simulink model "COMPONENT_MDL_Lag_QUAD_and_PEND_with_spin_rotors"  (R2020b)
(part 9 of 10)

Ly_pend.^2.*THE_Phi_D.*m_pend.*sin(THE_Phi_pend.*2.0).*(-1.0./2.4e+1)+(Lz_pend.^2.*THE_Phi_D.*m_pend.*sin(THE_Phi_pend.*2.0))./6.0-(Ly_pend.^2.*THE_Psi_D.*m_pend.*cos(THE_Theta).*sin(THE_Psi))./6.0-(Ly_pend.^2.*THE_Theta_pend_D.*m_pend.*cos(THE_Phi_pend).*sin(THE_Theta))./6.0-Lz_pend.^2.*THE_Theta_D.*m_pend.*cos(THE_Psi).*sin(THE_Theta).*(2.0./3.0)+(Ly_pend.^2.*THE_Phi_D.*m_pend.*cos(THE_Theta).*sin(THE_Psi).*sin(THE_Theta))./1.2e+1+(Ly_pend.^2.*THE_Psi_D.*m_pend.*cos(THE_Phi_pend).*sin(THE_Theta).*sin(THE_Phi_pend))./6.0+(Ly_pend.^2.*THE_Theta_pend_D.*m_pend.*cos(THE_Theta).*sin(THE_Psi).*sin(THE_Phi_pend))./6.0+(Ly_pend.^2.*THE_Phi_D.*m_pend.*cos(THE_Psi_pend).*sin(THE_Psi_pend).*sin(THE_Theta_pend))./1.2e+1-(Lz_pend.^2.*THE_Phi_D.*m_pend.*cos(THE_Theta).*sin(THE_Psi).*sin(THE_Theta))./3.0-Lz_pend.^2.*THE_Psi_D.*m_pend.*cos(THE_Phi_pend).*sin(THE_Theta).*sin(THE_Phi_pend).*(2.0./3.0)-(Lz_pend.^2.*THE_Phi_D.*m_pend.*cos(THE_Psi_pend).*sin(THE_Psi_pend).*sin(THE_Theta_pend))./3.0-Lz_pend.^2.*THE_Psi_pend_D.*m_pend.*cos(THE_Theta_pend).*sin(THE_Theta).*sin(THE_Phi_pend).*(2.0./3.0)-(Lx_pend.^2.*THE_Psi_D.*m_pend.*cos(THE_Theta).*cos(THE_Theta_pend).^2.*sin(THE_Psi))./6.0-(Lx_pend.^2.*THE_Phi_D.*m_pend.*cos(THE_Phi_pend).*cos(THE_Theta_pend).^2.*sin(THE_Phi_pend))./1.2e+1-(Lx_pend.^2.*THE_Theta_pend_D.*m_pend.*cos(THE_Phi_pend).*cos(THE_Theta_pend).^2.*sin(THE_Theta))./6.0+(Ly_pend.^2.*THE_Psi_D.*m_pend.*cos(THE_Theta).*cos(THE_Phi_pend).^2.*sin(THE_Psi))./6.0+(Ly_pend.^2.*THE_Psi_D.*m_pend.*cos(THE_Theta).*cos(THE_Psi_pend).^2.*sin(THE_Psi))./6.0-(Ly_pend.^2.*THE_Theta_D.*m_pend.*cos(THE_Psi).*cos(THE_Phi_pend).^2.*sin(THE_Theta))./6.0+(Ly_pend.^2.*THE_Psi_D.*m_pend.*cos(THE_Theta).*cos(THE_Theta_pend).^2.*sin(THE_Psi))./6.0-(Ly_pend.^2.*THE_Theta_D.*m_pend.*cos(THE_Psi).*cos(THE_Psi_pend).^2.*sin(THE_Theta))./6.0+(Ly_pend.^2.*THE_Phi_D.*m_pend.*cos(THE_Theta).^2.*cos(THE_Phi_pend).*sin(THE_Phi_pend))./6.0+(Ly_pend.^2.*THE_Phi_D.*m_pend.*cos(THE_Phi_pend).*cos(THE_Psi_pend).^2.*sin(THE_Phi_pend))./6.0+(Ly_pend.^2.*THE_Phi_D.*m_pend.*cos(THE_Phi_pend).*cos(THE_Theta_pend).^2.*sin(THE_Phi_pend))./1.2e+1+(Ly_pend.^2.*THE_Theta_pend_D.*m_pend.*cos(THE_Phi_pend).*cos(THE_Psi_pend).^2.*sin(THE_Theta))./6.0+(Ly_pend.^2.*THE_Theta_pend_D.*m_pend.*cos(THE_Phi_pend).*cos(THE_Theta_pend).^2.*sin(THE_Theta))./6.0-Lz_pend.^2.*THE_Psi_D.*m_pend.*cos(THE_Theta).*cos(THE_Phi_pend).^2.*sin(THE_Psi).*(2.0./3.0)-Lz_pend.^2.*THE_Psi_D.*m_pend.*cos(THE_Theta).*cos(THE_Psi_pend).^2.*sin(THE_Psi).*(2.0./3.0)+Lz_pend.^2.*THE_Theta_D.*m_pend.*cos(THE_Psi).*cos(THE_Phi_pend).^2.*sin(THE_Theta).*(2.0./3.0)+Lz_pend.^2.*THE_Theta_D.*m_pend.*cos(THE_Psi).*cos(THE_Psi_pend).^2.*sin(THE_Theta).*(2.0./3.0)-Lz_pend.^2.*THE_Phi_D.*m_pend.*cos(THE_Theta).^2.*cos(THE_Phi_pend).*sin(THE_Phi_pend).*(2.0./3.0)-Lz_pend.^2.*THE_Phi_D.*m_pend.*cos(THE_Phi_pend).*cos(THE_Psi_pend).^2.*sin(THE_Phi_pend).*(2.0./3.0)-Lz_pend.^2.*THE_Theta_pend_D.*m_pend.*cos(THE_Phi_pend).*cos(THE_Psi_pend).^2.*sin(THE_Theta).*(2.0./3.0)+(Lx_pend.^2.*THE_Phi_D.*m_pend.*cos(THE_Theta).*cos(THE_Theta_pend).^2.*sin(THE_Psi).*sin(THE_Theta))./1.2e+1+(Lx_pend.^2.*THE_Psi_D.*m_pend.*cos(THE_Phi_pend).*cos(THE_Theta_pend).^2.*sin(THE_Theta).*sin(THE_Phi_pend))./6.0+(Lx_pend.^2.*THE_Theta_pend_D.*m_pend.*cos(THE_Theta).*cos(THE_Theta_pend).^2.*sin(THE_Psi).*sin(THE_Phi_pend))./6.0-(Ly_pend.^2.*THE_Phi_D.*m_pend.*cos(THE_Theta).*cos(THE_Phi_pend).^2.*sin(THE_Psi).*sin(THE_Theta))./6.0-(Ly_pend.^2.*THE_Phi_D.*m_pend.*cos(THE_Theta).*cos(THE_Psi_pend).^2.*sin(THE_Psi).*sin(THE_Theta))./6.0-(Ly_pend.^2.*THE_Phi_D.*m_pend.*cos(THE_Theta).*cos(THE_Theta_pend).^2.*sin(THE_Psi).*sin(THE_Theta))./1.2e+1-(Ly_pend.^2.*THE_Psi_D.*m_pend.*cos(THE_Phi_pend).*cos(THE_Psi_pend).^2.*sin(THE_Theta).*sin(THE_Phi_pend))./3.0-(Ly_pend.^2.*THE_Psi_D.*m_pend.*cos(THE_Phi_pend).*cos(THE_Theta_pend).^2.*sin(THE_Theta).*sin(THE_Phi_pend))./6.0-(Ly_pend.^2.*THE_Phi_D.*m_pend.*cos(THE_Theta).^2.*cos(THE_Psi_pend).*sin(THE_Psi_pend).*sin(THE_Theta_pend))./6.0-(Ly_pend.^2.*THE_Theta_pend_D.*m_pend.*cos(THE_Theta).*cos(THE_Psi_pend).^2.*sin(THE_Psi).*sin(THE_Phi_pend))./6.0-(Ly_pend.^2.*THE_Theta_pend_D.*m_pend.*cos(THE_Theta).*cos(THE_Theta_pend).^2.*sin(THE_Psi).*sin(THE_Phi_pend))./6.0-(Ly_pend.^2.*THE_Phi_D.*m_pend.*cos(THE_Phi_pend).^2.*cos(THE_Psi_pend).*sin(THE_Psi_pend).*sin(THE_Theta_pend))./6.0-(Ly_pend.^2.*THE_Psi_pend_D.*m_pend.*cos(THE_Psi_pend).^2.*cos(THE_Theta_pend).*sin(THE_Theta).*sin(THE_Phi_pend))./6.0+Lz_pend.^2.*THE_Phi_D.*m_pend.*cos(THE_Theta).*cos(THE_Phi_pend).^2.*sin(THE_Psi).*sin(THE_Theta).*(2.0./3.0)+Lz_pend.^2.*THE_Phi_D.*m_pend.*cos(THE_Theta).*cos(THE_Psi_pend).^2.*sin(THE_Psi).*sin(THE_Theta).*(2.0./3.0)+Lz_pend.^2.*THE_Psi_D.*m_pend.*cos(THE_Phi_pend).*cos(THE_Psi_pend).^2.*sin(THE_Theta).*sin(THE_Phi_pend).*(4.0./3.0)+Lz_pend.^2.*THE_Phi_D.*m_pend.*cos(THE_Theta).^2.*cos(THE_Psi_pend).*sin(THE_Psi_pend).*sin(THE_Theta_pend).*(2.0./3.0)+Lz_pend.^2.*THE_Theta_pend_D.*m_pend.*cos(THE_Theta).*cos(THE_Psi_pend).^2.*sin(THE_Psi).*sin(THE_Phi_pend).*(2.0./3.0)+Lz_pend.^2.*THE_Phi_D.*m_pend.*cos(THE_Phi_pend).^2.*cos(THE_Psi_pend).*sin(THE_Psi_pend).*sin(THE_Theta_pend).*(2.0./3.0)+Lz_pend.^2.*THE_Psi_pend_D.*m_pend.*cos(THE_Psi_pend).^2.*cos(THE_Theta_pend).*sin(THE_Theta).*sin(THE_Phi_pend).*(2.0./3.0)+(Lx_pend.^2.*THE_Psi_D.*m_pend.*cos(THE_Theta).*cos(THE_Phi_pend).^2.*cos(THE_Theta_pend).^2.*sin(THE_Psi))./6.0-(Lx_pend.^2.*THE_Theta_D.*m_pend.*cos(THE_Psi).*cos(THE_Phi_pend).^2.*cos(THE_Theta_pend).^2.*sin(THE_Theta))./6.0+(Lx_pend.^2.*THE_Phi_D.*m_pend.*cos(THE_Theta).^2.*cos(THE_Phi_pend).*cos(THE_Theta_pend).^2.*sin(THE_Phi_pend))./6.0-(Ly_pend.^2.*THE_Phi_D.*m_pend.*cos(THE_Psi).^2.*cos(THE_Theta).^2.*cos(THE_Phi_pend).*sin(THE_Phi_pend))./1.2e+1-(Ly_pend.^2.*THE_Psi_D.*m_pend.*cos(THE_Theta).*cos(THE_Phi_pend).^2.*cos(THE_Psi_pend).^2.*sin(THE_Psi))./3.0-(Ly_pend.^2.*THE_Psi_D.*m_pend.*cos(THE_Theta).*cos(THE_Phi_pend).^2.*cos(THE_Theta_pend).^2.*sin(THE_Psi))./6.0+(Ly_pend.^2.*THE_Theta_D.*m_pend.*cos(THE_Psi).*cos(THE_Phi_pend).^2.*cos(THE_Psi_pend).^2.*sin(THE_Theta))./3.0-(Ly_pend.^2.*THE_Psi_D.*m_pend.*cos(THE_Theta).*cos(THE_Psi_pend).^2.*cos(THE_Theta_pend).^2.*sin(THE_Psi))./6.0+(Ly_pend.^2.*THE_Theta_D.*m_pend.*cos(THE_Psi).*cos(THE_Phi_pend).^2.*cos(THE_Theta_pend).^2.*sin(THE_Theta))./6.0-(Ly_pend.^2.*THE_Phi_D.*m_pend.*cos(THE_Theta).^2.*cos(THE_Phi_pend).*cos(THE_Psi_pend).^2.*sin(THE_Phi_pend))./3.0-(Ly_pend.^2.*THE_Phi_D.*m_pend.*cos(THE_Theta).^2.*cos(THE_Phi_pend).*cos(THE_Theta_pend).^2.*sin(THE_Phi_pend))./6.0-(Ly_pend.^2.*THE_Phi_D.*m_pend.*cos(THE_Phi_pend).*cos(THE_Psi_pend).^2.*cos(THE_Theta_pend).^2.*sin(THE_Phi_pend))./1.2e+1-(Ly_pend.^2.*THE_Theta_pend_D.*m_pend.*cos(THE_Phi_pend).*cos(THE_Psi_pend).^2.*cos(THE_Theta_pend).^2.*sin(THE_Theta))./6.0+(Lz_pend.^2.*THE_Phi_D.*m_pend.*cos(THE_Psi).^2.*cos(THE_Theta).^2.*cos(THE_Phi_pend).*sin(THE_Phi_pend))./3.0+Lz_pend.^2.*THE_Psi_D.*m_pend.*cos(THE_Theta).*cos(THE_Phi_pend).^2.*cos(THE_Psi_pend).^2.*sin(THE_Psi).*(4.0./3.0)-Lz_pend.^2.*THE_Theta_D.*m_pend.*cos(THE_Psi).*cos(THE_Phi_pend).^2.*cos(THE_Psi_pend).^2.*sin(THE_Theta).*(4.0./3.0)+Lz_pend.^2.*THE_Psi_D.*m_pend.*cos(THE_Theta).*cos(THE_Psi_pend).^2.*cos(THE_Theta_pend).^2.*sin(THE_Psi).*(2.0./3.0)+Lz_pend.^2.*THE_Phi_D.*m_pend.*cos(THE_Theta).^2.*cos(THE_Phi_pend).*cos(THE_Psi_pend).^2.*sin(THE_Phi_pend).*(4.0./3.0)+(Lz_pend.^2.*THE_Phi_D.*m_pend.*cos(THE_Phi_pend).*cos(THE_Psi_pend).^2.*cos(THE_Theta_pend).^2.*sin(THE_Phi_pend))./3.0+Lz_pend.^2.*THE_Theta_pend_D.*m_pend.*cos(THE_Phi_pend).*cos(THE_Psi_pend).^2.*cos(THE_Theta_pend).^2.*sin(THE_Theta).*(2.0./3.0)-(Lx_pend.^2.*THE_Theta_pend_D.*m_pend.*cos(THE_Psi).*cos(THE_Theta).*cos(THE_Theta_pend).*sin(THE_Theta_pend))./6.0+(Ly_pend.^2.*THE_Theta_pend_D.*m_pend.*cos(THE_Psi).*cos(THE_Theta).*cos(THE_Theta_pend).*sin(THE_Theta_pend))./6.0-Lz_pend.^2.*THE_Psi_pend_D.*m_pend.*cos(THE_Theta).*cos(THE_Phi_pend).*cos(THE_Theta_pend).*sin(THE_Psi).*(2.0./3.0)-(Ly_pend.^2.*THE_Psi_D.*m_pend.*cos(THE_Psi_pend).*sin(THE_Theta).*sin(THE_Psi_pend).*sin(THE_Theta_pend))./6.0+Lz_pend.^2.*THE_Psi_D.*m_pend.*cos(THE_Psi_pend).*sin(THE_Theta).*sin(THE_Psi_pend).*sin(THE_Theta_pend).*(2.0./3.0)+Lz_pend.*THE_Theta_D.*Tv_Z_pend.*m_pend.*cos(THE_Psi).^2.*cos(THE_Theta).*sin(THE_Phi_pend).*sin(THE_Psi_pend)-(Lx_pend.^2.*THE_Phi_D.*m_pend.*cos(THE_Theta).*cos(THE_Phi_pend).^2.*cos(THE_Theta_pend).^2.*sin(THE_Psi).*sin(THE_Theta))./6.0+(Ly_pend.^2.*THE_Phi_D.*m_pend.*cos(THE_Theta).*cos(THE_Phi_pend).^2.*cos(THE_Psi_pend).^2.*sin(THE_Psi).*sin(THE_Theta))./3.0+(Ly_pend.^2.*THE_Phi_D.*m_pend.*cos(THE_Theta).*cos(THE_Phi_pend).^2.*cos(THE_Theta_pend).^2.*sin(THE_Psi).*sin(THE_Theta))./6.0+(Ly_pend.^2.*THE_Phi_D.*m_pend.*cos(THE_Theta).*cos(THE_Psi_pend).^2.*cos(THE_Theta_pend).^2.*sin(THE_Psi).*sin(THE_Theta))./1.2e+1+(Ly_pend.^2.*THE_Phi_D.*m_pend.*cos(THE_Psi).^2.*cos(THE_Theta).^2.*cos(THE_Psi_pend).*sin(THE_Psi_pend).*sin(THE_Theta_pend))./1.2e+1+(Ly_pend.^2.*THE_Phi_D.*m_pend.*cos(THE_Theta).^2.*cos(THE_Phi_pend).^2.*cos(THE_Psi_pend).*sin(THE_Psi_pend).*sin(THE_Theta_pend))./3.0+(Ly_pend.^2.*THE_Psi_D.*m_pend.*cos(THE_Phi_pend).*cos(THE_Psi_pend).^2.*cos(THE_Theta_pend).^2.*sin(THE_Theta).*sin(THE_Phi_pend))./6.0+(Ly_pend.^2.*THE_Theta_pend_D.*m_pend.*cos(THE_Theta).*cos(THE_Psi_pend).^2.*cos(THE_Theta_pend).^2.*sin(THE_Psi).*sin(THE_Phi_pend))./6.0-Lz_pend.^2.*THE_Phi_D.*m_pend.*cos(THE_Theta).*cos(THE_Phi_pend).^2.*cos(THE_Psi_pend).^2.*sin(THE_Psi).*sin(THE_Theta).*(4.0./3.0)-(Lz_pend.^2.*THE_Phi_D.*m_pend.*cos(THE_Theta).*cos(THE_Psi_pend).^2.*cos(THE_Theta_pend).^2.*sin(THE_Psi).*sin(THE_Theta))./3.0-(Lz_pend.^2.*THE_Phi_D.*m_pend.*cos(THE_Psi).^2.*cos(THE_Theta).^2.*cos(THE_Psi_pend).*sin(THE_Psi_pend).*sin(THE_Theta_pend))./3.0-Lz_pend.^2.*THE_Phi_D.*m_pend.*cos(THE_Theta).^2.*cos(THE_Phi_pend).^2.*cos(THE_Psi_pend).*sin(THE_Psi_pend).*sin(THE_Theta_pend).*(4.0./3.0)-Lz_pend.^2.*THE_Psi_D.*m_pend.*cos(THE_Phi_pend).*cos(THE_Psi_pend).^2.*cos(THE_Theta_pend).^2.*sin(THE_Theta).*sin(THE_Phi_pend).*(2.0./3.0)-Lz_pend.^2.*THE_Theta_pend_D.*m_pend.*cos(THE_Theta).*cos(THE_Psi_pend).^2.*cos(THE_Theta_pend).^2.*sin(THE_Psi).*sin(THE_Phi_pend).*(2.0./3.0)+(Lx_pend.^2.*THE_Psi_D.*m_pend.*cos(THE_Psi).*cos(THE_Theta).*cos(THE_Theta_pend).*sin(THE_Phi_pend).*sin(THE_Theta_pend))./6.0+(Ly_pend.^2.*THE_Theta_D.*m_pend.*cos(THE_Psi).*cos(THE_Theta).*cos(THE_Phi_pend).*sin(THE_Psi).*sin(THE_Phi_pend))./6.0-(Ly_pend.^2.*THE_Psi_D.*m_pend.*cos(THE_Psi).*cos(THE_Theta).*cos(THE_Theta_pend).*sin(THE_Phi_pend).*sin(THE_Theta_pend))./6.0-Lz_pend.^2.*THE_Theta_D.*m_pend.*cos(THE_Psi).*cos(THE_Theta).*cos(THE_Phi_pend).*sin(THE_Psi).*sin(THE_Phi_pend).*(2.0./3.0)-(Lx_pend.^2.*THE_Phi_D.*m_pend.*cos(THE_Psi).^2.*cos(THE_Theta).^2.*cos(THE_Phi_pend).*cos(THE_Theta_pend).^2.*sin(THE_Phi_pend))./1.2e+1+(Ly_pend.^2.*THE_Phi_D.*m_pend.*cos(THE_Psi).^2.*cos(THE_Theta).^2.*cos(THE_Phi_pend).*cos(THE_Psi_pend).^2.*sin(THE_Phi_pend))./6.0+(Ly_pend.^2.*THE_Phi_D.*m_pend.*cos(THE_Psi).^2.*cos(THE_Theta).^2.*cos(THE_Phi_pend).*cos(THE_Theta_pend).^2.*sin(THE_Phi_pend))./1.2e+1+(Ly_pend.^2.*THE_Psi_D.*m_pend.*cos(THE_Theta).*cos(THE_Phi_pend).^2.*cos(THE_Psi_pend).^2.*cos(THE_Theta_pend).^2.*sin(THE_Psi))./6.0-(Ly_pend.^2.*THE_Theta_D.*m_pend.*cos(THE_Psi).*cos(THE_Phi_pend).^2.*cos(THE_Psi_pend).^2.*cos(THE_Theta_pend).^2.*sin(THE_Theta))./6.0+(Ly_pend.^2.*THE_Phi_D.*m_pend.*cos(THE_Theta).^2.*cos(THE_Phi_pend).*cos(THE_Psi_pend).^2.*cos(THE_Theta_pend).^2.*sin(THE_Phi_pend))./6.0-Lz_pend.^2.*THE_Phi_D.*m_pend.*cos(THE_Psi).^2.*cos(THE_Theta).^2.*cos(THE_Phi_pend).*cos(THE_Psi_pend).^2.*sin(THE_Phi_pend).*(2.0./3.0)-Lz_pend.^2.*THE_Psi_D.*m_pend.*cos(THE_Theta).*cos(THE_Phi_pend).^2.*cos(THE_Psi_pend).^2.*cos(THE_Theta_pend).^2.*sin(THE_Psi).*(2.0./3.0)+Lz_pend.^2.*THE_Theta_D.*m_pend.*cos(THE_Psi).*cos(THE_Phi_pend).^2.*cos(THE_Psi_pend).^2.*cos(THE_Theta_pend).^2.*sin(THE_Theta).*(2.0./3.0)-Lz_pend.^2.*THE_Phi_D.*m_pend.*cos(THE_Theta).^2.*cos(THE_Phi_pend).*cos(THE_Psi_pend).^2.*cos(THE_Theta_pend).^2.*sin(THE_Phi_pend).*(2.0./3.0)+(Ly_pend.^2.*THE_Theta_pend_D.*m_pend.*cos(THE_Psi_pend).*sin(THE_Theta).*sin(THE_Phi_pend).*sin(THE_Psi_pend).*sin(THE_Theta_pend))./6.0-Lz_pend.^2.*THE_Theta_pend_D.*m_pend.*cos(THE_Psi_pend).*sin(THE_Theta).*sin(THE_Phi_pend).*sin(THE_Psi_pend).*sin(THE_Theta_pend).*(2.0./3.0)+Lz_pend.*THE_Psi_D.*Tv_Z_pend.*m_pend.*cos(THE_Psi).*cos(THE_Theta).*cos(THE_Phi_pend).*sin(THE_Psi_pend)-(Lx_pend.^2.*THE_Theta_D.*m_pend.*cos(THE_Psi).^2.*cos(THE_Theta).*cos(THE_Phi_pend).*cos(THE_Theta_pend).*sin(THE_Theta_pend))./6.0+(Ly_pend.^2.*THE_Theta_D.*m_pend.*cos(THE_Psi).^2.*cos(THE_Theta).*cos(THE_Phi_pend).*cos(THE_Theta_pend).*sin(THE_Theta_pend))./6.0-(Ly_pend.^2.*THE_Psi_pend_D.*m_pend.*cos(THE_Theta).*cos(THE_Phi_pend).*cos(THE_Psi_pend).^2.*cos(THE_Theta_pend).*sin(THE_Psi))./6.0-(Ly_pend.^2.*THE_Psi_pend_D.*m_pend.*cos(THE_Psi).*cos(THE_Theta).*cos(THE_Psi_pend).*cos(THE_Theta_pend).^2.*sin(THE_Psi_pend))./6.0-(Ly_pend.^2.*THE_Theta_pend_D.*m_pend.*cos(THE_Psi).*cos(THE_Theta).*cos(THE_Psi_pend).^2.*cos(THE_Theta_pend).*sin(THE_Theta_pend))./6.0+Lz_pend.^2.*THE_Psi_pend_D.*m_pend.*cos(THE_Theta).*cos(THE_Phi_pend).*cos(THE_Psi_pend).^2.*cos(THE_Theta_pend).*sin(THE_Psi).*(2.0./3.0)+Lz_pend.^2.*THE_Psi_pend_D.*m_pend.*cos(THE_Psi).*cos(THE_Theta).*cos(THE_Psi_pend).*cos(THE_Theta_pend).^2.*sin(THE_Psi_pend).*(2.0./3.0)+Lz_pend.^2.*THE_Theta_pend_D.*m_pend.*cos(THE_Psi).*cos(THE_Theta).*cos(THE_Psi_pend).^2.*cos(THE_Theta_pend).*sin(THE_Theta_pend).*(2.0./3.0)+(Ly_pend.^2.*THE_Psi_D.*m_pend.*cos(THE_Phi_pend).^2.*cos(THE_Psi_pend).*sin(THE_Theta).*sin(THE_Psi_pend).*sin(THE_Theta_pend))./3.0-Lz_pend.^2.*THE_Psi_D.*m_pend.*cos(THE_Phi_pend).^2.*cos(THE_Psi_pend).*sin(THE_Theta).*sin(THE_Psi_pend).*sin(THE_Theta_pend).*(4.0./3.0)-(Ly_pend.^2.*THE_Psi_D.*m_pend.*cos(THE_Psi).*cos(THE_Theta).*cos(THE_Phi_pend).*cos(THE_Psi_pend).*cos(THE_Theta_pend).*sin(THE_Psi_pend))./6.0+Lz_pend.^2.*THE_Psi_D.*m_pend.*cos(THE_Psi).*cos(THE_Theta).*cos(THE_Phi_pend).*cos(THE_Psi_pend).*cos(THE_Theta_pend).*sin(THE_Psi_pend).*(2.0./3.0)-(Lx_pend.^2.*THE_Phi_D.*m_pend.*cos(THE_Psi).*cos(THE_Theta).*cos(THE_Theta_pend).*sin(THE_Theta).*sin(THE_Phi_pend).*sin(THE_Theta_pend))./1.2e+1-(Ly_pend.^2.*THE_Theta_D.*m_pend.*cos(THE_Psi).*cos(THE_Theta).*cos(THE_Psi_pend).*sin(THE_Psi).*sin(THE_Psi_pend).*sin(THE_Theta_pend))./6.0+(Ly_pend.^2.*THE_Phi_D.*m_pend.*cos(THE_Psi).*cos(THE_Theta).*cos(THE_Theta_pend).*sin(THE_Theta).*sin(THE_Phi_pend).*sin(THE_Theta_pend))./1.2e+1+(Ly_pend.^2.*THE_Theta_pend_D.*m_pend.*cos(THE_Theta).*cos(THE_Phi_pend).*cos(THE_Psi_pend).*sin(THE_Psi).*sin(THE_Psi_pend).*sin(THE_Theta_pend))./6.0+(Ly_pend.^2.*THE_Psi_pend_D.*m_pend.*cos(THE_Phi_pend).*cos(THE_Psi_pend).*cos(THE_Theta_pend).*sin(THE_Theta).*sin(THE_Psi_pend).*sin(THE_Theta_pend))./6.0+Lz_pend.^2.*THE_Theta_D.*m_pend.*cos(THE_Psi).*cos(THE_Theta).*cos(THE_Psi_pend).*sin(THE_Psi).*sin(THE_Psi_pend).*sin(THE_Theta_pend).*(2.0./3.0)-Lz_pend.^2.*THE_Theta_pend_D.*m_pend.*cos(THE_Theta).*cos(THE_Phi_pend).*cos(THE_Psi_pend).*sin(THE_Psi).*sin(THE_Psi_pend).*sin(THE_Theta_pend).*(2.0./3.0)-Lz_pend.^2.*THE_Psi_pend_D.*m_pend.*cos(THE_Phi_pend).*cos(THE_Psi_pend).*cos(THE_Theta_pend).*sin(THE_Theta).*sin(THE_Psi_pend).*sin(THE_Theta_pend).*(2.0./3.0)-(Ly_pend.^2.*THE_Phi_D.*m_pend.*cos(THE_Theta).*cos(THE_Phi_pend).^2.*cos(THE_Psi_pend).^2.*cos(THE_Theta_pend).^2.*sin(THE_Psi).*sin(THE_Theta))./6.0-(Ly_pend.^2.*THE_Phi_D.*m_pend.*cos(THE_Psi).^2.*cos(THE_Theta).^2.*cos(THE_Phi_pend).^2.*cos(THE_Psi_pend).*sin(THE_Psi_pend).*sin(THE_Theta_pend))./6.0+Lz_pend.^2.*THE_Phi_D.*m_pend.*cos(THE_Theta).*cos(THE_Phi_pend).^2.*cos(THE_Psi_pend).^2.*cos(THE_Theta_pend).^2.*sin(THE_Psi).*sin(THE_Theta).*(2.0./3.0)+Lz_pend.^2.*THE_Phi_D.*m_pend.*cos(THE_Psi).^2.*cos(THE_Theta).^2.*cos(THE_Phi_pend).^2.*cos(THE_Psi_pend).*sin(THE_Psi_pend).*sin(THE_Theta_pend).*(2.0./3.0)-(Lz_pend.*THE_Phi_D.*Tv_Z_pend.*m_pend.*cos(THE_Psi).*cos(THE_Theta).*cos(THE_Phi_pend).*sin(THE_Theta).*sin(THE_Psi_pend))./2.0-Lz_pend.*THE_Psi_D.*Tv_Z_pend.*m_pend.*cos(THE_Psi).*cos(THE_Theta).*cos(THE_Psi_pend).*sin(THE_Phi_pend).*sin(THE_Theta_pend)-(Lx_pend.^2.*THE_Phi_D.*m_pend.*cos(THE_Psi).*cos(THE_Theta).^2.*cos(THE_Phi_pend).*cos(THE_Theta_pend).*sin(THE_Psi).*sin(THE_Theta_pend))./1.2e+1+(Lx_pend.^2.*THE_Theta_D.*m_pend.*cos(THE_Psi).*cos(THE_Theta).*cos(THE_Phi_pend).*cos(THE_Theta_pend).^2.*sin(THE_Psi).*sin(THE_Phi_pend))./6.0-(Ly_pend.^2.*THE_Theta_D.*m_pend.*cos(THE_Psi).*cos(THE_Theta).*cos(THE_Phi_pend).*cos(THE_Psi_pend).^2.*sin(THE_Psi).*sin(THE_Phi_pend))./3.0+(Ly_pend.^2.*THE_Phi_D.*m_pend.*cos(THE_Psi).*cos(THE_Theta).^2.*cos(THE_Phi_pend).*cos(THE_Theta_pend).*sin(THE_Psi).*sin(THE_Theta_pend))./1.2e+1-(Ly_pend.^2.*THE_Theta_D.*m_pend.*cos(THE_Psi).*cos(THE_Theta).*cos(THE_Phi_pend).*cos(THE_Theta_pend).^2.*sin(THE_Psi).*sin(THE_Phi_pend))./6.0+(Ly_pend.^2.*THE_Psi_D.*m_pend.*cos(THE_Psi).*cos(THE_Theta).*cos(THE_Psi_pend).^2.*cos(THE_Theta_pend).*sin(THE_Phi_pend).*sin(THE_Theta_pend))./6.0-(Ly_pend.^2.*THE_Theta_D.*m_pend.*cos(THE_Psi).^2.*cos(THE_Theta).*cos(THE_Psi_pend).*cos(THE_Theta_pend).*sin(THE_Phi_pend).*sin(THE_Psi_pend))./6.0+Lz_pend.^2.*THE_Theta_D.*m_pend.*cos(THE_Psi).*cos(THE_Theta).*cos(THE_Phi_pend).*cos(THE_Psi_pend).^2.*sin(THE_Psi).*sin(THE_Phi_pend).*(4.0./3.0)-Lz_pend.^2.*THE_Psi_D.*m_pend.*cos(THE_Psi).*cos(THE_Theta).*cos(THE_Psi_pend).^2.*cos(THE_Theta_pend).*sin(THE_Phi_pend).*sin(THE_Theta_pend).*(2.0./3.0)+Lz_pend.^2.*THE_Theta_D.*m_pend.*cos(THE_Psi).^2.*cos(THE_Theta).*cos(THE_Psi_pend).*cos(THE_Theta_pend).*sin(THE_Phi_pend).*sin(THE_Psi_pend).*(2.0./3.0)-(Ly_pend.^2.*THE_Phi_D.*m_pend.*cos(THE_Psi).^2.*cos(THE_Theta).^2.*cos(THE_Phi_pend).*cos(THE_Psi_pend).^2.*cos(THE_Theta_pend).^2.*sin(THE_Phi_pend))./1.2e+1+(Lz_pend.^2.*THE_Phi_D.*m_pend.*cos(THE_Psi).^2.*cos(THE_Theta).^2.*cos(THE_Phi_pend).*cos(THE_Psi_pend).^2.*cos(THE_Theta_pend).^2.*sin(THE_Phi_pend))./3.0+Lz_pend.*THE_Theta_D.*Tv_Z_pend.*m_pend.*cos(THE_Psi).^2.*cos(THE_Theta).*cos(THE_Phi_pend).*cos(THE_Psi_pend).*sin(THE_Theta_pend)+(Lz_pend.*THE_Phi_D.*Tv_Z_pend.*m_pend.*cos(THE_Psi).*cos(THE_Theta).^2.*sin(THE_Psi).*sin(THE_Phi_pend).*sin(THE_Psi_pend))./2.0-(Ly_pend.^2.*THE_Theta_D.*m_pend.*cos(THE_Psi).^2.*cos(THE_Theta).*cos(THE_Phi_pend).*cos(THE_Psi_pend).^2.*cos(THE_Theta_pend).*sin(THE_Theta_pend))./6.0+Lz_pend.^2.*THE_Theta_D.*m_pend.*cos(THE_Psi).^2.*cos(THE_Theta).*cos(THE_Phi_pend).*cos(THE_Psi_pend).^2.*cos(THE_Theta_pend).*sin(THE_Theta_pend).*(2.0./3.0)-(Ly_pend.^2.*THE_Psi_D.*m_pend.*cos(THE_Theta).*cos(THE_Phi_pend).*cos(THE_Psi_pend).*sin(THE_Psi).*sin(THE_Phi_pend).*sin(THE_Psi_pend).*sin(THE_Theta_pend))./3.0+(Ly_pend.^2.*THE_Theta_D.*m_pend.*cos(THE_Psi).*cos(THE_Phi_pend).*cos(THE_Psi_pend).*sin(THE_Theta).*sin(THE_Phi_pend).*sin(THE_Psi_pend).*sin(THE_Theta_pend))./3.0-(Ly_pend.^2.*THE_Psi_pend_D.*m_pend.*cos(THE_Theta).*cos(THE_Psi_pend).*cos(THE_Theta_pend).*sin(THE_Psi).*sin(THE_Phi_pend).*sin(THE_Psi_pend).*sin(THE_Theta_pend))./6.0+Lz_pend.^2.*THE_Psi_D.*m_pend.*cos(THE_Theta).*cos(THE_Phi_pend).*cos(THE_Psi_pend).*sin(THE_Psi).*sin(THE_Phi_pend).*sin(THE_Psi_pend).*sin(THE_Theta_pend).*(4.0./3.0)-Lz_pend.^2.*THE_Theta_D.*m_pend.*cos(THE_Psi).*cos(THE_Phi_pend).*cos(THE_Psi_pend).*sin(THE_Theta).*sin(THE_Phi_pend).*sin(THE_Psi_pend).*sin(THE_Theta_pend).*(4.0./3.0)+Lz_pend.^2.*THE_Psi_pend_D.*m_pend.*cos(THE_Theta).*cos(THE_Psi_pend).*cos(THE_Theta_pend).*sin(THE_Psi).*sin(THE_Phi_pend).*sin(THE_Psi_pend).*sin(THE_Theta_pend).*(2.0./3.0)+(Lz_pend.*THE_Phi_D.*Tv_Z_pend.*m_pend.*cos(THE_Psi).*cos(THE_Theta).*cos(THE_Psi_pend).*sin(THE_Theta).*sin(THE_Phi_pend).*sin(THE_Theta_pend))./2.0-(Ly_pend.^2.*THE_Phi_D.*m_pend.*cos(THE_Psi).*cos(THE_Theta).^2.*cos(THE_Psi_pend).*cos(THE_Theta_pend).*sin(THE_Psi).*sin(THE_Phi_pend).*sin(THE_Psi_pend))./1.2e+1+(Ly_pend.^2.*THE_Theta_D.*m_pend.*cos(THE_Psi).*cos(THE_Theta).*cos(THE_Phi_pend).^2.*cos(THE_Psi_pend).*sin(THE_Psi).*sin(THE_Psi_pend).*sin(THE_Theta_pend))./3.0-(Ly_pend.^2.*THE_Phi_D.*m_pend.*cos(THE_Psi).*cos(THE_Theta).*cos(THE_Psi_pend).^2.*cos(THE_Theta_pend).*sin(THE_Theta).*sin(THE_Phi_pend).*sin(THE_Theta_pend))./1.2e+1+(Lz_pend.^2.*THE_Phi_D.*m_pend.*cos(THE_Psi).*cos(THE_Theta).^2.*cos(THE_Psi_pend).*cos(THE_Theta_pend).*sin(THE_Psi).*sin(THE_Phi_pend).*sin(THE_Psi_pend))./3.0-Lz_pend.^2.*THE_Theta_D.*m_pend.*cos(THE_Psi).*cos(THE_Theta).*cos(THE_Phi_pend).^2.*cos(THE_Psi_pend).*sin(THE_Psi).*sin(THE_Psi_pend).*sin(THE_Theta_pend).*(4.0./3.0)+(Lz_pend.^2.*THE_Phi_D.*m_pend.*cos(THE_Psi).*cos(THE_Theta).*cos(THE_Psi_pend).^2.*cos(THE_Theta_pend).*sin(THE_Theta).*sin(THE_Phi_pend).*sin(THE_Theta_pend))./3.0+(Lz_pend.*THE_Phi_D.*Tv_Z_pend.*m_pend.*cos(THE_Psi).*cos(THE_Theta).^2.*cos(THE_Phi_pend).*cos(THE_Psi_pend).*sin(THE_Psi).*sin(THE_Theta_pend))./2.0-(Ly_pend.^2.*THE_Phi_D.*m_pend.*cos(THE_Psi).*cos(THE_Theta).^2.*cos(THE_Phi_pend).*cos(THE_Psi_pend).^2.*cos(THE_Theta_pend).*sin(THE_Psi).*sin(THE_Theta_pend))./1.2e+1+(Ly_pend.^2.*THE_Theta_D.*m_pend.*cos(THE_Psi).*cos(THE_Theta).*cos(THE_Phi_pend).*cos(THE_Psi_pend).^2.*cos(THE_Theta_pend).^2.*sin(THE_Psi).*sin(THE_Phi_pend))./6.0+(Lz_pend.^2.*THE_Phi_D.*m_pend.*cos(THE_Psi).*cos(THE_Theta).^2.*cos(THE_Phi_pend).*cos(THE_Psi_pend).^2.*cos(THE_Theta_pend).*sin(THE_Psi).*sin(THE_Theta_pend))./3.0-Lz_pend.^2.*THE_Theta_D.*m_pend.*cos(THE_Psi).*cos(THE_Theta).*cos(THE_Phi_pend).*cos(THE_Psi_pend).^2.*cos(THE_Theta_pend).^2.*sin(THE_Psi).*sin(THE_Phi_pend).*(2.0./3.0)+(Ly_pend.^2.*THE_Phi_D.*m_pend.*cos(THE_Psi).*cos(THE_Theta).*cos(THE_Phi_pend).*cos(THE_Psi_pend).*cos(THE_Theta_pend).*sin(THE_Theta).*sin(THE_Psi_pend))./1.2e+1-(Lz_pend.^2.*THE_Phi_D.*m_pend.*cos(THE_Psi).*cos(THE_Theta).*cos(THE_Phi_pend).*cos(THE_Psi_pend).*cos(THE_Theta_pend).*sin(THE_Theta).*sin(THE_Psi_pend))./3.0+(Ly_pend.^2.*THE_Phi_D.*m_pend.*cos(THE_Theta).*cos(THE_Phi_pend).*cos(THE_Psi_pend).*sin(THE_Psi).*sin(THE_Theta).*sin(THE_Phi_pend).*sin(THE_Psi_pend).*sin(THE_Theta_pend))./3.0-Lz_pend.^2.*THE_Phi_D.*m_pend.*cos(THE_Theta).*cos(THE_Phi_pend).*cos(THE_Psi_pend).*sin(THE_Psi).*sin(THE_Theta).*sin(THE_Phi_pend).*sin(THE_Psi_pend).*sin(THE_Theta_pend).*(4.0./3.0),(Ly_pend.^2.*THE_Theta_D.*m_pend.*cos(THE_Theta).*sin(THE_Phi_pend))./6.0+(Ly_pend.^2.*THE_Phi_pend_D.*m_pend.*cos(THE_Phi_pend).*sin(THE_Theta))./6.0-(Ly_pend.^2.*THE_Theta_D.*m_pend.*cos(THE_Phi_pend).*sin(THE_Psi).*sin(THE_Theta))./6.0-(Ly_pend.^2.*THE_Phi_pend_D.*m_pend.*cos(THE_Theta).*sin(THE_Psi).*sin(THE_Phi_pend))./6.0-(Ly_pend.^2.*THE_Psi_pend_D.*m_pend.*cos(THE_Phi_pend).*sin(THE_Theta).*sin(THE_Theta_pend))./6.0+(Lz_pend.*THE_Phi_D.*Tv_Z_pend.*m_pend.*cos(THE_Psi_pend).*sin(THE_Theta_pend))./2.0+(Lx_pend.^2.*THE_Theta_D.*m_pend.*cos(THE_Psi).^2.*cos(THE_Theta).*sin(THE_Phi_pend))./6.0-(Lx_pend.^2.*THE_Phi_D.*m_pend.*cos(THE_Theta).^2.*cos(THE_Theta_pend).*sin(THE_Theta_pend))./1.2e+1+(Lx_pend.^2.*THE_Theta_D.*m_pend.*cos(THE_Theta).*cos(THE_Theta_pend).^2.*sin(THE_Phi_pend))./6.0-(Lx_pend.^2.*THE_Phi_D.*m_pend.*cos(THE_Phi_pend).^2.*cos(THE_Theta_pend).*sin(THE_Theta_pend))./1.2e+1+(Lx_pend.^2.*THE_Phi_pend_D.*m_pend.*cos(THE_Phi_pend).*cos(THE_Theta_pend).^2.*sin(THE_Theta))./6.0-(Ly_pend.^2.*THE_Theta_D.*m_pend.*cos(THE_Psi).^2.*cos(THE_Theta).*sin(THE_Phi_pend))./6.0-(Ly_pend.^2.*THE_Theta_D.*m_pend.*cos(THE_Theta).*cos(THE_Psi_pend).^2.*sin(THE_Phi_pend))./6.0+(Ly_pend.^2.*THE_Phi_D.*m_pend.*cos(THE_Theta).^2.*cos(THE_Theta_pend).*sin(THE_Theta_pend))./1.2e+1-(Ly_pend.^2.*THE_Theta_D.*m_pend.*cos(THE_Theta).*cos(THE_Theta_pend).^2.*sin(THE_Phi_pend))./6.0-(Ly_pend.^2.*THE_Phi_pend_D.*m_pend.*cos(THE_Phi_pend).*cos(THE_Psi_pend).^2.*sin(THE_Theta))./6.0+(Ly_pend.^2.*THE_Phi_D.*m_pend.*cos(THE_Phi_pend).^2.*cos(THE_Theta_pend).*sin(THE_Theta_pend))./1.2e+1-(Ly_pend.^2.*THE_Phi_pend_D.*m_pend.*cos(THE_Phi_pend).*cos(THE_Theta_pend).^2.*sin(THE_Theta))./6.0+Lz_pend.^2.*THE_Theta_D.*m_pend.*cos(THE_Theta).*cos(THE_Psi_pend).^2.*sin(THE_Phi_pend).*(2.0./3.0)+Lz_pend.^2.*THE_Phi_pend_D.*m_pend.*cos(THE_Phi_pend).*cos(THE_Psi_pend).^2.*sin(THE_Theta).*(2.0./3.0)+(Lx_pend.^2.*THE_Psi_D.*m_pend.*cos(THE_Psi).*cos(THE_Theta).*cos(THE_Phi_pend))./6.0+(Ly_pend.^2.*THE_Psi_pend_D.*m_pend.*cos(THE_Psi).*cos(THE_Theta).*cos(THE_Theta_pend))./6.0-Lz_pend.*THE_Psi_D.*Tv_Z_pend.*m_pend.*cos(THE_Psi_pend).*sin(THE_Theta).*sin(THE_Theta_pend)-(Lx_pend.^2.*THE_Psi_D.*m_pend.*cos(THE_Psi).*cos(THE_Theta).*cos(THE_Phi_pend).*cos(THE_Theta_pend).^2)./6.0+(Ly_pend.^2.*THE_Psi_D.*m_pend.*cos(THE_Psi).*cos(THE_Theta).*cos(THE_Phi_pend).*cos(THE_Theta_pend).^2)./6.0-(Ly_pend.^2.*THE_Psi_pend_D.*m_pend.*cos(THE_Psi).*cos(THE_Theta).*cos(THE_Psi_pend).^2.*cos(THE_Theta_pend))./6.0+Lz_pend.^2.*THE_Psi_pend_D.*m_pend.*cos(THE_Psi).*cos(THE_Theta).*cos(THE_Psi_pend).^2.*cos(THE_Theta_pend).*(2.0./3.0)+(Lx_pend.^2.*THE_Phi_D.*m_pend.*cos(THE_Psi).*cos(THE_Theta).^2.*sin(THE_Psi).*sin(THE_Phi_pend))./1.2e+1-(Lx_pend.^2.*THE_Theta_D.*m_pend.*cos(THE_Phi_pend).*cos(THE_Theta_pend).^2.*sin(THE_Psi).*sin(THE_Theta))./6.0-(Lx_pend.^2.*THE_Phi_pend_D.*m_pend.*cos(THE_Theta).*cos(THE_Theta_pend).^2.*sin(THE_Psi).*sin(THE_Phi_pend))./6.0+(Lx_pend.^2.*THE_Psi_D.*m_pend.*cos(THE_Phi_pend).^2.*cos(THE_Theta_pend).*sin(THE_Theta).*sin(THE_Theta_pend))./6.0-(Ly_pend.^2.*THE_Phi_D.*m_pend.*cos(THE_Psi).*cos(THE_Theta).^2.*sin(THE_Psi).*sin(THE_Phi_pend))./1.2e+1+(Ly_pend.^2.*THE_Theta_D.*m_pend.*cos(THE_Phi_pend).*cos(THE_Psi_pend).^2.*sin(THE_Psi).*sin(THE_Theta))./6.0+(Ly_pend.^2.*THE_Theta_D.*m_pend.*cos(THE_Phi_pend).*cos(THE_Theta_pend).^2.*sin(THE_Psi).*sin(THE_Theta))./6.0+(Ly_pend.^2.*THE_Phi_pend_D.*m_pend.*cos(THE_Theta).*cos(THE_Psi_pend).^2.*sin(THE_Psi).*sin(THE_Phi_pend))./6.0+(Ly_pend.^2.*THE_Phi_pend_D.*m_pend.*cos(THE_Theta).*cos(THE_Theta_pend).^2.*sin(THE_Psi).*sin(THE_Phi_pend))./6.0-(Ly_pend.^2.*THE_Psi_D.*m_pend.*cos(THE_Phi_pend).^2.*cos(THE_Theta_pend).*sin(THE_Theta).*sin(THE_Theta_pend))./6.0+(Ly_pend.^2.*THE_Psi_pend_D.*m_pend.*cos(THE_Phi_pend).*cos(THE_Psi_pend).^2.*sin(THE_Theta).*sin(THE_Theta_pend))./6.0-Lz_pend.^2.*THE_Theta_D.*m_pend.*cos(THE_Phi_pend).*cos(THE_Psi_pend).^2.*sin(THE_Psi).*sin(THE_Theta).*(2.0./3.0)-Lz_pend.^2.*THE_Phi_pend_D.*m_pend.*cos(THE_Theta).*cos(THE_Psi_pend).^2.*sin(THE_Psi).*sin(THE_Phi_pend).*(2.0./3.0)-Lz_pend.^2.*THE_Psi_pend_D.*m_pend.*cos(THE_Phi_pend).*cos(THE_Psi_pend).^2.*sin(THE_Theta).*sin(THE_Theta_pend).*(2.0./3.0)+(Lx_pend.^2.*THE_Phi_D.*m_pend.*cos(THE_Psi).^2.*cos(THE_Theta).^2.*cos(THE_Theta_pend).*sin(THE_Theta_pend))./6.0-(Lx_pend.^2.*THE_Theta_D.*m_pend.*cos(THE_Psi).^2.*cos(THE_Theta).*cos(THE_Theta_pend).^2.*sin(THE_Phi_pend))./3.0+(Lx_pend.^2.*THE_Phi_D.*m_pend.*cos(THE_Theta).^2.*cos(THE_Phi_pend).^2.*cos(THE_Theta_pend).*sin(THE_Theta_pend))./6.0+(Ly_pend.^2.*THE_Theta_D.*m_pend.*cos(THE_Psi).^2.*cos(THE_Theta).*cos(THE_Psi_pend).^2.*sin(THE_Phi_pend))./6.0-(Ly_pend.^2.*THE_Phi_D.*m_pend.*cos(THE_Psi).^2.*cos(THE_Theta).^2.*cos(THE_Theta_pend).*sin(THE_Theta_pend))./6.0+(Ly_pend.^2.*THE_Theta_D.*m_pend.*cos(THE_Psi).^2.*cos(THE_Theta).*cos(THE_Theta_pend).^2.*sin(THE_Phi_pend))./3.0-(Ly_pend.^2.*THE_Phi_D.*m_pend.*cos(THE_Theta).^2.*cos(THE_Phi_pend).^2.*cos(THE_Theta_pend).*sin(THE_Theta_pend))./6.0-(Ly_pend.^2.*THE_Phi_D.*m_pend.*cos(THE_Theta).^2.*cos(THE_Psi_pend).^2.*cos(THE_Theta_pend).*sin(THE_Theta_pend))./1.2e+1+(Ly_pend.^2.*THE_Theta_D.*m_pend.*cos(THE_Theta).*cos(THE_Psi_pend).^2.*cos(THE_Theta_pend).^2.*sin(THE_Phi_pend))./6.0-(Ly_pend.^2.*THE_Phi_D.*m_pend.*cos(THE_Phi_pend).^2.*cos(THE_Psi_pend).^2.*cos(THE_Theta_pend).*sin(THE_Theta_pend))./1.2e+1+(Ly_pend.^2.*THE_Phi_pend_D.*m_pend.*cos(THE_Phi_pend).*cos(THE_Psi_pend).^2.*cos(THE_Theta_pend).^2.*sin(THE_Theta))./6.0-Lz_pend.^2.*THE_Theta_D.*m_pend.*cos(THE_Psi).^2.*cos(THE_Theta).*cos(THE_Psi_pend).^2.*sin(THE_Phi_pend).*(2.0./3.0)+(Lz_pend.^2.*THE_Phi_D.*m_pend.*cos(THE_Theta).^2.*cos(THE_Psi_pend).^2.*cos(THE_Theta_pend).*sin(THE_Theta_pend))./3.0-Lz_pend.^2.*THE_Theta_D.*m_pend.*cos(THE_Theta).*cos(THE_Psi_pend).^2.*cos(THE_Theta_pend).^2.*sin(THE_Phi_pend).*(2.0./3.0)+(Lz_pend.^2.*THE_Phi_D.*m_pend.*cos(THE_Phi_pend).^2.*cos(THE_Psi_pend).^2.*cos(THE_Theta_pend).*sin(THE_Theta_pend))./3.0-Lz_pend.^2.*THE_Phi_pend_D.*m_pend.*cos(THE_Phi_pend).*cos(THE_Psi_pend).^2.*cos(THE_Theta_pend).^2.*sin(THE_Theta).*(2.0./3.0)-(Lx_pend.^2.*THE_Phi_D.*m_pend.*cos(THE_Psi).*cos(THE_Theta).*cos(THE_Phi_pend).*sin(THE_Theta))./1.2e+1+(Lx_pend.^2.*THE_Phi_pend_D.*m_pend.*cos(THE_Psi).*cos(THE_Theta).*cos(THE_Theta_pend).*sin(THE_Theta_pend))./6.0+(Ly_pend.^2.*THE_Phi_D.*m_pend.*cos(THE_Psi).*cos(THE_Theta).*cos(THE_Phi_pend).*sin(THE_Theta))./1.2e+1-(Ly_pend.^2.*THE_Phi_pend_D.*m_pend.*cos(THE_Psi).*cos(THE_Theta).*cos(THE_Theta_pend).*sin(THE_Theta_pend))./6.0+(Ly_pend.^2.*THE_Psi_pend_D.*m_pend.*cos(THE_Theta).*sin(THE_Psi).*sin(THE_Phi_pend).*sin(THE_Theta_pend))./6.0+(Ly_pend.^2.*THE_Psi_pend_D.*m_pend.*cos(THE_Psi_pend).*sin(THE_Theta).*sin(THE_Phi_pend).*sin(THE_Psi_pend))./6.0-Lz_pend.^2.*THE_Psi_pend_D.*m_pend.*cos(THE_Psi_pend).*sin(THE_Theta).*sin(THE_Phi_pend).*sin(THE_Psi_pend).*(2.0./3.0)-(Ly_pend.^2.*THE_Psi_D.*m_pend.*cos(THE_Psi).*cos(THE_Theta).*cos(THE_Phi_pend).*cos(THE_Psi_pend).^2.*cos(THE_Theta_pend).^2)./6.0+Lz_pend.^2.*THE_Psi_D.*m_pend.*cos(THE_Psi).*cos(THE_Theta).*cos(THE_Phi_pend).*cos(THE_Psi_pend).^2.*cos(THE_Theta_pend).^2.*(2.0./3.0)-(Lx_pend.^2.*THE_Phi_D.*m_pend.*cos(THE_Psi).*cos(THE_Theta).^2.*cos(THE_Theta_pend).^2.*sin(THE_Psi).*sin(THE_Phi_pend))./6.0+(Ly_pend.^2.*THE_Phi_D.*m_pend.*cos(THE_Psi).*cos(THE_Theta).^2.*cos(THE_Psi_pend).^2.*sin(THE_Psi).*sin(THE_Phi_pend))./1.2e+1+(Ly_pend.^2.*THE_Phi_D.*m_pend.*cos(THE_Psi).*cos(THE_Theta).^2.*cos(THE_Theta_pend).^2.*sin(THE_Psi).*sin(THE_Phi_pend))./6.0-(Ly_pend.^2.*THE_Theta_D.*m_pend.*cos(THE_Phi_pend).*cos(THE_Psi_pend).^2.*cos(THE_Theta_pend).^2.*sin(THE_Psi).*sin(THE_Theta))./6.0-(Ly_pend.^2.*THE_Phi_pend_D.*m_pend.*cos(THE_Theta).*cos(THE_Psi_pend).^2.*cos(THE_Theta_pend).^2.*sin(THE_Psi).*sin(THE_Phi_pend))./6.0+(Ly_pend.^2.*THE_Psi_D.*m_pend.*cos(THE_Phi_pend).^2.*cos(THE_Psi_pend).^2.*cos(THE_Theta_pend).*sin(THE_Theta).*sin(THE_Theta_pend))./6.0-(Lz_pend.^2.*THE_Phi_D.*m_pend.*cos(THE_Psi).*cos(THE_Theta).^2.*cos(THE_Psi_pend).^2.*sin(THE_Psi).*sin(THE_Phi_pend))./3.0+Lz_pend.^2.*THE_Theta_D.*m_pend.*cos(THE_Phi_pend).*cos(THE_Psi_pend).^2.*cos(THE_Theta_pend).^2.*sin(THE_Psi).*sin(THE_Theta).*(2.0./3.0)+Lz_pend.^2.*THE_Phi_pend_D.*m_pend.*cos(THE_Theta).*cos(THE_Psi_pend).^2.*cos(THE_Theta_pend).^2.*sin(THE_Psi).*sin(THE_Phi_pend).*(2.0./3.0)-Lz_pend.^2.*THE_Psi_D.*m_pend.*cos(THE_Phi_pend).^2.*cos(THE_Psi_pend).^2.*cos(THE_Theta_pend).*sin(THE_Theta).*sin(THE_Theta_pend).*(2.0./3.0)-(Lz_pend.*THE_Phi_D.*Tv_Z_pend.*m_pend.*cos(THE_Psi).^2.*cos(THE_Theta).^2.*cos(THE_Psi_pend).*sin(THE_Theta_pend))./2.0-(Lx_pend.^2.*THE_Theta_D.*m_pend.*cos(THE_Psi).*cos(THE_Theta).*cos(THE_Theta_pend).*sin(THE_Psi).*sin(THE_Theta_pend))./3.0+(Ly_pend.^2.*THE_Theta_D.*m_pend.*cos(THE_Psi).*cos(THE_Theta).*cos(THE_Theta_pend).*sin(THE_Psi).*sin(THE_Theta_pend))./3.0+(Ly_pend.^2.*THE_Theta_D.*m_pend.*cos(THE_Psi).*cos(THE_Psi_pend).*cos(THE_Theta_pend).*sin(THE_Theta).*sin(THE_Psi_pend))./6.0+(Ly_pend.^2.*THE_Psi_pend_D.*m_pend.*cos(THE_Theta).*cos(THE_Phi_pend).*cos(THE_Psi_pend).*sin(THE_Psi).*sin(THE_Psi_pend))./6.0+(Ly_pend.^2.*THE_Theta_D.*m_pend.*cos(THE_Theta).*cos(THE_Phi_pend).*cos(THE_Psi_pend).*sin(THE_Psi_pend).*sin(THE_Theta_pend))./6.0-(Ly_pend.^2.*THE_Phi_D.*m_pend.*cos(THE_Phi_pend).*cos(THE_Psi_pend).*cos(THE_Theta_pend).*sin(THE_Phi_pend).*sin(THE_Psi_pend))./1.2e+1-Lz_pend.^2.*THE_Theta_D.*m_pend.*cos(THE_Psi).*cos(THE_Psi_pend).*cos(THE_Theta_pend).*sin(THE_Theta).*sin(THE_Psi_pend).*(2.0./3.0)-Lz_pend.^2.*THE_Psi_pend_D.*m_pend.*cos(THE_Theta).*cos(THE_Phi_pend).*cos(THE_Psi_pend).*sin(THE_Psi).*sin(THE_Psi_pend).*(2.0./3.0)-Lz_pend.^2.*THE_Theta_D.*m_pend.*cos(THE_Theta).*cos(THE_Phi_pend).*cos(THE_Psi_pend).*sin(THE_Psi_pend).*sin(THE_Theta_pend).*(2.0./3.0)+(Lz_pend.^2.*THE_Phi_D.*m_pend.*cos(THE_Phi_pend).*cos(THE_Psi_pend).*cos(THE_Theta_pend).*sin(THE_Phi_pend).*sin(THE_Psi_pend))./3.0-(Lx_pend.^2.*THE_Phi_D.*m_pend.*cos(THE_Psi).^2.*cos(THE_Theta).^2.*cos(THE_Phi_pend).^2.*cos(THE_Theta_pend).*sin(THE_Theta_pend))./1.2e+1+(Ly_pend.^2.*THE_Phi_D.*m_pend.*cos(THE_Psi).^2.*cos(THE_Theta).^2.*cos(THE_Phi_pend).^2.*cos(THE_Theta_pend).*sin(THE_Theta_pend))./1.2e+1+(Ly_pend.^2.*THE_Phi_D.*m_pend.*cos(THE_Psi).^2.*cos(THE_Theta).^2.*cos(THE_Psi_pend).^2.*cos(THE_Theta_pend).*sin(THE_Theta_pend))./6.0-(Ly_pend.^2.*THE_Theta_D.*m_pend.*cos(THE_Psi).^2.*cos(THE_Theta).*cos(THE_Psi_pend).^2.*cos(THE_Theta_pend).^2.*sin(THE_Phi_pend))./3.0+(Ly_pend.^2.*THE_Phi_D.*m_pend.*cos(THE_Theta).^2.*cos(THE_Phi_pend).^2.*cos(THE_Psi_pend).^2.*cos(THE_Theta_pend).*sin(THE_Theta_pend))./6.0-Lz_pend.^2.*THE_Phi_D.*m_pend.*cos(THE_Psi).^2.*cos(THE_Theta).^2.*cos(THE_Psi_pend).^2.*cos(THE_Theta_pend).*sin(THE_Theta_pend).*(2.0./3.0)+Lz_pend.^2.*THE_Theta_D.*m_pend.*cos(THE_Psi).^2.*cos(THE_Theta).*cos(THE_Psi_pend).^2.*cos(THE_Theta_pend).^2.*sin(THE_Phi_pend).*(4.0./3.0)-Lz_pend.^2.*THE_Phi_D.*m_pend.*cos(THE_Theta).^2.*cos(THE_Phi_pend).^2.*cos(THE_Psi_pend).^2.*cos(THE_Theta_pend).*sin(THE_Theta_pend).*(2.0./3.0)-(Ly_pend.^2.*THE_Phi_pend_D.*m_pend.*cos(THE_Psi_pend).*sin(THE_Theta).*sin(THE_Phi_pend).*sin(THE_Psi_pend).*sin(THE_Theta_pend))./6.0+Lz_pend.^2.*THE_Phi_pend_D.*m_pend.*cos(THE_Psi_pend).*sin(THE_Theta).*sin(THE_Phi_pend).*sin(THE_Psi_pend).*sin(THE_Theta_pend).*(2.0./3.0)+(Lx_pend.^2.*THE_Phi_D.*m_pend.*cos(THE_Psi).*cos(THE_Theta).*cos(THE_Phi_pend).*cos(THE_Theta_pend).^2.*sin(THE_Theta))./6.0-(Ly_pend.^2.*THE_Phi_D.*m_pend.*cos(THE_Psi).*cos(THE_Theta).*cos(THE_Phi_pend).*cos(THE_Psi_pend).^2.*sin(THE_Theta))./1.2e+1-(Ly_pend.^2.*THE_Phi_D.*m_pend.*cos(THE_Psi).*cos(THE_Theta).*cos(THE_Phi_pend).*cos(THE_Theta_pend).^2.*sin(THE_Theta))./6.0+(Ly_pend.^2.*THE_Phi_pend_D.*m_pend.*cos(THE_Psi).*cos(THE_Theta).*cos(THE_Psi_pend).^2.*cos(THE_Theta_pend).*sin(THE_Theta_pend))./6.0+(Lz_pend.^2.*THE_Phi_D.*m_pend.*cos(THE_Psi).*cos(THE_Theta).*cos(THE_Phi_pend).*cos(THE_Psi_pend).^2.*sin(THE_Theta))./3.0-Lz_pend.^2.*THE_Phi_pend_D.*m_pend.*cos(THE_Psi).*cos(THE_Theta).*cos(THE_Psi_pend).^2.*cos(THE_Theta_pend).*sin(THE_Theta_pend).*(2.0./3.0)-(Ly_pend.^2.*THE_Psi_pend_D.*m_pend.*cos(THE_Theta).*cos(THE_Psi_pend).^2.*sin(THE_Psi).*sin(THE_Phi_pend).*sin(THE_Theta_pend))./6.0+Lz_pend.^2.*THE_Psi_pend_D.*m_pend.*cos(THE_Theta).*cos(THE_Psi_pend).^2.*sin(THE_Psi).*sin(THE_Phi_pend).*sin(THE_Theta_pend).*(2.0./3.0)-(Lx_pend.^2.*THE_Psi_D.*m_pend.*cos(THE_Theta).*cos(THE_Phi_pend).*cos(THE_Theta_pend).*sin(THE_Psi).*sin(THE_Phi_pend).*sin(THE_Theta_pend))./6.0+(Lx_pend.^2.*THE_Theta_D.*m_pend.*cos(THE_Psi).*cos(THE_Phi_pend).*cos(THE_Theta_pend).*sin(THE_Theta).*sin(THE_Phi_pend).*sin(THE_Theta_pend))./6.0+(Ly_pend.^2.*THE_Phi_D.*m_pend.*cos(THE_Theta).*cos(THE_Psi_pend).*cos(THE_Theta_pend).*sin(THE_Psi).*sin(THE_Theta).*sin(THE_Psi_pend))./1.2e+1+(Ly_pend.^2.*THE_Psi_D.*m_pend.*cos(THE_Theta).*cos(THE_Phi_pend).*cos(THE_Theta_pend).*sin(THE_Psi).*sin(THE_Phi_pend).*sin(THE_Theta_pend))./6.0-(Ly_pend.^2.*THE_Theta_D.*m_pend.*cos(THE_Psi).*cos(THE_Phi_pend).*cos(THE_Theta_pend).*sin(THE_Theta).*sin(THE_Phi_pend).*sin(THE_Theta_pend))./6.0+(Ly_pend.^2.*THE_Psi_D.*m_pend.*cos(THE_Phi_pend).*cos(THE_Psi_pend).*cos(THE_Theta_pend).*sin(THE_Theta).*sin(THE_Phi_pend).*sin(THE_Psi_pend))./6.0-(Ly_pend.^2.*THE_Phi_pend_D.*m_pend.*cos(THE_Theta).*cos(THE_Phi_pend).*cos(THE_Psi_pend).*sin(THE_Psi).*sin(THE_Psi_pend).*sin(THE_Theta_pend))./6.0-(Lz_pend.^2.*THE_Phi_D.*m_pend.*cos(THE_Theta).*cos(THE_Psi_pend).*cos(THE_Theta_pend).*sin(THE_Psi).*sin(THE_Theta).*sin(THE_Psi_pend))./3.0-Lz_pend.^2.*THE_Psi_D.*m_pend.*cos(THE_Phi_pend).*cos(THE_Psi_pend).*cos(THE_Theta_pend).*sin(THE_Theta).*sin(THE_Phi_pend).*sin(THE_Psi_pend).*(2.0./3.0)+Lz_pend.^2.*THE_Phi_pend_D.*m_pend.*cos(THE_Theta).*cos(THE_Phi_pend).*cos(THE_Psi_pend).*sin(THE_Psi).*sin(THE_Psi_pend).*sin(THE_Theta_pend).*(2.0./3.0)+Lz_pend.*THE_Psi_D.*Tv_Z_pend.*m_pend.*cos(THE_Psi).*cos(THE_Theta).*cos(THE_Phi_pend).*cos(THE_Psi_pend).*cos(THE_Theta_pend)-(Ly_pend.^2.*THE_Phi_D.*m_pend.*cos(THE_Psi).*cos(THE_Theta).^2.*cos(THE_Psi_pend).^2.*cos(THE_Theta_pend).^2.*sin(THE_Psi).*sin(THE_Phi_pend))./6.0+Lz_pend.^2.*THE_Phi_D.*m_pend.*cos(THE_Psi).*cos(THE_Theta).^2.*cos(THE_Psi_pend).^2.*cos(THE_Theta_pend).^2.*sin(THE_Psi).*sin(THE_Phi_pend).*(2.0./3.0)+(Ly_pend.^2.*THE_Theta_D.*m_pend.*cos(THE_Psi_pend).*sin(THE_Psi).*sin(THE_Theta).*sin(THE_Phi_pend).*sin(THE_Psi_pend).*sin(THE_Theta_pend))./6.0-Lz_pend.^2.*THE_Theta_D.*m_pend.*cos(THE_Psi_pend).*sin(THE_Psi).*sin(THE_Theta).*sin(THE_Phi_pend).*sin(THE_Psi_pend).*sin(THE_Theta_pend).*(2.0./3.0)+Lz_pend.*THE_Theta_D.*Tv_Z_pend.*m_pend.*cos(THE_Psi).*cos(THE_Theta).*cos(THE_Psi_pend).*sin(THE_Psi).*sin(THE_Theta_pend)+(Lx_pend.^2.*THE_Theta_D.*m_pend.*cos(THE_Psi).*cos(THE_Theta).*cos(THE_Phi_pend).^2.*cos(THE_Theta_pend).*sin(THE_Psi).*sin(THE_Theta_pend))./6.0-(Ly_pend.^2.*THE_Theta_D.*m_pend.*cos(THE_Psi).*cos(THE_Theta).*cos(THE_Phi_pend).^2.*cos(THE_Theta_pend).*sin(THE_Psi).*sin(THE_Theta_pend))./6.0-(Ly_pend.^2.*THE_Theta_D.*m_pend.*cos(THE_Psi).*cos(THE_Theta).*cos(THE_Psi_pend).^2.*cos(THE_Theta_pend).*sin(THE_Psi).*sin(THE_Theta_pend))./3.0+(Ly_pend.^2.*THE_Psi_D.*m_pend.*cos(THE_Theta).*cos(THE_Phi_pend).^2.*cos(THE_Psi_pend).*cos(THE_Theta_pend).*sin(THE_Psi).*sin(THE_Psi_pend))./6.0-(Ly_pend.^2.*THE_Theta_D.*m_pend.*cos(THE_Psi).*cos(THE_Phi_pend).^2.*cos(THE_Psi_pend).*cos(THE_Theta_pend).*sin(THE_Theta).*sin(THE_Psi_pend))./6.0-(Ly_pend.^2.*THE_Theta_D.*m_pend.*cos(THE_Psi).^2.*cos(THE_Theta).*cos(THE_Phi_pend).*cos(THE_Psi_pend).*sin(THE_Psi_pend).*sin(THE_Theta_pend))./6.0+(Ly_pend.^2.*THE_Phi_D.*m_pend.*cos(THE_Theta).^2.*cos(THE_Phi_pend).*cos(THE_Psi_pend).*cos(THE_Theta_pend).*sin(THE_Phi_pend).*sin(THE_Psi_pend))./6.0+Lz_pend.^2.*THE_Theta_D.*m_pend.*cos(THE_Psi).*cos(THE_Theta).*cos(THE_Psi_pend).^2.*cos(THE_Theta_pend).*sin(THE_Psi).*sin(THE_Theta_pend).*(4.0./3.0)-Lz_pend.^2.*THE_Psi_D.*m_pend.*cos(THE_Theta).*cos(THE_Phi_pend).^2.*cos(THE_Psi_pend).*cos(THE_Theta_pend).*sin(THE_Psi).*sin(THE_Psi_pend).*(2.0./3.0)+Lz_pend.^2.*THE_Theta_D.*m_pend.*cos(THE_Psi).*cos(THE_Phi_pend).^2.*cos(THE_Psi_pend).*cos(THE_Theta_pend).*sin(THE_Theta).*sin(THE_Psi_pend).*(2.0./3.0)+Lz_pend.^2.*THE_Theta_D.*m_pend.*cos(THE_Psi).^2.*cos(THE_Theta).*cos(THE_Phi_pend).*cos(THE_Psi_pend).*sin(THE_Psi_pend).*sin(THE_Theta_pend).*(2.0./3.0)-Lz_pend.^2.*THE_Phi_D.*m_pend.*cos(THE_Theta).^2.*cos(THE_Phi_pend).*cos(THE_Psi_pend).*cos(THE_Theta_pend).*sin(THE_Phi_pend).*sin(THE_Psi_pend).*(2.0./3.0)-(Ly_pend.^2.*THE_Phi_D.*m_pend.*cos(THE_Psi).^2.*cos(THE_Theta).^2.*cos(THE_Phi_pend).^2.*cos(THE_Psi_pend).^2.*cos(THE_Theta_pend).*sin(THE_Theta_pend))./1.2e+1+(Lz_pend.^2.*THE_Phi_D.*m_pend.*cos(THE_Psi).^2.*cos(THE_Theta).^2.*cos(THE_Phi_pend).^2.*cos(THE_Psi_pend).^2.*cos(THE_Theta_pend).*sin(THE_Theta_pend))./3.0+Lz_pend.*THE_Theta_D.*Tv_Z_pend.*m_pend.*cos(THE_Psi).^2.*cos(THE_Theta).*cos(THE_Psi_pend).*cos(THE_Theta_pend).*sin(THE_Phi_pend)+(Ly_pend.^2.*THE_Phi_D.*m_pend.*cos(THE_Psi).*cos(THE_Theta).*cos(THE_Phi_pend).*cos(THE_Psi_pend).^2.*cos(THE_Theta_pend).^2.*sin(THE_Theta))./6.0-Lz_pend.^2.*THE_Phi_D.*m_pend.*cos(THE_Psi).*cos(THE_Theta).*cos(THE_Phi_pend).*cos(THE_Psi_pend).^2.*cos(THE_Theta_pend).^2.*sin(THE_Theta).*(2.0./3.0)+(Lx_pend.^2.*THE_Phi_D.*m_pend.*cos(THE_Theta).*cos(THE_Phi_pend).*cos(THE_Theta_pend).*sin(THE_Psi).*sin(THE_Theta).*sin(THE_Phi_pend).*sin(THE_Theta_pend))./6.0-(Ly_pend.^2.*THE_Phi_D.*m_pend.*cos(THE_Psi).*cos(THE_Theta).*cos(THE_Psi_pend).*sin(THE_Theta).*sin(THE_Phi_pend).*sin(THE_Psi_pend).*sin(THE_Theta_pend))./1.2e+1-(Ly_pend.^2.*THE_Phi_D.*m_pend.*cos(THE_Theta).*cos(THE_Phi_pend).*cos(THE_Theta_pend).*sin(THE_Psi).*sin(THE_Theta).*sin(THE_Phi_pend).*sin(THE_Theta_pend))./6.0+(Lz_pend.^2.*THE_Phi_D.*m_pend.*cos(THE_Psi).*cos(THE_Theta).*cos(THE_Psi_pend).*sin(THE_Theta).*sin(THE_Phi_pend).*sin(THE_Psi_pend).*sin(THE_Theta_pend))./3.0-(Lz_pend.*THE_Phi_D.*Tv_Z_pend.*m_pend.*cos(THE_Psi).*cos(THE_Theta).*cos(THE_Phi_pend).*cos(THE_Psi_pend).*cos(THE_Theta_pend).*sin(THE_Theta))./2.0-(Ly_pend.^2.*THE_Phi_D.*m_pend.*cos(THE_Psi).*cos(THE_Theta).^2.*cos(THE_Phi_pend).*cos(THE_Psi_pend).*sin(THE_Psi).*sin(THE_Psi_pend).*sin(THE_Theta_pend))./1.2e+1-(Ly_pend.^2.*THE_Phi_D.*m_pend.*cos(THE_Theta).*cos(THE_Phi_pend).^2.*cos(THE_Psi_pend).*cos(THE_Theta_pend).*sin(THE_Psi).*sin(THE_Theta).*sin(THE_Psi_pend))./6.0-(Ly_pend.^2.*THE_Psi_D.*m_pend.*cos(THE_Theta).*cos(THE_Phi_pend).*cos(THE_Psi_pend).^2.*cos(THE_Theta_pend).*sin(THE_Psi).*sin(THE_Phi_pend).*sin(THE_Theta_pend))./6.0+(Ly_pend.^2.*THE_Theta_D.*m_pend.*cos(THE_Psi).*cos(THE_Phi_pend).*cos(THE_Psi_pend).^2.*cos(THE_Theta_pend).*sin(THE_Theta).*sin(THE_Phi_pend).*sin(THE_Theta_pend))./6.0+(Lz_pend.^2.*THE_Phi_D.*m_pend.*cos(THE_Psi).*cos(THE_Theta).^2.*cos(THE_Phi_pend).*cos(THE_Psi_pend).*sin(THE_Psi).*sin(THE_Psi_pend).*sin(THE_Theta_pend))./3.0+Lz_pend.^2.*THE_Phi_D.*m_pend.*cos(THE_Theta).*cos(THE_Phi_pend).^2.*cos(THE_Psi_pend).*cos(THE_Theta_pend).*sin(THE_Psi).*sin(THE_Theta).*sin(THE_Psi_pend).*(2.0./3.0)+Lz_pend.^2.*THE_Psi_D.*m_pend.*cos(THE_Theta).*cos(THE_Phi_pend).*cos(THE_Psi_pend).^2.*cos(THE_Theta_pend).*sin(THE_Psi).*sin(THE_Phi_pend).*sin(THE_Theta_pend).*(2.0./3.0)-Lz_pend.^2.*THE_Theta_D.*m_pend.*cos(THE_Psi).*cos(THE_Phi_pend).*cos(THE_Psi_pend).^2.*cos(THE_Theta_pend).*sin(THE_Theta).*sin(THE_Phi_pend).*sin(THE_Theta_pend).*(2.0./3.0)+(Lz_pend.*THE_Phi_D.*Tv_Z_pend.*m_pend.*cos(THE_Psi).*cos(THE_Theta).^2.*cos(THE_Psi_pend).*cos(THE_Theta_pend).*sin(THE_Psi).*sin(THE_Phi_pend))./2.0+(Ly_pend.^2.*THE_Theta_D.*m_pend.*cos(THE_Psi).*cos(THE_Theta).*cos(THE_Phi_pend).^2.*cos(THE_Psi_pend).^2.*cos(THE_Theta_pend).*sin(THE_Psi).*sin(THE_Theta_pend))./6.0-(Ly_pend.^2.*THE_Phi_D.*m_pend.*cos(THE_Psi).^2.*cos(THE_Theta).^2.*cos(THE_Phi_pend).*cos(THE_Psi_pend).*cos(THE_Theta_pend).*sin(THE_Phi_pend).*sin(THE_Psi_pend))./1.2e+1-Lz_pend.^2.*THE_Theta_D.*m_pend.*cos(THE_Psi).*cos(THE_Theta).*cos(THE_Phi_pend).^2.*cos(THE_Psi_pend).^2.*cos(THE_Theta_pend).*sin(THE_Psi).*sin(THE_Theta_pend).*(2.0./3.0)+(Lz_pend.^2.*THE_Phi_D.*m_pend.*cos(THE_Psi).^2.*cos(THE_Theta).^2.*cos(THE_Phi_pend).*cos(THE_Psi_pend).*cos(THE_Theta_pend).*sin(THE_Phi_pend).*sin(THE_Psi_pend))./3.0+(Ly_pend.^2.*THE_Phi_D.*m_pend.*cos(THE_Theta).*cos(THE_Phi_pend).*cos(THE_Psi_pend).^2.*cos(THE_Theta_pend).*sin(THE_Psi).*sin(THE_Theta).*sin(THE_Phi_pend).*sin(THE_Theta_pend))./6.0-Lz_pend.^2.*THE_Phi_D.*m_pend.*cos(THE_Theta).*cos(THE_Phi_pend).*cos(THE_Psi_pend).^2.*cos(THE_Theta_pend).*sin(THE_Psi).*sin(THE_Theta).*sin(THE_Phi_pend).*sin(THE_Theta_pend).*(2.0./3.0)+(Ly_pend.^2.*THE_Theta_D.*m_pend.*cos(THE_Psi).*cos(THE_Theta).*cos(THE_Phi_pend).*cos(THE_Psi_pend).*cos(THE_Theta_pend).*sin(THE_Psi).*sin(THE_Phi_pend).*sin(THE_Psi_pend))./6.0-Lz_pend.^2.*THE_Theta_D.*m_pend.*cos(THE_Psi).*cos(THE_Theta).*cos(THE_Phi_pend).*cos(THE_Psi_pend).*cos(THE_Theta_pend).*sin(THE_Psi).*sin(THE_Phi_pend).*sin(THE_Psi_pend).*(2.0./3.0),Ly_pend.^2.*THE_Phi_D.*m_pend.*sin(THE_Psi_pend.*2.0).*(-1.0./2.4e+1)+(Lz_pend.^2.*THE_Phi_D.*m_pend.*sin(THE_Psi_pend.*2.0))./6.0+(Ly_pend.^2.*THE_Psi_D.*m_pend.*cos(THE_Theta).*sin(THE_Psi).*sin(THE_Theta_pend))./6.0+(Ly_pend.^2.*THE_Psi_D.*m_pend.*cos(THE_Psi_pend).*sin(THE_Theta).*sin(THE_Psi_pend))./6.0+(Ly_pend.^2.*THE_Phi_D.*m_pend.*cos(THE_Phi_pend).*sin(THE_Phi_pend).*sin(THE_Theta_pend))./1.2e+1+(Ly_pend.^2.*THE_Theta_pend_D.*m_pend.*cos(THE_Phi_pend).*sin(THE_Theta).*sin(THE_Theta_pend))./6.0+Lz_pend.^2.*THE_Theta_D.*m_pend.*cos(THE_Psi).*sin(THE_Theta).*sin(THE_Theta_pend).*(2.0./3.0)-Lz_pend.^2.*THE_Psi_D.*m_pend.*cos(THE_Psi_pend).*sin(THE_Theta).*sin(THE_Psi_pend).*(2.0./3.0)-(Lz_pend.^2.*THE_Phi_D.*m_pend.*cos(THE_Phi_pend).*sin(THE_Phi_pend).*sin(THE_Theta_pend))./3.0+Lz_pend.^2.*THE_Phi_pend_D.*m_pend.*cos(THE_Theta_pend).*sin(THE_Theta).*sin(THE_Phi_pend).*(2.0./3.0)+(Lz_pend.*THE_Phi_D.*Tv_Z_pend.*m_pend.*cos(THE_Theta_pend).*sin(THE_Psi_pend))./2.0+(Ly_pend.^2.*THE_Phi_D.*m_pend.*cos(THE_Theta).^2.*cos(THE_Psi_pend).*sin(THE_Psi_pend))./6.0+(Ly_pend.^2.*THE_Phi_D.*m_pend.*cos(THE_Phi_pend).^2.*cos(THE_Psi_pend).*sin(THE_Psi_pend))./6.0-Lz_pend.^2.*THE_Phi_D.*m_pend.*cos(THE_Theta).^2.*cos(THE_Psi_pend).*sin(THE_Psi_pend).*(2.0./3.0)-Lz_pend.^2.*THE_Phi_D.*m_pend.*cos(THE_Phi_pend).^2.*cos(THE_Psi_pend).*sin(THE_Psi_pend).*(2.0./3.0)-(Ly_pend.^2.*THE_Theta_pend_D.*m_pend.*cos(THE_Psi).*cos(THE_Theta).*cos(THE_Theta_pend))./6.0-Lz_pend.^2.*THE_Theta_D.*m_pend.*cos(THE_Theta).*cos(THE_Phi_pend).*cos(THE_Theta_pend).*(2.0./3.0)-Lz_pend.*THE_Psi_D.*Tv_Z_pend.*m_pend.*cos(THE_Theta_pend).*sin(THE_Theta).*sin(THE_Psi_pend)-(Ly_pend.^2.*THE_Theta_D.*m_pend.*cos(THE_Psi).^2.*cos(THE_Theta).*cos(THE_Phi_pend).*cos(THE_Theta_pend))./6.0-(Ly_pend.^2.*THE_Theta_D.*m_pend.*cos(THE_Theta).*cos(THE_Phi_pend).*cos(THE_Psi_pend).^2.*cos(THE_Theta_pend))./6.0+(Ly_pend.^2.*THE_Theta_pend_D.*m_pend.*cos(THE_Psi).*cos(THE_Theta).*cos(THE_Psi_pend).^2.*cos(THE_Theta_pend))./6.0+Lz_pend.^2.*THE_Theta_D.*m_pend.*cos(THE_Psi).^2.*cos(THE_Theta).*cos(THE_Phi_pend).*cos(THE_Theta_pend).*(2.0./3.0)+Lz_pend.^2.*THE_Theta_D.*m_pend.*cos(THE_Theta).*cos(THE_Phi_pend).*cos(THE_Psi_pend).^2.*cos(THE_Theta_pend).*(2.0./3.0)-Lz_pend.^2.*THE_Theta_pend_D.*m_pend.*cos(THE_Psi).*cos(THE_Theta).*cos(THE_Psi_pend).^2.*cos(THE_Theta_pend).*(2.0./3.0)-(Ly_pend.^2.*THE_Psi_D.*m_pend.*cos(THE_Theta).*cos(THE_Phi_pend).^2.*sin(THE_Psi).*sin(THE_Theta_pend))./6.0-(Ly_pend.^2.*THE_Psi_D.*m_pend.*cos(THE_Theta).*cos(THE_Psi_pend).^2.*sin(THE_Psi).*sin(THE_Theta_pend))./6.0+(Ly_pend.^2.*THE_Theta_D.*m_pend.*cos(THE_Psi).*cos(THE_Phi_pend).^2.*sin(THE_Theta).*sin(THE_Theta_pend))./6.0+(Ly_pend.^2.*THE_Theta_D.*m_pend.*cos(THE_Psi).*cos(THE_Psi_pend).^2.*sin(THE_Theta).*sin(THE_Theta_pend))./6.0-(Ly_pend.^2.*THE_Psi_D.*m_pend.*cos(THE_Phi_pend).^2.*cos(THE_Psi_pend).*sin(THE_Theta).*sin(THE_Psi_pend))./3.0-(Ly_pend.^2.*THE_Phi_D.*m_pend.*cos(THE_Theta).^2.*cos(THE_Phi_pend).*sin(THE_Phi_pend).*sin(THE_Theta_pend))./6.0-(Ly_pend.^2.*THE_Phi_D.*m_pend.*cos(THE_Phi_pend).*cos(THE_Psi_pend).^2.*sin(THE_Phi_pend).*sin(THE_Theta_pend))./6.0+(Ly_pend.^2.*THE_Phi_pend_D.*m_pend.*cos(THE_Psi_pend).^2.*cos(THE_Theta_pend).*sin(THE_Theta).*sin(THE_Phi_pend))./6.0-(Ly_pend.^2.*THE_Theta_pend_D.*m_pend.*cos(THE_Phi_pend).*cos(THE_Psi_pend).^2.*sin(THE_Theta).*sin(THE_Theta_pend))./6.0+Lz_pend.^2.*THE_Psi_D.*m_pend.*cos(THE_Theta).*cos(THE_Phi_pend).^2.*sin(THE_Psi).*sin(THE_Theta_pend).*(2.0./3.0)+Lz_pend.^2.*THE_Psi_D.*m_pend.*cos(THE_Theta).*cos(THE_Psi_pend).^2.*sin(THE_Psi).*sin(THE_Theta_pend).*(2.0./3.0)-Lz_pend.^2.*THE_Theta_D.*m_pend.*cos(THE_Psi).*cos(THE_Phi_pend).^2.*sin(THE_Theta).*sin(THE_Theta_pend).*(2.0./3.0)-Lz_pend.^2.*THE_Theta_D.*m_pend.*cos(THE_Psi).*cos(THE_Psi_pend).^2.*sin(THE_Theta).*sin(THE_Theta_pend).*(2.0./3.0)+Lz_pend.^2.*THE_Psi_D.*m_pend.*cos(THE_Phi_pend).^2.*cos(THE_Psi_pend).*sin(THE_Theta).*sin(THE_Psi_pend).*(4.0./3.0)+Lz_pend.^2.*THE_Phi_D.*m_pend.*cos(THE_Theta).^2.*cos(THE_Phi_pend).*sin(THE_Phi_pend).*sin(THE_Theta_pend).*(2.0./3.0)+Lz_pend.^2.*THE_Phi_D.*m_pend.*cos(THE_Phi_pend).*cos(THE_Psi_pend).^2.*sin(THE_Phi_pend).*sin(THE_Theta_pend).*(2.0./3.0)-Lz_pend.^2.*THE_Phi_pend_D.*m_pend.*cos(THE_Psi_pend).^2.*cos(THE_Theta_pend).*sin(THE_Theta).*sin(THE_Phi_pend).*(2.0./3.0)+Lz_pend.^2.*THE_Theta_pend_D.*m_pend.*cos(THE_Phi_pend).*cos(THE_Psi_pend).^2.*sin(THE_Theta).*sin(THE_Theta_pend).*(2.0./3.0)-(Ly_pend.^2.*THE_Phi_D.*m_pend.*cos(THE_Psi).^2.*cos(THE_Theta).^2.*cos(THE_Psi_pend).*sin(THE_Psi_pend))./1.2e+1-(Ly_pend.^2.*THE_Phi_D.*m_pend.*cos(THE_Theta).^2.*cos(THE_Phi_pend).^2.*cos(THE_Psi_pend).*sin(THE_Psi_pend))./3.0-(Ly_pend.^2.*THE_Phi_D.*m_pend.*cos(THE_Theta).^2.*cos(THE_Psi_pend).*cos(THE_Theta_pend).^2.*sin(THE_Psi_pend))./1.2e+1-(Ly_pend.^2.*THE_Phi_D.*m_pend.*cos(THE_Phi_pend).^2.*cos(THE_Psi_pend).*cos(THE_Theta_pend).^2.*sin(THE_Psi_pend))./1.2e+1+(Lz_pend.^2.*THE_Phi_D.*m_pend.*cos(THE_Psi).^2.*cos(THE_Theta).^2.*cos(THE_Psi_pend).*sin(THE_Psi_pend))./3.0+Lz_pend.^2.*THE_Phi_D.*m_pend.*cos(THE_Theta).^2.*cos(THE_Phi_pend).^2.*cos(THE_Psi_pend).*sin(THE_Psi_pend).*(4.0./3.0)+(Lz_pend.^2.*THE_Phi_D.*m_pend.*cos(THE_Theta).^2.*cos(THE_Psi_pend).*cos(THE_Theta_pend).^2.*sin(THE_Psi_pend))./3.0+(Lz_pend.^2.*THE_Phi_D.*m_pend.*cos(THE_Phi_pend).^2.*cos(THE_Psi_pend).*cos(THE_Theta_pend).^2.*sin(THE_Psi_pend))./3.0+(Ly_pend.^2.*THE_Psi_D.*m_pend.*cos(THE_Psi).*cos(THE_Theta).*cos(THE_Theta_pend).*sin(THE_Phi_pend))./6.0+Lz_pend.^2.*THE_Phi_pend_D.*m_pend.*cos(THE_Theta).*cos(THE_Phi_pend).*cos(THE_Theta_pend).*sin(THE_Psi).*(2.0./3.0)-(Ly_pend.^2.*THE_Phi_D.*m_pend.*cos(THE_Theta).*sin(THE_Psi).*sin(THE_Theta).*sin(THE_Theta_pend))./1.2e+1-(Ly_pend.^2.*THE_Psi_D.*m_pend.*cos(THE_Phi_pend).*sin(THE_Theta).*sin(THE_Phi_pend).*sin(THE_Theta_pend))./6.0-(Ly_pend.^2.*THE_Theta_pend_D.*m_pend.*cos(THE_Theta).*sin(THE_Psi).*sin(THE_Phi_pend).*sin(THE_Theta_pend))./6.0-(Ly_pend.^2.*THE_Theta_pend_D.*m_pend.*cos(THE_Psi_pend).*sin(THE_Theta).*sin(THE_Phi_pend).*sin(THE_Psi_pend))./6.0+(Lz_pend.^2.*THE_Phi_D.*m_pend.*cos(THE_Theta).*sin(THE_Psi).*sin(THE_Theta).*sin(THE_Theta_pend))./3.0-Lz_pend.^2.*THE_Theta_D.*m_pend.*cos(THE_Theta_pend).*sin(THE_Psi).*sin(THE_Theta).*sin(THE_Phi_pend).*(2.0./3.0)+Lz_pend.^2.*THE_Psi_D.*m_pend.*cos(THE_Phi_pend).*sin(THE_Theta).*sin(THE_Phi_pend).*sin(THE_Theta_pend).*(2.0./3.0)+Lz_pend.^2.*THE_Theta_pend_D.*m_pend.*cos(THE_Psi_pend).*sin(THE_Theta).*sin(THE_Phi_pend).*sin(THE_Psi_pend).*(2.0./3.0)-Lz_pend.*THE_Theta_D.*Tv_Z_pend.*m_pend.*cos(THE_Psi).^2.*cos(THE_Theta).*cos(THE_Phi_pend).*cos(THE_Psi_pend)+(Ly_pend.^2.*THE_Theta_D.*m_pend.*cos(THE_Psi).^2.*cos(THE_Theta).*cos(THE_Phi_pend).*cos(THE_Psi_pend).^2.*cos(THE_Theta_pend))./3.0-Lz_pend.^2.*THE_Theta_D.*m_pend.*cos(THE_Psi).^2.*cos(THE_Theta).*cos(THE_Phi_pend).*cos(THE_Psi_pend).^2.*cos(THE_Theta_pend).*(4.0./3.0)+(Ly_pend.^2.*THE_Phi_D.*m_pend.*cos(THE_Psi).^2.*cos(THE_Theta).^2.*cos(THE_Phi_pend).*sin(THE_Phi_pend).*sin(THE_Theta_pend))./1.2e+1+(Ly_pend.^2.*THE_Psi_D.*m_pend.*cos(THE_Theta).*cos(THE_Phi_pend).^2.*cos(THE_Psi_pend).^2.*sin(THE_Psi).*sin(THE_Theta_pend))./3.0-(Ly_pend.^2.*THE_Theta_D.*m_pend.*cos(THE_Psi).*cos(THE_Phi_pend).^2.*cos(THE_Psi_pend).^2.*sin(THE_Theta).*sin(THE_Theta_pend))./3.0+(Ly_pend.^2.*THE_Phi_D.*m_pend.*cos(THE_Theta).^2.*cos(THE_Phi_pend).*cos(THE_Psi_pend).^2.*sin(THE_Phi_pend).*sin(THE_Theta_pend))./3.0+(Ly_pend.^2.*THE_Psi_D.*m_pend.*cos(THE_Phi_pend).^2.*cos(THE_Psi_pend).*cos(THE_Theta_pend).^2.*sin(THE_Theta).*sin(THE_Psi_pend))./6.0-(Lz_pend.^2.*THE_Phi_D.*m_pend.*cos(THE_Psi).^2.*cos(THE_Theta).^2.*cos(THE_Phi_pend).*sin(THE_Phi_pend).*sin(THE_Theta_pend))./3.0-Lz_pend.^2.*THE_Psi_D.*m_pend.*cos(THE_Theta).*cos(THE_Phi_pend).^2.*cos(THE_Psi_pend).^2.*sin(THE_Psi).*sin(THE_Theta_pend).*(4.0./3.0)+Lz_pend.^2.*THE_Theta_D.*m_pend.*cos(THE_Psi).*cos(THE_Phi_pend).^2.*cos(THE_Psi_pend).^2.*sin(THE_Theta).*sin(THE_Theta_pend).*(4.0./3.0)-Lz_pend.^2.*THE_Phi_D.*m_pend.*cos(THE_Theta).^2.*cos(THE_Phi_pend).*cos(THE_Psi_pend).^2.*sin(THE_Phi_pend).*sin(THE_Theta_pend).*(4.0./3.0)-Lz_pend.^2.*THE_Psi_D.*m_pend.*cos(THE_Phi_pend).^2.*cos(THE_Psi_pend).*cos(THE_Theta_pend).^2.*sin(THE_Theta).*sin(THE_Psi_pend).*(2.0./3.0)-(Lz_pend.*THE_Phi_D.*Tv_Z_pend.*m_pend.*cos(THE_Psi).^2.*cos(THE_Theta).^2.*cos(THE_Theta_pend).*sin(THE_Psi_pend))./2.0+(Ly_pend.^2.*THE_Theta_D.*m_pend.*cos(THE_Psi).*cos(THE_Theta).*cos(THE_Psi_pend).*sin(THE_Psi).*sin(THE_Psi_pend))./6.0-(Ly_pend.^2.*THE_Phi_D.*m_pend.*cos(THE_Psi).*cos(THE_Theta).*cos(THE_Theta_pend).*sin(THE_Theta).*sin(THE_Phi_pend))./1.2e+1-(Ly_pend.^2.*THE_Theta_pend_D.*m_pend.*cos(THE_Theta).*cos(THE_Phi_pend).*cos(THE_Psi_pend).*sin(THE_Psi).*sin(THE_Psi_pend))./6.0-Lz_pend.^2.*THE_Theta_D.*m_pend.*cos(THE_Psi).*cos(THE_Theta).*cos(THE_Psi_pend).*sin(THE_Psi).*sin(THE_Psi_pend).*(2.0./3.0)+(Lz_pend.^2.*THE_Phi_D.*m_pend.*cos(THE_Psi).*cos(THE_Theta).*cos(THE_Theta_pend).*sin(THE_Theta).*sin(THE_Phi_pend))./3.0+Lz_pend.^2.*THE_Theta_pend_D.*m_pend.*cos(THE_Theta).*cos(THE_Phi_pend).*cos(THE_Psi_pend).*sin(THE_Psi).*sin(THE_Psi_pend).*(2.0./3.0)+(Ly_pend.^2.*THE_Phi_D.*m_pend.*cos(THE_Psi).^2.*cos(THE_Theta).^2.*cos(THE_Phi_pend).^2.*cos(THE_Psi_pend).*sin(THE_Psi_pend))./6.0+(Ly_pend.^2.*THE_Phi_D.*m_pend.*cos(THE_Psi).^2.*cos(THE_Theta).^2.*cos(THE_Psi_pend).*cos(THE_Theta_pend).^2.*sin(THE_Psi_pend))./6.0+(Ly_pend.^2.*THE_Phi_D.*m_pend.*cos(THE_Theta).^2.*cos(THE_Phi_pend).^2.*cos(THE_Psi_pend).*cos(THE_Theta_pend).^2.*sin(THE_Psi_pend))./6.0-Lz_pend.^2.*THE_Phi_D.*m_pend.*cos(THE_Psi).^2.*cos(THE_Theta).^2.*cos(THE_Phi_pend).^2.*cos(THE_Psi_pend).*sin(THE_Psi_pend).*(2.0./3.0)-Lz_pend.^2.*THE_Phi_D.*m_pend.*cos(THE_Psi).^2.*cos(THE_Theta).^2.*cos(THE_Psi_pend).*cos(THE_Theta_pend).^2.*sin(THE_Psi_pend).*(2.0./3.0)-Lz_pend.^2.*THE_Phi_D.*m_pend.*cos(THE_Theta).^2.*cos(THE_Phi_pend).^2.*cos(THE_Psi_pend).*cos(THE_Theta_pend).^2.*sin(THE_Psi_pend).*(2.0./3.0)+Lz_pend.*THE_Psi_D.*Tv_Z_pend.*m_pend.*cos(THE_Psi).*cos(THE_Theta).*cos(THE_Psi_pend).*sin(THE_Phi_pend)-(Ly_pend.^2.*THE_Phi_D.*m_pend.*cos(THE_Psi).*cos(THE_Theta).^2.*cos(THE_Phi_pend).*cos(THE_Theta_pend).*sin(THE_Psi))./1.2e+1-(Ly_pend.^2.*THE_Psi_D.*m_pend.*cos(THE_Psi).*cos(THE_Theta).*cos(THE_Psi_pend).^2.*cos(THE_Theta_pend).*sin(THE_Phi_pend))./6.0+(Ly_pend.^2.*THE_Phi_pend_D.*m_pend.*cos(THE_Theta).*cos(THE_Phi_pend).*cos(THE_Psi_pend).^2.*cos(THE_Theta_pend).*sin(THE_Psi))./6.0+(Ly_pend.^2.*THE_Phi_pend_D.*m_pend.*cos(THE_Psi).*cos(THE_Theta).*cos(THE_Psi_pend).*cos(THE_Theta_pend).^2.*sin(THE_Psi_pend))./6.0+(Lz_pend.^2.*THE_Phi_D.*m_pend.*cos(THE_Psi).*cos(THE_Theta).^2.*cos(THE_Phi_pend).*cos(THE_Theta_pend).*sin(THE_Psi))./3.0+Lz_pend.^2.*THE_Psi_D.*m_pend.*cos(THE_Psi).*cos(THE_Theta).*cos(THE_Psi_pend).^2.*cos(THE_Theta_pend).*sin(THE_Phi_pend).*(2.0./3.0)-Lz_pend.^2.*THE_Phi_pend_D.*m_pend.*cos(THE_Theta).*cos(THE_Phi_pend).*cos(THE_Psi_pend).^2.*cos(THE_Theta_pend).*sin(THE_Psi).*(2.0./3.0)-Lz_pend.^2.*THE_Phi_pend_D.*m_pend.*cos(THE_Psi).*cos(THE_Theta).*cos(THE_Psi_pend).*cos(THE_Theta_pend).^2.*sin(THE_Psi_pend).*(2.0./3.0)+(Ly_pend.^2.*THE_Phi_D.*m_pend.*cos(THE_Theta).*cos(THE_Phi_pend).^2.*sin(THE_Psi).*sin(THE_Theta).*sin(THE_Theta_pend))./6.0+(Ly_pend.^2.*THE_Phi_D.*m_pend.*cos(THE_Theta).*cos(THE_Psi_pend).^2.*sin(THE_Psi).*sin(THE_Theta).*sin(THE_Theta_pend))./6.0-(Ly_pend.^2.*THE_Theta_D.*m_pend.*cos(THE_Psi_pend).^2.*cos(THE_Theta_pend).*sin(THE_Psi).*sin(THE_Theta).*sin(THE_Phi_pend))./6.0+(Ly_pend.^2.*THE_Psi_D.*m_pend.*cos(THE_Phi_pend).*cos(THE_Psi_pend).^2.*sin(THE_Theta).*sin(THE_Phi_pend).*sin(THE_Theta_pend))./3.0+(Ly_pend.^2.*THE_Theta_pend_D.*m_pend.*cos(THE_Theta).*cos(THE_Psi_pend).^2.*sin(THE_Psi).*sin(THE_Phi_pend).*sin(THE_Theta_pend))./6.0-Lz_pend.^2.*THE_Phi_D.*m_pend.*cos(THE_Theta).*cos(THE_Phi_pend).^2.*sin(THE_Psi).*sin(THE_Theta).*sin(THE_Theta_pend).*(2.0./3.0)-Lz_pend.^2.*THE_Phi_D.*m_pend.*cos(THE_Theta).*cos(THE_Psi_pend).^2.*sin(THE_Psi).*sin(THE_Theta).*sin(THE_Theta_pend).*(2.0./3.0)+Lz_pend.^2.*THE_Theta_D.*m_pend.*cos(THE_Psi_pend).^2.*cos(THE_Theta_pend).*sin(THE_Psi).*sin(THE_Theta).*sin(THE_Phi_pend).*(2.0./3.0)-Lz_pend.^2.*THE_Psi_D.*m_pend.*cos(THE_Phi_pend).*cos(THE_Psi_pend).^2.*sin(THE_Theta).*sin(THE_Phi_pend).*sin(THE_Theta_pend).*(4.0./3.0)-Lz_pend.^2.*THE_Theta_pend_D.*m_pend.*cos(THE_Theta).*cos(THE_Psi_pend).^2.*sin(THE_Psi).*sin(THE_Phi_pend).*sin(THE_Theta_pend).*(2.0./3.0)-(Ly_pend.^2.*THE_Phi_D.*m_pend.*cos(THE_Theta).*cos(THE_Phi_pend).^2.*cos(THE_Psi_pend).^2.*sin(THE_Psi).*sin(THE_Theta).*sin(THE_Theta_pend))./3.0+Lz_pend.^2.*THE_Phi_D.*m_pend.*cos(THE_Theta).*cos(THE_Phi_pend).^2.*cos(THE_Psi_pend).^2.*sin(THE_Psi).*sin(THE_Theta).*sin(THE_Theta_pend).*(4.0./3.0)-(Ly_pend.^2.*THE_Theta_D.*m_pend.*cos(THE_Psi).*cos(THE_Theta).*cos(THE_Phi_pend).*sin(THE_Psi).*sin(THE_Phi_pend).*sin(THE_Theta_pend))./6.0+(Ly_pend.^2.*THE_Psi_D.*m_pend.*cos(THE_Theta).*cos(THE_Phi_pend).*cos(THE_Psi_pend).*sin(THE_Psi).*sin(THE_Phi_pend).*sin(THE_Psi_pend))./3.0-(Ly_pend.^2.*THE_Theta_D.*m_pend.*cos(THE_Psi).*cos(THE_Phi_pend).*cos(THE_Psi_pend).*sin(THE_Theta).*sin(THE_Phi_pend).*sin(THE_Psi_pend))./3.0-(Ly_pend.^2.*THE_Theta_D.*m_pend.*cos(THE_Theta).*cos(THE_Psi_pend).*cos(THE_Theta_pend).*sin(THE_Phi_pend).*sin(THE_Psi_pend).*sin(THE_Theta_pend))./6.0-(Ly_pend.^2.*THE_Phi_pend_D.*m_pend.*cos(THE_Phi_pend).*cos(THE_Psi_pend).*cos(THE_Theta_pend).*sin(THE_Theta).*sin(THE_Psi_pend).*sin(THE_Theta_pend))./6.0+Lz_pend.^2.*THE_Theta_D.*m_pend.*cos(THE_Psi).*cos(THE_Theta).*cos(THE_Phi_pend).*sin(THE_Psi).*sin(THE_Phi_pend).*sin(THE_Theta_pend).*(2.0./3.0)-Lz_pend.^2.*THE_Psi_D.*m_pend.*cos(THE_Theta).*cos(THE_Phi_pend).*cos(THE_Psi_pend).*sin(THE_Psi).*sin(THE_Phi_pend).*sin(THE_Psi_pend).*(4.0./3.0)+Lz_pend.^2.*THE_Theta_D.*m_pend.*cos(THE_Psi).*cos(THE_Phi_pend).*cos(THE_Psi_pend).*sin(THE_Theta).*sin(THE_Phi_pend).*sin(THE_Psi_pend).*(4.0./3.0)+Lz_pend.^2.*THE_Theta_D.*m_pend.*cos(THE_Theta).*cos(THE_Psi_pend).*cos(THE_Theta_pend).*sin(THE_Phi_pend).*sin(THE_Psi_pend).*sin(THE_Theta_pend).*(2.0./3.0)+Lz_pend.^2.*THE_Phi_pend_D.*m_pend.*cos(THE_Phi_pend).*cos(THE_Psi_pend).*cos(THE_Theta_pend).*sin(THE_Theta).*sin(THE_Psi_pend).*sin(THE_Theta_pend).*(2.0./3.0)-(Ly_pend.^2.*THE_Phi_D.*m_pend.*cos(THE_Psi).^2.*cos(THE_Theta).^2.*cos(THE_Phi_pend).*cos(THE_Psi_pend).^2.*sin(THE_Phi_pend).*sin(THE_Theta_pend))./6.0+Lz_pend.^2.*THE_Phi_D.*m_pend.*cos(THE_Psi).^2.*cos(THE_Theta).^2.*cos(THE_Phi_pend).*cos(THE_Psi_pend).^2.*sin(THE_Phi_pend).*sin(THE_Theta_pend).*(2.0./3.0)-(Lz_pend.*THE_Phi_D.*Tv_Z_pend.*m_pend.*cos(THE_Psi).*cos(THE_Theta).*cos(THE_Psi_pend).*sin(THE_Theta).*sin(THE_Phi_pend))./2.0+Lz_pend.*THE_Theta_D.*Tv_Z_pend.*m_pend.*cos(THE_Psi).*cos(THE_Theta).*cos(THE_Theta_pend).*sin(THE_Psi).*sin(THE_Psi_pend)-Lz_pend.*THE_Psi_D.*Tv_Z_pend.*m_pend.*cos(THE_Psi).*cos(THE_Theta).*cos(THE_Phi_pend).*sin(THE_Psi_pend).*sin(THE_Theta_pend)-(Ly_pend.^2.*THE_Theta_D.*m_pend.*cos(THE_Psi).*cos(THE_Theta).*cos(THE_Phi_pend).^2.*cos(THE_Psi_pend).*sin(THE_Psi).*sin(THE_Psi_pend))./3.0+(Ly_pend.^2.*THE_Phi_D.*m_pend.*cos(THE_Psi).*cos(THE_Theta).*cos(THE_Psi_pend).^2.*cos(THE_Theta_pend).*sin(THE_Theta).*sin(THE_Phi_pend))./6.0-(Ly_pend.^2.*THE_Theta_D.*m_pend.*cos(THE_Psi).*cos(THE_Theta).*cos(THE_Psi_pend).*cos(THE_Theta_pend).^2.*sin(THE_Psi).*sin(THE_Psi_pend))./3.0+Lz_pend.^2.*THE_Theta_D.*m_pend.*cos(THE_Psi).*cos(THE_Theta).*cos(THE_Phi_pend).^2.*cos(THE_Psi_pend).*sin(THE_Psi).*sin(THE_Psi_pend).*(4.0./3.0)-Lz_pend.^2.*THE_Phi_D.*m_pend.*cos(THE_Psi).*cos(THE_Theta).*cos(THE_Psi_pend).^2.*cos(THE_Theta_pend).*sin(THE_Theta).*sin(THE_Phi_pend).*(2.0./3.0)+Lz_pend.^2.*THE_Theta_D.*m_pend.*cos(THE_Psi).*cos(THE_Theta).*cos(THE_Psi_pend).*cos(THE_Theta_pend).^2.*sin(THE_Psi).*sin(THE_Psi_pend).*(4.0./3.0)-(Ly_pend.^2.*THE_Phi_D.*m_pend.*cos(THE_Psi).^2.*cos(THE_Theta).^2.*cos(THE_Phi_pend).^2.*cos(THE_Psi_pend).*cos(THE_Theta_pend).^2.*sin(THE_Psi_pend))./1.2e+1+(Lz_pend.^2.*THE_Phi_D.*m_pend.*cos(THE_Psi).^2.*cos(THE_Theta).^2.*cos(THE_Phi_pend).^2.*cos(THE_Psi_pend).*cos(THE_Theta_pend).^2.*sin(THE_Psi_pend))./3.0-(Lz_pend.*THE_Phi_D.*Tv_Z_pend.*m_pend.*cos(THE_Psi).*cos(THE_Theta).^2.*cos(THE_Phi_pend).*cos(THE_Psi_pend).*sin(THE_Psi))./2.0-Lz_pend.*THE_Theta_D.*Tv_Z_pend.*m_pend.*cos(THE_Psi).^2.*cos(THE_Theta).*sin(THE_Phi_pend).*sin(THE_Psi_pend).*sin(THE_Theta_pend)+(Ly_pend.^2.*THE_Phi_D.*m_pend.*cos(THE_Psi).*cos(THE_Theta).^2.*cos(THE_Phi_pend).*cos(THE_Psi_pend).^2.*cos(THE_Theta_pend).*sin(THE_Psi))./6.0-Lz_pend.^2.*THE_Phi_D.*m_pend.*cos(THE_Psi).*cos(THE_Theta).^2.*cos(THE_Phi_pend).*cos(THE_Psi_pend).^2.*cos(THE_Theta_pend).*sin(THE_Psi).*(2.0./3.0)-(Ly_pend.^2.*THE_Phi_D.*m_pend.*cos(THE_Theta).*cos(THE_Phi_pend).*cos(THE_Psi_pend).*sin(THE_Psi).*sin(THE_Theta).*sin(THE_Phi_pend).*sin(THE_Psi_pend))./3.0+(Ly_pend.^2.*THE_Theta_D.*m_pend.*cos(THE_Phi_pend).*cos(THE_Psi_pend).*cos(THE_Theta_pend).*sin(THE_Psi).*sin(THE_Theta).*sin(THE_Psi_pend).*sin(THE_Theta_pend))./6.0+(Ly_pend.^2.*THE_Phi_pend_D.*m_pend.*cos(THE_Theta).*cos(THE_Psi_pend).*cos(THE_Theta_pend).*sin(THE_Psi).*sin(THE_Phi_pend).*sin(THE_Psi_pend).*sin(THE_Theta_pend))./6.0+Lz_pend.^2.*THE_Phi_D.*m_pend.*cos(THE_Theta).*cos(THE_Phi_pend).*cos(THE_Psi_pend).*sin(THE_Psi).*sin(THE_Theta).*sin(THE_Phi_pend).*sin(THE_Psi_pend).*(4.0./3.0)-Lz_pend.^2.*THE_Theta_D.*m_pend.*cos(THE_Phi_pend).*cos(THE_Psi_pend).*cos(THE_Theta_pend).*sin(THE_Psi).*sin(THE_Theta).*sin(THE_Psi_pend).*sin(THE_Theta_pend).*(2.0./3.0)-Lz_pend.^2.*THE_Phi_pend_D.*m_pend.*cos(THE_Theta).*cos(THE_Psi_pend).*cos(THE_Theta_pend).*sin(THE_Psi).*sin(THE_Phi_pend).*sin(THE_Psi_pend).*sin(THE_Theta_pend).*(2.0./3.0)+(Lz_pend.*THE_Phi_D.*Tv_Z_pend.*m_pend.*cos(THE_Psi).*cos(THE_Theta).*cos(THE_Phi_pend).*sin(THE_Theta).*sin(THE_Psi_pend).*sin(THE_Theta_pend))./2.0+(Ly_pend.^2.*THE_Theta_D.*m_pend.*cos(THE_Psi).*cos(THE_Theta).*cos(THE_Phi_pend).*cos(THE_Psi_pend).^2.*sin(THE_Psi).*sin(THE_Phi_pend).*sin(THE_Theta_pend))./3.0-(Ly_pend.^2.*THE_Psi_D.*m_pend.*cos(THE_Theta).*cos(THE_Phi_pend).*cos(THE_Psi_pend).*cos(THE_Theta_pend).^2.*sin(THE_Psi).*sin(THE_Phi_pend).*sin(THE_Psi_pend))./6.0+(Ly_pend.^2.*THE_Theta_D.*m_pend.*cos(THE_Psi).*cos(THE_Phi_pend).*cos(THE_Psi_pend).*cos(THE_Theta_pend).^2.*sin(THE_Theta).*sin(THE_Phi_pend).*sin(THE_Psi_pend))./6.0+(Ly_pend.^2.*THE_Theta_D.*m_pend.*cos(THE_Psi).^2.*cos(THE_Theta).*cos(THE_Psi_pend).*cos(THE_Theta_pend).*sin(THE_Phi_pend).*sin(THE_Psi_pend).*sin(THE_Theta_pend))./3.0-Lz_pend.^2.*THE_Theta_D.*m_pend.*cos(THE_Psi).*cos(THE_Theta).*cos(THE_Phi_pend).*cos(THE_Psi_pend).^2.*sin(THE_Psi).*sin(THE_Phi_pend).*sin(THE_Theta_pend).*(4.0./3.0)+Lz_pend.^2.*THE_Psi_D.*m_pend.*cos(THE_Theta).*cos(THE_Phi_pend).*cos(THE_Psi_pend).*cos(THE_Theta_pend).^2.*sin(THE_Psi).*sin(THE_Phi_pend).*sin(THE_Psi_pend).*(2.0./3.0)-Lz_pend.^2.*THE_Theta_D.*m_pend.*cos(THE_Psi).*cos(THE_Phi_pend).*cos(THE_Psi_pend).*cos(THE_Theta_pend).^2.*sin(THE_Theta).*sin(THE_Phi_pend).*sin(THE_Psi_pend).*(2.0./3.0)-Lz_pend.^2.*THE_Theta_D.*m_pend.*cos(THE_Psi).^2.*cos(THE_Theta).*cos(THE_Psi_pend).*cos(THE_Theta_pend).*sin(THE_Phi_pend).*sin(THE_Psi_pend).*sin(THE_Theta_pend).*(4.0./3.0)-(Lz_pend.*THE_Phi_D.*Tv_Z_pend.*m_pend.*cos(THE_Psi).*cos(THE_Theta).^2.*sin(THE_Psi).*sin(THE_Phi_pend).*sin(THE_Psi_pend).*sin(THE_Theta_pend))./2.0+(Ly_pend.^2.*THE_Theta_D.*m_pend.*cos(THE_Psi).*cos(THE_Theta).*cos(THE_Phi_pend).^2.*cos(THE_Psi_pend).*cos(THE_Theta_pend).^2.*sin(THE_Psi).*sin(THE_Psi_pend))./6.0-Lz_pend.^2.*THE_Theta_D.*m_pend.*cos(THE_Psi).*cos(THE_Theta).*cos(THE_Phi_pend).^2.*cos(THE_Psi_pend).*cos(THE_Theta_pend).^2.*sin(THE_Psi).*sin(THE_Psi_pend).*(2.0./3.0)+(Ly_pend.^2.*THE_Psi_D.*m_pend.*cos(THE_Psi).*cos(THE_Theta).*cos(THE_Phi_pend).*cos(THE_Psi_pend).*cos(THE_Theta_pend).*sin(THE_Psi_pend).*sin(THE_Theta_pend))./6.0-Lz_pend.^2.*THE_Psi_D.*m_pend.*cos(THE_Psi).*cos(THE_Theta).*cos(THE_Phi_pend).*cos(THE_Psi_pend).*cos(THE_Theta_pend).*sin(THE_Psi_pend).*sin(THE_Theta_pend).*(2.0./3.0)+(Ly_pend.^2.*THE_Phi_D.*m_pend.*cos(THE_Theta).*cos(THE_Phi_pend).*cos(THE_Psi_pend).*cos(THE_Theta_pend).^2.*sin(THE_Psi).*sin(THE_Theta).*sin(THE_Phi_pend).*sin(THE_Psi_pend))./6.0+(Ly_pend.^2.*THE_Phi_D.*m_pend.*cos(THE_Psi).*cos(THE_Theta).^2.*cos(THE_Psi_pend).*cos(THE_Theta_pend).*sin(THE_Psi).*sin(THE_Phi_pend).*sin(THE_Psi_pend).*sin(THE_Theta_pend))./6.0-Lz_pend.^2.*THE_Phi_D.*m_pend.*cos(THE_Theta).*cos(THE_Phi_pend).*cos(THE_Psi_pend).*cos(THE_Theta_pend).^2.*sin(THE_Psi).*sin(THE_Theta).*sin(THE_Phi_pend).*sin(THE_Psi_pend).*(2.0./3.0)-Lz_pend.^2.*THE_Phi_D.*m_pend.*cos(THE_Psi).*cos(THE_Theta).^2.*cos(THE_Psi_pend).*cos(THE_Theta_pend).*sin(THE_Psi).*sin(THE_Phi_pend).*sin(THE_Psi_pend).*sin(THE_Theta_pend).*(2.0./3.0)-(Ly_pend.^2.*THE_Phi_D.*m_pend.*cos(THE_Psi).*cos(THE_Theta).*cos(THE_Phi_pend).*cos(THE_Psi_pend).*cos(THE_Theta_pend).*sin(THE_Theta).*sin(THE_Psi_pend).*sin(THE_Theta_pend))./6.0+Lz_pend.^2.*THE_Phi_D.*m_pend.*cos(THE_Psi).*cos(THE_Theta).*cos(THE_Phi_pend).*cos(THE_Psi_pend).*cos(THE_Theta_pend).*sin(THE_Theta).*sin(THE_Psi_pend).*sin(THE_Theta_pend).*(2.0./3.0),-I_xx.*THE_Psi_D.*cos(THE_Theta)-I_yy.*THE_Psi_D.*cos(THE_Theta)+I_zz.*THE_Psi_D.*cos(THE_Theta)-Iprop_xx.*THE_Psi_D.*cos(THE_Theta).*4.0-Iprop_yy.*THE_Psi_D.*cos(THE_Theta).*4.0+Iprop_zz.*THE_Psi_D.*cos(THE_Theta).*4.0+I_yz.*THE_Theta_D.*sin(THE_Theta)+Iprop_yz.*THE_Theta_D.*sin(THE_Theta).*4.0-Iprop_xz.*wMOT_1.*cos(THE_Theta)-Iprop_xz.*wMOT_2.*cos(THE_Theta)-Iprop_xz.*wMOT_3.*cos(THE_Theta)-Iprop_xz.*wMOT_4.*cos(THE_Theta)-I_xy.*THE_Theta_D.*cos(THE_Psi).*cos(THE_Theta)-Iprop_xy.*THE_Theta_D.*cos(THE_Psi).*cos(THE_Theta).*4.0+I_xz.*THE_Theta_D.*cos(THE_Theta).*sin(THE_Psi)+Iprop_xz.*THE_Theta_D.*cos(THE_Theta).*sin(THE_Psi).*4.0-(Lx_pend.^2.*THE_Psi_D.*m_pend.*cos(THE_Theta))./6.0-THE_Psi_D.*Tv_Z_pend.^2.*m_pend.*cos(THE_Theta).*2.0-THE_Psi_D.*cg_to_mot_H.^2.*mprop.*cos(THE_Theta).*8.0-Iprop_zz.*wMOT_1.*cos(THE_Psi).*sin(THE_Theta)-Iprop_zz.*wMOT_2.*cos(THE_Psi).*sin(THE_Theta)-Iprop_zz.*wMOT_3.*cos(THE_Psi).*sin(THE_Theta)-Iprop_zz.*wMOT_4.*cos(THE_Psi).*sin(THE_Theta)-Iprop_yz.*wMOT_1.*sin(THE_Psi).*sin(THE_Theta)-Iprop_yz.*wMOT_2.*sin(THE_Psi).*sin(THE_Theta)-Iprop_yz.*wMOT_3.*sin(THE_Psi).*sin(THE_Theta)-Iprop_yz.*wMOT_4.*sin(THE_Psi).*sin(THE_Theta)+I_yy.*THE_Psi_D.*cos(THE_Psi).^2.*cos(THE_Theta).*2.0-I_zz.*THE_Psi_D.*cos(THE_Psi).^2.*cos(THE_Theta).*2.0+Iprop_yy.*THE_Psi_D.*cos(THE_Psi).^2.*cos(THE_Theta).*8.0-Iprop_zz.*THE_Psi_D.*cos(THE_Psi).^2.*cos(THE_Theta).*8.0-I_yz.*THE_Theta_D.*cos(THE_Psi).^2.*sin(THE_Theta).*2.0-Iprop_yz.*THE_Theta_D.*cos(THE_Psi).^2.*sin(THE_Theta).*8.0-I_yz.*THE_Psi_D.*cos(THE_Psi).*cos(THE_Theta).*sin(THE_Psi).*4.0-Iprop_yz.*THE_Psi_D.*cos(THE_Psi).*cos(THE_Theta).*sin(THE_Psi).*1.6e+1-I_yy.*THE_Theta_D.*cos(THE_Psi).*sin(THE_Psi).*sin(THE_Theta)+I_zz.*THE_Theta_D.*cos(THE_Psi).*sin(THE_Psi).*sin(THE_Theta)-Iprop_yy.*THE_Theta_D.*cos(THE_Psi).*sin(THE_Psi).*sin(THE_Theta).*4.0+Iprop_zz.*THE_Theta_D.*cos(THE_Psi).*sin(THE_Psi).*sin(THE_Theta).*4.0+(Lx_pend.^2.*THE_Theta_pend_D.*m_pend.*cos(THE_Theta).*sin(THE_Phi_pend))./6.0-(Ly_pend.^2.*THE_Phi_pend_D.*m_pend.*cos(THE_Psi).*sin(THE_Theta))./6.0+(Lx_pend.^2.*THE_Psi_D.*m_pend.*cos(THE_Psi).^2.*cos(THE_Theta))./6.0+(Lx_pend.^2.*THE_Psi_D.*m_pend.*cos(THE_Theta).*cos(THE_Theta_pend).^2)./6.0-(Ly_pend.^2.*THE_Psi_D.*m_pend.*cos(THE_Psi).^2.*cos(THE_Theta))./6.0-(Ly_pend.^2.*THE_Psi_D.*m_pend.*cos(THE_Theta).*cos(THE_Theta_pend).^2)./6.0+THE_Psi_D.*Tv_Z_pend.^2.*m_pend.*cos(THE_Psi).^2.*cos(THE_Theta).*2.0+THE_Psi_D.*cg_to_mot_H.^2.*mprop.*cos(THE_Psi).^2.*cos(THE_Theta).*8.0-THE_Psi_D.*cg_to_mot_L.^2.*mprop.*cos(THE_Psi).^2.*cos(THE_Theta).*4.0-(Lx_pend.^2.*THE_Theta_D.*m_pend.*cos(THE_Psi).*sin(THE_Psi).*sin(THE_Theta))./1.2e+1-(Lx_pend.^2.*THE_Theta_pend_D.*m_pend.*cos(THE_Phi_pend).*sin(THE_Psi).*sin(THE_Theta))./6.0+(Ly_pend.^2.*THE_Theta_D.*m_pend.*cos(THE_Psi).*sin(THE_Psi).*sin(THE_Theta))./1.2e+1+(Ly_pend.^2.*THE_Psi_pend_D.*m_pend.*cos(THE_Psi).*sin(THE_Theta).*sin(THE_Theta_pend))./6.0-THE_Theta_D.*Tv_Z_pend.^2.*m_pend.*cos(THE_Psi).*sin(THE_Psi).*sin(THE_Theta)-THE_Theta_D.*cg_to_mot_H.^2.*mprop.*cos(THE_Psi).*sin(THE_Psi).*sin(THE_Theta).*4.0+THE_Theta_D.*cg_to_mot_L.^2.*mprop.*cos(THE_Psi).*sin(THE_Psi).*sin(THE_Theta).*2.0-(Lx_pend.^2.*THE_Phi_pend_D.*m_pend.*cos(THE_Psi).*cos(THE_Theta_pend).^2.*sin(THE_Theta))./6.0-(Lx_pend.^2.*THE_Theta_pend_D.*m_pend.*cos(THE_Psi).^2.*cos(THE_Theta).*sin(THE_Phi_pend))./6.0-(Lx_pend.^2.*THE_Theta_pend_D.*m_pend.*cos(THE_Theta).*cos(THE_Theta_pend).^2.*sin(THE_Phi_pend))./6.0+(Ly_pend.^2.*THE_Phi_pend_D.*m_pend.*cos(THE_Psi).*cos(THE_Phi_pend).^2.*sin(THE_Theta))./6.0+(Ly_pend.^2.*THE_Phi_pend_D.*m_pend.*cos(THE_Psi).*cos(THE_Psi_pend).^2.*sin(THE_Theta))./6.0+(Ly_pend.^2.*THE_Phi_pend_D.*m_pend.*cos(THE_Psi).*cos(THE_Theta_pend).^2.*sin(THE_Theta))./6.0+(Ly_pend.^2.*THE_Theta_pend_D.*m_pend.*cos(THE_Psi).^2.*cos(THE_Theta).*sin(THE_Phi_pend))./6.0+(Ly_pend.^2.*THE_Theta_pend_D.*m_pend.*cos(THE_Theta).*cos(THE_Theta_pend).^2.*sin(THE_Phi_pend))./6.0-Lz_pend.^2.*THE_Phi_pend_D.*m_pend.*cos(THE_Psi).*cos(THE_Phi_pend).^2.*sin(THE_Theta).*(2.0./3.0)-Lz_pend.^2.*THE_Phi_pend_D.*m_pend.*cos(THE_Psi).*cos(THE_Psi_pend).^2.*sin(THE_Theta).*(2.0./3.0)-(Lx_pend.^2.*THE_Psi_D.*m_pend.*cos(THE_Psi).^2.*cos(THE_Theta).*cos(THE_Theta_pend).^2)./3.0+(Ly_pend.^2.*THE_Psi_D.*m_pend.*cos(THE_Psi).^2.*cos(THE_Theta).*cos(THE_Phi_pend).^2)./6.0+(Ly_pend.^2.*THE_Psi_D.*m_pend.*cos(THE_Psi).^2.*cos(THE_Theta).*cos(THE_Psi_pend).^2)./6.0+(Ly_pend.^2.*THE_Psi_D.*m_pend.*cos(THE_Psi).^2.*cos(THE_Theta).*cos(THE_Theta_pend).^2)./3.0+(Ly_pend.^2.*THE_Psi_D.*m_pend.*cos(THE_Theta).*cos(THE_Psi_pend).^2.*cos(THE_Theta_pend).^2)./6.0-Lz_pend.^2.*THE_Psi_D.*m_pend.*cos(THE_Psi).^2.*cos(THE_Theta).*cos(THE_Phi_pend).^2.*(2.0./3.0)-Lz_pend.^2.*THE_Psi_D.*m_pend.*cos(THE_Psi).^2.*cos(THE_Theta).*cos(THE_Psi_pend).^2.*(2.0./3.0)-Lz_pend.^2.*THE_Psi_D.*m_pend.*cos(THE_Theta).*cos(THE_Psi_pend).^2.*cos(THE_Theta_pend).^2.*(2.0./3.0)-(Ly_pend.^2.*THE_Psi_pend_D.*m_pend.*cos(THE_Theta).*cos(THE_Phi_pend).*cos(THE_Theta_pend))./6.0+(Lz_pend.*THE_Theta_D.*Tv_Z_pend.*m_pend.*cos(THE_Phi_pend).*sin(THE_Theta).*sin(THE_Psi_pend))./2.0+Lz_pend.*THE_Phi_pend_D.*Tv_Z_pend.*m_pend.*cos(THE_Theta).*sin(THE_Phi_pend).*sin(THE_Psi_pend)+(Ly_pend.^2.*THE_Psi_pend_D.*m_pend.*cos(THE_Psi).^2.*cos(THE_Theta).*cos(THE_Phi_pend).*cos(THE_Theta_pend))./6.0+(Ly_pend.^2.*THE_Psi_pend_D.*m_pend.*cos(THE_Theta).*cos(THE_Phi_pend).*cos(THE_Psi_pend).^2.*cos(THE_Theta_pend))./6.0-Lz_pend.^2.*THE_Psi_pend_D.*m_pend.*cos(THE_Psi).^2.*cos(THE_Theta).*cos(THE_Phi_pend).*cos(THE_Theta_pend).*(2.0./3.0)-Lz_pend.^2.*THE_Psi_pend_D.*m_pend.*cos(THE_Theta).*cos(THE_Phi_pend).*cos(THE_Psi_pend).^2.*cos(THE_Theta_pend).*(2.0./3.0)+(Lx_pend.^2.*THE_Theta_D.*m_pend.*cos(THE_Psi).*cos(THE_Theta_pend).^2.*sin(THE_Psi).*sin(THE_Theta))./6.0+(Lx_pend.^2.*THE_Theta_pend_D.*m_pend.*cos(THE_Phi_pend).*cos(THE_Theta_pend).^2.*sin(THE_Psi).*sin(THE_Theta))./6.0-(Ly_pend.^2.*THE_Theta_D.*m_pend.*cos(THE_Psi).*cos(THE_Phi_pend).^2.*sin(THE_Psi).*sin(THE_Theta))./1.2e+1-(Ly_pend.^2.*THE_Theta_D.*m_pend.*cos(THE_Psi).*cos(THE_Psi_pend).^2.*sin(THE_Psi).*sin(THE_Theta))./1.2e+1-(Ly_pend.^2.*THE_Theta_D.*m_pend.*cos(THE_Psi).*cos(THE_Theta_pend).^2.*sin(THE_Psi).*sin(THE_Theta))./6.0-(Ly_pend.^2.*THE_Psi_pend_D.*m_pend.*cos(THE_Psi).*cos(THE_Phi_pend).^2.*sin(THE_Theta).*sin(THE_Theta_pend))./6.0-(Ly_pend.^2.*THE_Psi_pend_D.*m_pend.*cos(THE_Psi).*cos(THE_Psi_pend).^2.*sin(THE_Theta).*sin(THE_Theta_pend))./6.0-(Ly_pend.^2.*THE_Theta_pend_D.*m_pend.*cos(THE_Phi_pend).*cos(THE_Theta_pend).^2.*sin(THE_Psi).*sin(THE_Theta))./6.0+(Lz_pend.^2.*THE_Theta_D.*m_pend.*cos(THE_Psi).*cos(THE_Phi_pend).^2.*sin(THE_Psi).*sin(THE_Theta))./3.0+(Lz_pend.^2.*THE_Theta_D.*m_pend.*cos(THE_Psi).*cos(THE_Psi_pend).^2.*sin(THE_Psi).*sin(THE_Theta))./3.0+Lz_pend.^2.*THE_Psi_pend_D.*m_pend.*cos(THE_Psi).*cos(THE_Phi_pend).^2.*sin(THE_Theta).*sin(THE_Theta_pend).*(2.0./3.0)+Lz_pend.^2.*THE_Psi_pend_D.*m_pend.*cos(THE_Psi).*cos(THE_Psi_pend).^2.*sin(THE_Theta).*sin(THE_Theta_pend).*(2.0./3.0)+(Lx_pend.^2.*THE_Phi_pend_D.*m_pend.*cos(THE_Psi).*cos(THE_Phi_pend).^2.*cos(THE_Theta_pend).^2.*sin(THE_Theta))./6.0+(Lx_pend.^2.*THE_Theta_pend_D.*m_pend.*cos(THE_Psi).^2.*cos(THE_Theta).*cos(THE_Theta_pend).^2.*sin(THE_Phi_pend))./3.0-(Ly_pend.^2.*THE_Phi_pend_D.*m_pend.*cos(THE_Psi).*cos(THE_Phi_pend).^2.*cos(THE_Psi_pend).^2.*sin(THE_Theta))./3.0-(Ly_pend.^2.*THE_Phi_pend_D.*m_pend.*cos(THE_Psi).*cos(THE_Phi_pend).^2.*cos(THE_Theta_pend).^2.*sin(THE_Theta))./6.0-(Ly_pend.^2.*THE_Phi_pend_D.*m_pend.*cos(THE_Psi).*cos(THE_Psi_pend).^2.*cos(THE_Theta_pend).^2.*sin(THE_Theta))./6.0-(Ly_pend.^2.*THE_Theta_pend_D.*m_pend.*cos(THE_Psi).^2.*cos(THE_Theta).*cos(THE_Psi_pend).^2.*sin(THE_Phi_pend))./6.0-(Ly_pend.^2.*THE_Theta_pend_D.*m_pend.*cos(THE_Psi).^2.*cos(THE_Theta).*cos(THE_Theta_pend).^2.*sin(THE_Phi_pend))./3.0-(Ly_pend.^2.*THE_Theta_pend_D.*m_pend.*cos(THE_Theta).*cos(THE_Psi_pend).^2.*cos(THE_Theta_pend).^2.*sin(THE_Phi_pend))./6.0+Lz_pend.^2.*THE_Phi_pend_D.*m_pend.*cos(THE_Psi).*cos(THE_Phi_pend).^2.*cos(THE_Psi_pend).^2.*sin(THE_Theta).*(4.0./3.0)+Lz_pend.^2.*THE_Phi_pend_D.*m_pend.*cos(THE_Psi).*cos(THE_Psi_pend).^2.*cos(THE_Theta_pend).^2.*sin(THE_Theta).*(2.0./3.0)+Lz_pend.^2.*THE_Theta_pend_D.*m_pend.*cos(THE_Psi).^2.*cos(THE_Theta).*cos(THE_Psi_pend).^2.*sin(THE_Phi_pend).*(2.0./3.0)+Lz_pend.^2.*THE_Theta_pend_D.*m_pend.*cos(THE_Theta).*cos(THE_Psi_pend).^2.*cos(THE_Theta_pend).^2.*sin(THE_Phi_pend).*(2.0./3.0)-(Lx_pend.^2.*THE_Phi_pend_D.*m_pend.*cos(THE_Theta).*cos(THE_Phi_pend).*cos(THE_Theta_pend).*sin(THE_Theta_pend))./6.0+(Ly_pend.^2.*THE_Theta_D.*m_pend.*cos(THE_Psi).*cos(THE_Theta).*cos(THE_Phi_pend).*sin(THE_Phi_pend))./1.2e+1+(Ly_pend.^2.*THE_Phi_pend_D.*m_pend.*cos(THE_Theta).*cos(THE_Phi_pend).*cos(THE_Theta_pend).*sin(THE_Theta_pend))./6.0-(Lz_pend.^2.*THE_Theta_D.*m_pend.*cos(THE_Psi).*cos(THE_Theta).*cos(THE_Phi_pend).*sin(THE_Phi_pend))./3.0+(Lx_pend.^2.*THE_Psi_D.*m_pend.*cos(THE_Psi).^2.*cos(THE_Theta).*cos(THE_Phi_pend).^2.*cos(THE_Theta_pend).^2)./6.0-(Ly_pend.^2.*THE_Psi_D.*m_pend.*cos(THE_Psi).^2.*cos(THE_Theta).*cos(THE_Phi_pend).^2.*cos(THE_Psi_pend).^2)./3.0-(Ly_pend.^2.*THE_Psi_D.*m_pend.*cos(THE_Psi).^2.*cos(THE_Theta).*cos(THE_Phi_pend).^2.*cos(THE_Theta_pend).^2)./6.0-(Ly_pend.^2.*THE_Psi_D.*m_pend.*cos(THE_Psi).^2.*cos(THE_Theta).*cos(THE_Psi_pend).^2.*cos(THE_Theta_pend).^2)./3.0+Lz_pend.^2.*THE_Psi_D.*m_pend.*cos(THE_Psi).^2.*cos(THE_Theta).*cos(THE_Phi_pend).^2.*cos(THE_Psi_pend).^2.*(4.0./3.0)+Lz_pend.^2.*THE_Psi_D.*m_pend.*cos(THE_Psi).^2.*cos(THE_Theta).*cos(THE_Psi_pend).^2.*cos(THE_Theta_pend).^2.*(4.0./3.0)+(Lx_pend.^2.*THE_Theta_D.*m_pend.*cos(THE_Theta_pend).*sin(THE_Theta).*sin(THE_Phi_pend).*sin(THE_Theta_pend))./1.2e+1-(Ly_pend.^2.*THE_Psi_pend_D.*m_pend.*cos(THE_Theta_pend).*sin(THE_Psi).*sin(THE_Theta).*sin(THE_Phi_pend))./6.0-(Ly_pend.^2.*THE_Theta_D.*m_pend.*cos(THE_Theta_pend).*sin(THE_Theta).*sin(THE_Phi_pend).*sin(THE_Theta_pend))./1.2e+1-Lz_pend.*THE_Psi_D.*Tv_Z_pend.*m_pend.*cos(THE_Theta).*cos(THE_Psi_pend).*cos(THE_Theta_pend).*2.0-Lz_pend.*THE_Psi_pend_D.*Tv_Z_pend.*m_pend.*cos(THE_Theta).*cos(THE_Phi_pend).*cos(THE_Psi_pend)+Lz_pend.*THE_Psi_D.*Tv_Z_pend.*m_pend.*cos(THE_Psi).^2.*cos(THE_Theta).*cos(THE_Psi_pend).*cos(THE_Theta_pend).*2.0+Lz_pend.*THE_Psi_pend_D.*Tv_Z_pend.*m_pend.*cos(THE_Psi).^2.*cos(THE_Theta).*cos(THE_Phi_pend).*cos(THE_Psi_pend)-Lz_pend.*THE_Theta_D.*Tv_Z_pend.*m_pend.*cos(THE_Psi).^2.*cos(THE_Phi_pend).*sin(THE_Theta).*sin(THE_Psi_pend)-Lz_pend.*THE_Phi_pend_D.*Tv_Z_pend.*m_pend.*cos(THE_Psi).^2.*cos(THE_Theta).*sin(THE_Phi_pend).*sin(THE_Psi_pend)-(Ly_pend.^2.*THE_Psi_pend_D.*m_pend.*cos(THE_Psi).^2.*cos(THE_Theta).*cos(THE_Phi_pend).*cos(THE_Psi_pend).^2.*cos(THE_Theta_pend))./3.0+Lz_pend.^2.*THE_Psi_pend_D.*m_pend.*cos(THE_Psi).^2.*cos(THE_Theta).*cos(THE_Phi_pend).*cos(THE_Psi_pend).^2.*cos(THE_Theta_pend).*(4.0./3.0)-(Lx_pend.^2.*THE_Theta_D.*m_pend.*cos(THE_Psi).*cos(THE_Phi_pend).^2.*cos(THE_Theta_pend).^2.*sin(THE_Psi).*sin(THE_Theta))./1.2e+1+(Ly_pend.^2.*THE_Theta_D.*m_pend.*cos(THE_Psi).*cos(THE_Phi_pend).^2.*cos(THE_Psi_pend).^2.*sin(THE_Psi).*sin(THE_Theta))./6.0+(Ly_pend.^2.*THE_Theta_D.*m_pend.*cos(THE_Psi).*cos(THE_Phi_pend).^2.*cos(THE_Theta_pend).^2.*sin(THE_Psi).*sin(THE_Theta))./1.2e+1+(Ly_pend.^2.*THE_Theta_D.*m_pend.*cos(THE_Psi).*cos(THE_Psi_pend).^2.*cos(THE_Theta_pend).^2.*sin(THE_Psi).*sin(THE_Theta))./6.0+(Ly_pend.^2.*THE_Psi_pend_D.*m_pend.*cos(THE_Psi).*cos(THE_Phi_pend).^2.*cos(THE_Psi_pend).^2.*sin(THE_Theta).*sin(THE_Theta_pend))./3.0+(Ly_pend.^2.*THE_Theta_pend_D.*m_pend.*cos(THE_Phi_pend).*cos(THE_Psi_pend).^2.*cos(THE_Theta_pend).^2.*sin(THE_Psi).*sin(THE_Theta))./6.0-Lz_pend.^2.*THE_Theta_D.*m_pend.*cos(THE_Psi).*cos(THE_Phi_pend).^2.*cos(THE_Psi_pend).^2.*sin(THE_Psi).*sin(THE_Theta).*(2.0./3.0)-Lz_pend.^2.*THE_Theta_D.*m_pend.*cos(THE_Psi).*cos(THE_Psi_pend).^2.*cos(THE_Theta_pend).^2.*sin(THE_Psi).*sin(THE_Theta).*(2.0./3.0)-Lz_pend.^2.*THE_Psi_pend_D.*m_pend.*cos(THE_Psi).*cos(THE_Phi_pend).^2.*cos(THE_Psi_pend).^2.*sin(THE_Theta).*sin(THE_Theta_pend).*(4.0./3.0)-Lz_pend.^2.*THE_Theta_pend_D.*m_pend.*cos(THE_Phi_pend).*cos(THE_Psi_pend).^2.*cos(THE_Theta_pend).^2.*sin(THE_Psi).*sin(THE_Theta).*(2.0./3.0)+(Lx_pend.^2.*THE_Theta_D.*m_pend.*cos(THE_Theta).*cos(THE_Phi_pend).*cos(THE_Theta_pend).*sin(THE_Psi).*sin(THE_Theta_pend))./1.2e+1+(Lx_pend.^2.*THE_Theta_pend_D.*m_pend.*cos(THE_Psi).*cos(THE_Theta).*cos(THE_Theta_pend).*sin(THE_Psi).*sin(THE_Theta_pend))./3.0-(Ly_pend.^2.*THE_Phi_pend_D.*m_pend.*cos(THE_Psi).*cos(THE_Theta).*cos(THE_Phi_pend).*sin(THE_Psi).*sin(THE_Phi_pend))./6.0-(Ly_pend.^2.*THE_Psi_pend_D.*m_pend.*cos(THE_Psi).*cos(THE_Theta).*cos(THE_Psi_pend).*sin(THE_Psi).*sin(THE_Psi_pend))./6.0-(Ly_pend.^2.*THE_Theta_D.*m_pend.*cos(THE_Psi).*cos(THE_Theta).*cos(THE_Psi_pend).*sin(THE_Psi_pend).*sin(THE_Theta_pend))./1.2e+1-(Ly_pend.^2.*THE_Theta_D.*m_pend.*cos(THE_Theta).*cos(THE_Phi_pend).*cos(THE_Theta_pend).*sin(THE_Psi).*sin(THE_Theta_pend))./1.2e+1-(Ly_pend.^2.*THE_Theta_pend_D.*m_pend.*cos(THE_Psi).*cos(THE_Theta).*cos(THE_Theta_pend).*sin(THE_Psi).*sin(THE_Theta_pend))./3.0-(Ly_pend.^2.*THE_Theta_D.*m_pend.*cos(THE_Phi_pend).*cos(THE_Psi_pend).*cos(THE_Theta_pend).*sin(THE_Theta).*sin(THE_Psi_pend))./1.2e+1-(Ly_pend.^2.*THE_Phi_pend_D.*m_pend.*cos(THE_Theta).*cos(THE_Psi_pend).*cos(THE_Theta_pend).*sin(THE_Phi_pend).*sin(THE_Psi_pend))./6.0+Lz_pend.^2.*THE_Phi_pend_D.*m_pend.*cos(THE_Psi).*cos(THE_Theta).*cos(THE_Phi_pend).*sin(THE_Psi).*sin(THE_Phi_pend).*(2.0./3.0)+Lz_pend.^2.*THE_Psi_pend_D.*m_pend.*cos(THE_Psi).*cos(THE_Theta).*cos(THE_Psi_pend).*sin(THE_Psi).*sin(THE_Psi_pend).*(2.0./3.0)+(Lz_pend.^2.*THE_Theta_D.*m_pend.*cos(THE_Psi).*cos(THE_Theta).*cos(THE_Psi_pend).*sin(THE_Psi_pend).*sin(THE_Theta_pend))./3.0+(Lz_pend.^2.*THE_Theta_D.*m_pend.*cos(THE_Phi_pend).*cos(THE_Psi_pend).*cos(THE_Theta_pend).*sin(THE_Theta).*sin(THE_Psi_pend))./3.0+Lz_pend.^2.*THE_Phi_pend_D.*m_pend.*cos(THE_Theta).*cos(THE_Psi_pend).*cos(THE_Theta_pend).*sin(THE_Phi_pend).*sin(THE_Psi_pend).*(2.0./3.0)+(Ly_pend.^2.*THE_Phi_pend_D.*m_pend.*cos(THE_Psi).*cos(THE_Phi_pend).^2.*cos(THE_Psi_pend).^2.*cos(THE_Theta_pend).^2.*sin(THE_Theta))./6.0+(Ly_pend.^2.*THE_Theta_pend_D.*m_pend.*cos(THE_Psi).^2.*cos(THE_Theta).*cos(THE_Psi_pend).^2.*cos(THE_Theta_pend).^2.*sin(THE_Phi_pend))./3.0-Lz_pend.^2.*THE_Phi_pend_D.*m_pend.*cos(THE_Psi).*cos(THE_Phi_pend).^2.*cos(THE_Psi_pend).^2.*cos(THE_Theta_pend).^2.*sin(THE_Theta).*(2.0./3.0)-Lz_pend.^2.*THE_Theta_pend_D.*m_pend.*cos(THE_Psi).^2.*cos(THE_Theta).*cos(THE_Psi_pend).^2.*cos(THE_Theta_pend).^2.*sin(THE_Phi_pend).*(4.0./3.0)-(Lx_pend.^2.*THE_Phi_pend_D.*m_pend.*cos(THE_Theta_pend).*sin(THE_Psi).*sin(THE_Theta).*sin(THE_Phi_pend).*sin(THE_Theta_pend))./6.0+(Ly_pend.^2.*THE_Phi_pend_D.*m_pend.*cos(THE_Theta_pend).*sin(THE_Psi).*sin(THE_Theta).*sin(THE_Phi_pend).*sin(THE_Theta_pend))./6.0+Lz_pend.*THE_Phi_pend_D.*Tv_Z_pend.*m_pend.*cos(THE_Theta).*cos(THE_Phi_pend).*cos(THE_Psi_pend).*sin(THE_Theta_pend)+Lz_pend.*THE_Theta_pend_D.*Tv_Z_pend.*m_pend.*cos(THE_Theta).*cos(THE_Psi_pend).*cos(THE_Theta_pend).*sin(THE_Phi_pend)-(Lz_pend.*THE_Theta_D.*Tv_Z_pend.*m_pend.*cos(THE_Theta).*sin(THE_Psi).*sin(THE_Phi_pend).*sin(THE_Psi_pend))./2.0-Lz_pend.*THE_Phi_pend_D.*Tv_Z_pend.*m_pend.*cos(THE_Phi_pend).*sin(THE_Psi).*sin(THE_Theta).*sin(THE_Psi_pend)-Lz_pend.*THE_Psi_pend_D.*Tv_Z_pend.*m_pend.*cos(THE_Psi_pend).*sin(THE_Psi).*sin(THE_Theta).*sin(THE_Phi_pend)-(Lz_pend.*THE_Theta_D.*Tv_Z_pend.*m_pend.*cos(THE_Psi_pend).*sin(THE_Theta).*sin(THE_Phi_pend).*sin(THE_Theta_pend))./2.0-Lz_pend.*THE_Psi_pend_D.*Tv_Z_pend.*m_pend.*cos(THE_Theta).*sin(THE_Phi_pend).*sin(THE_Psi_pend).*sin(THE_Theta_pend)+(Lx_pend.^2.*THE_Theta_D.*m_pend.*cos(THE_Psi).*cos(THE_Theta).*cos(THE_Phi_pend).*cos(THE_Theta_pend).^2.*sin(THE_Phi_pend))./1.2e+1+(Lx_pend.^2.*THE_Phi_pend_D.*m_pend.*cos(THE_Psi).^2.*cos(THE_Theta).*cos(THE_Phi_pend).*cos(THE_Theta_pend).*sin(THE_Theta_pend))./6.0-(Ly_pend.^2.*THE_Theta_D.*m_pend.*cos(THE_Psi).*cos(THE_Theta).*cos(THE_Phi_pend).*cos(THE_Psi_pend).^2.*sin(THE_Phi_pend))./6.0-(Ly_pend.^2.*THE_Theta_D.*m_pend.*cos(THE_Psi).*cos(THE_Theta).*cos(THE_Phi_pend).*cos(THE_Theta_pend).^2.*sin(THE_Phi_pend))./1.2e+1-(Ly_pend.^2.*THE_Phi_pend_D.*m_pend.*cos(THE_Psi).^2.*cos(THE_Theta).*cos(THE_Phi_pend).*cos(THE_Theta_pend).*sin(THE_Theta_pend))./6.0-(Ly_pend.^2.*THE_Phi_pend_D.*m_pend.*cos(THE_Theta).*cos(THE_Phi_pend).*cos(THE_Psi_pend).^2.*cos(THE_Theta_pend).*sin(THE_Theta_pend))./6.0+Lz_pend.^2.*THE_Theta_D.*m_pend.*cos(THE_Psi).*cos(THE_Theta).*cos(THE_Phi_pend).*cos(THE_Psi_pend).^2.*sin(THE_Phi_pend).*(2.0./3.0)+Lz_pend.^2.*THE_Phi_pend_D.*m_pend.*cos(THE_Theta).*cos(THE_Phi_pend).*cos(THE_Psi_pend).^2.*cos(THE_Theta_pend).*sin(THE_Theta_pend).*(2.0./3.0)+(Ly_pend.^2.*THE_Psi_D.*m_pend.*cos(THE_Psi).^2.*cos(THE_Theta).*cos(THE_Phi_pend).^2.*cos(THE_Psi_pend).^2.*cos(THE_Theta_pend).^2)./6.0-Lz_pend.^2.*THE_Psi_D.*m_pend.*cos(THE_Psi).^2.*cos(THE_Theta).*cos(THE_Phi_pend).^2.*cos(THE_Psi_pend).^2.*cos(THE_Theta_pend).^2.*(2.0./3.0)-(Lx_pend.^2.*THE_Theta_D.*m_pend.*cos(THE_Psi).^2.*cos(THE_Theta_pend).*sin(THE_Theta).*sin(THE_Phi_pend).*sin(THE_Theta_pend))./6.0+(Ly_pend.^2.*THE_Theta_D.*m_pend.*cos(THE_Psi).^2.*cos(THE_Theta_pend).*sin(THE_Theta).*sin(THE_Phi_pend).*sin(THE_Theta_pend))./6.0+(Ly_pend.^2.*THE_Psi_pend_D.*m_pend.*cos(THE_Psi_pend).^2.*cos(THE_Theta_pend).*sin(THE_Psi).*sin(THE_Theta).*sin(THE_Phi_pend))./6.0+(Ly_pend.^2.*THE_Theta_D.*m_pend.*cos(THE_Psi_pend).^2.*cos(THE_Theta_pend).*sin(THE_Theta).*sin(THE_Phi_pend).*sin(THE_Theta_pend))./1.2e+1-Lz_pend.^2.*THE_Psi_pend_D.*m_pend.*cos(THE_Psi_pend).^2.*cos(THE_Theta_pend).*sin(THE_Psi).*sin(THE_Theta).*sin(THE_Phi_pend).*(2.0./3.0)-(Lz_pend.^2.*THE_Theta_D.*m_pend.*cos(THE_Psi_pend).^2.*cos(THE_Theta_pend).*sin(THE_Theta).*sin(THE_Phi_pend).*sin(THE_Theta_pend))./3.0-(Ly_pend.^2.*THE_Theta_D.*m_pend.*cos(THE_Psi).^2.*cos(THE_Psi_pend).^2.*cos(THE_Theta_pend).*sin(THE_Theta).*sin(THE_Phi_pend).*sin(THE_Theta_pend))./6.0+Lz_pend.^2.*THE_Theta_D.*m_pend.*cos(THE_Psi).^2.*cos(THE_Psi_pend).^2.*cos(THE_Theta_pend).*sin(THE_Theta).*sin(THE_Phi_pend).*sin(THE_Theta_pend).*(2.0./3.0)-(Lx_pend.^2.*THE_Psi_D.*m_pend.*cos(THE_Psi).*cos(THE_Theta).*cos(THE_Theta_pend).*sin(THE_Psi).*sin(THE_Phi_pend).*sin(THE_Theta_pend))./3.0-(Lx_pend.^2.*THE_Theta_pend_D.*m_pend.*cos(THE_Psi).*cos(THE_Phi_pend).*cos(THE_Theta_pend).*sin(THE_Theta).*sin(THE_Phi_pend).*sin(THE_Theta_pend))./6.0+(Ly_pend.^2.*THE_Psi_D.*m_pend.*cos(THE_Psi).*cos(THE_Theta).*cos(THE_Theta_pend).*sin(THE_Psi).*sin(THE_Phi_pend).*sin(THE_Theta_pend))./3.0+(Ly_pend.^2.*THE_Psi_pend_D.*m_pend.*cos(THE_Psi).*cos(THE_Theta).*cos(THE_Phi_pend).*sin(THE_Psi).*sin(THE_Phi_pend).*sin(THE_Theta_pend))./6.0+(Ly_pend.^2.*THE_Phi_pend_D.*m_pend.*cos(THE_Psi).*cos(THE_Theta).*cos(THE_Psi_pend).*sin(THE_Psi).*sin(THE_Psi_pend).*sin(THE_Theta_pend))./6.0+(Ly_pend.^2.*THE_Theta_D.*m_pend.*cos(THE_Theta).*cos(THE_Psi_pend).*cos(THE_Theta_pend).*sin(THE_Psi).*sin(THE_Phi_pend).*sin(THE_Psi_pend))./1.2e+1+(Ly_pend.^2.*THE_Psi_pend_D.*m_pend.*cos(THE_Psi).*cos(THE_Phi_pend).*cos(THE_Psi_pend).*sin(THE_Theta).*sin(THE_Phi_pend).*sin(THE_Psi_pend))./3.0+(Ly_pend.^2.*THE_Phi_pend_D.*m_pend.*cos(THE_Phi_pend).*cos(THE_Psi_pend).*cos(THE_Theta_pend).*sin(THE_Psi).*sin(THE_Theta).*sin(THE_Psi_pend))./6.0+(Ly_pend.^2.*THE_Theta_pend_D.*m_pend.*cos(THE_Psi).*cos(THE_Phi_pend).*cos(THE_Theta_pend).*sin(THE_Theta).*sin(THE_Phi_pend).*sin(THE_Theta_pend))./6.0+(Ly_pend.^2.*THE_Psi_pend_D.*m_pend.*cos(THE_Theta).*cos(THE_Psi_pend).*cos(THE_Theta_pend).*sin(THE_Phi_pend).*sin(THE_Psi_pend).*sin(THE_Theta_pend))./6.0-Lz_pend.^2.*THE_Psi_pend_D.*m_pend.*cos(THE_Psi).*cos(THE_Theta).*cos(THE_Phi_pend).*sin(THE_Psi).*sin(THE_Phi_pend).*sin(THE_Theta_pend).*(2.0./3.0)-Lz_pend.^2.*THE_Phi_pend_D.*m_pend.*cos(THE_Psi).*cos(THE_Theta).*cos(THE_Psi_pend).*sin(THE_Psi).*sin(THE_Psi_pend).*sin(THE_Theta_pend).*(2.0./3.0)-(Lz_pend.^2.*THE_Theta_D.*m_pend.*cos(THE_Theta).*cos(THE_Psi_pend).*cos(THE_Theta_pend).*sin(THE_Psi).*sin(THE_Phi_pend).*sin(THE_Psi_pend))./3.0-Lz_pend.^2.*THE_Psi_pend_D.*m_pend.*cos(THE_Psi).*cos(THE_Phi_pend).*cos(THE_Psi_pend).*sin(THE_Theta).*sin(THE_Phi_pend).*sin(THE_Psi_pend).*(4.0./3.0)-Lz_pend.^2.*THE_Phi_pend_D.*m_pend.*cos(THE_Phi_pend).*cos(THE_Psi_pend).*cos(THE_Theta_pend).*sin(THE_Psi).*sin(THE_Theta).*sin(THE_Psi_pend).*(2.0./3.0)-Lz_pend.^2.*THE_Psi_pend_D.*m_pend.*cos(THE_Theta).*cos(THE_Psi_pend).*cos(THE_Theta_pend).*sin(THE_Phi_pend).*sin(THE_Psi_pend).*sin(THE_Theta_pend).*(2.0./3.0)-(Ly_pend.^2.*THE_Theta_D.*m_pend.*cos(THE_Psi).*cos(THE_Phi_pend).^2.*cos(THE_Psi_pend).^2.*cos(THE_Theta_pend).^2.*sin(THE_Psi).*sin(THE_Theta))./1.2e+1+(Lz_pend.^2.*THE_Theta_D.*m_pend.*cos(THE_Psi).*cos(THE_Phi_pend).^2.*cos(THE_Psi_pend).^2.*cos(THE_Theta_pend).^2.*sin(THE_Psi).*sin(THE_Theta))./3.0-Lz_pend.*THE_Psi_D.*Tv_Z_pend.*m_pend.*cos(THE_Psi).*cos(THE_Theta).*cos(THE_Phi_pend).*sin(THE_Psi).*sin(THE_Psi_pend).*2.0-Lz_pend.*THE_Theta_D.*Tv_Z_pend.*m_pend.*cos(THE_Psi).*cos(THE_Psi_pend).*cos(THE_Theta_pend).*sin(THE_Psi).*sin(THE_Theta)-Lz_pend.*THE_Psi_pend_D.*Tv_Z_pend.*m_pend.*cos(THE_Psi).*cos(THE_Theta).*cos(THE_Theta_pend).*sin(THE_Psi).*sin(THE_Psi_pend)-(Lz_pend.*THE_Theta_D.*Tv_Z_pend.*m_pend.*cos(THE_Theta).*cos(THE_Phi_pend).*cos(THE_Psi_pend).*sin(THE_Psi).*sin(THE_Theta_pend))./2.0-Lz_pend.*THE_Theta_pend_D.*Tv_Z_pend.*m_pend.*cos(THE_Psi).*cos(THE_Theta).*cos(THE_Psi_pend).*sin(THE_Psi).*sin(THE_Theta_pend)-Lz_pend.*THE_Theta_pend_D.*Tv_Z_pend.*m_pend.*cos(THE_Phi_pend).*cos(THE_Psi_pend).*cos(THE_Theta_pend).*sin(THE_Psi).*sin(THE_Theta)+Lz_pend.*THE_Phi_pend_D.*Tv_Z_pend.*m_pend.*cos(THE_Psi_pend).*sin(THE_Psi).*sin(THE_Theta).*sin(THE_Phi_pend).*sin(THE_Theta_pend)+Lz_pend.*THE_Psi_pend_D.*Tv_Z_pend.*m_pend.*cos(THE_Phi_pend).*sin(THE_Psi).*sin(THE_Theta).*sin(THE_Psi_pend).*sin(THE_Theta_pend)-(Lx_pend.^2.*THE_Phi_pend_D.*m_pend.*cos(THE_Psi).*cos(THE_Theta).*cos(THE_Phi_pend).*cos(THE_Theta_pend).^2.*sin(THE_Psi).*sin(THE_Phi_pend))./6.0-(Lx_pend.^2.*THE_Theta_pend_D.*m_pend.*cos(THE_Psi).*cos(THE_Theta).*cos(THE_Phi_pend).^2.*cos(THE_Theta_pend).*sin(THE_Psi).*sin(THE_Theta_pend))./6.0+(Ly_pend.^2.*THE_Phi_pend_D.*m_pend.*cos(THE_Psi).*cos(THE_Theta).*cos(THE_Phi_pend).*cos(THE_Psi_pend).^2.*sin(THE_Psi).*sin(THE_Phi_pend))./3.0+(Ly_pend.^2.*THE_Psi_pend_D.*m_pend.*cos(THE_Psi).*cos(THE_Theta).*cos(THE_Phi_pend).^2.*cos(THE_Psi_pend).*sin(THE_Psi).*sin(THE_Psi_pend))./3.0+(Ly_pend.^2.*THE_Phi_pend_D.*m_pend.*cos(THE_Psi).*cos(THE_Theta).*cos(THE_Phi_pend).*cos(THE_Theta_pend).^2.*sin(THE_Psi).*sin(THE_Phi_pend))./6.0+(Ly_pend.^2.*THE_Psi_pend_D.*m_pend.*cos(THE_Psi).*cos(THE_Theta).*cos(THE_Psi_pend).*cos(THE_Theta_pend).^2.*sin(THE_Psi).*sin(THE_Psi_pend))./3.0+(Ly_pend.^2.*THE_Theta_D.*m_pend.*cos(THE_Psi).*cos(THE_Theta).*cos(THE_Phi_pend).^2.*cos(THE_Psi_pend).*sin(THE_Psi_pend).*sin(THE_Theta_pend))./6.0+(Ly_pend.^2.*THE_Theta_D.*m_pend.*cos(THE_Psi).^2.*cos(THE_Phi_pend).*cos(THE_Psi_pend).*cos(THE_Theta_pend).*sin(THE_Theta).*sin(THE_Psi_pend))./6.0+(Ly_pend.^2.*THE_Theta_D.*m_pend.*cos(THE_Theta).*cos(THE_Phi_pend).*cos(THE_Psi_pend).^2.*cos(THE_Theta_pend).*sin(THE_Psi).*sin(THE_Theta_pend))./1.2e+1+(Ly_pend.^2.*THE_Theta_pend_D.*m_pend.*cos(THE_Psi).*cos(THE_Theta).*cos(THE_Phi_pend).^2.*cos(THE_Theta_pend).*sin(THE_Psi).*sin(THE_Theta_pend))./6.0+(Ly_pend.^2.*THE_Theta_pend_D.*m_pend.*cos(THE_Psi).*cos(THE_Theta).*cos(THE_Psi_pend).^2.*cos(THE_Theta_pend).*sin(THE_Psi).*sin(THE_Theta_pend))./3.0+(Ly_pend.^2.*THE_Phi_pend_D.*m_pend.*cos(THE_Psi).^2.*cos(THE_Theta).*cos(THE_Psi_pend).*cos(THE_Theta_pend).*sin(THE_Phi_pend).*sin(THE_Psi_pend))./6.0+(Ly_pend.^2.*THE_Theta_pend_D.*m_pend.*cos(THE_Psi).*cos(THE_Phi_pend).^2.*cos(THE_Psi_pend).*cos(THE_Theta_pend).*sin(THE_Theta).*sin(THE_Psi_pend))./6.0+(Ly_pend.^2.*THE_Theta_pend_D.*m_pend.*cos(THE_Psi).^2.*cos(THE_Theta).*cos(THE_Phi_pend).*cos(THE_Psi_pend).*sin(THE_Psi_pend).*sin(THE_Theta_pend))./6.0-Lz_pend.^2.*THE_Phi_pend_D.*m_pend.*cos(THE_Psi).*cos(THE_Theta).*cos(THE_Phi_pend).*cos(THE_Psi_pend).^2.*sin(THE_Psi).*sin(THE_Phi_pend).*(4.0./3.0)-Lz_pend.^2.*THE_Psi_pend_D.*m_pend.*cos(THE_Psi).*cos(THE_Theta).*cos(THE_Phi_pend).^2.*cos(THE_Psi_pend).*sin(THE_Psi).*sin(THE_Psi_pend).*(4.0./3.0)-Lz_pend.^2.*THE_Psi_pend_D.*m_pend.*cos(THE_Psi).*cos(THE_Theta).*cos(THE_Psi_pend).*cos(THE_Theta_pend).^2.*sin(THE_Psi).*sin(THE_Psi_pend).*(4.0./3.0)-Lz_pend.^2.*THE_Theta_D.*m_pend.*cos(THE_Psi).*cos(THE_Theta).*cos(THE_Phi_pend).^2.*cos(THE_Psi_pend).*sin(THE_Psi_pend).*sin(THE_Theta_pend).*(2.0./3.0)-Lz_pend.^2.*THE_Theta_D.*m_pend.*cos(THE_Psi).^2.*cos(THE_Phi_pend).*cos(THE_Psi_pend).*cos(THE_Theta_pend).*sin(THE_Theta).*sin(THE_Psi_pend).*(2.0./3.0)-(Lz_pend.^2.*THE_Theta_D.*m_pend.*cos(THE_Theta).*cos(THE_Phi_pend).*cos(THE_Psi_pend).^2.*cos(THE_Theta_pend).*sin(THE_Psi).*sin(THE_Theta_pend))./3.0-Lz_pend.^2.*THE_Theta_pend_D.*m_pend.*cos(THE_Psi).*cos(THE_Theta).*cos(THE_Psi_pend).^2.*cos(THE_Theta_pend).*sin(THE_Psi).*sin(THE_Theta_pend).*(4.0./3.0)-Lz_pend.^2.*THE_Phi_pend_D.*m_pend.*cos(THE_Psi).^2.*cos(THE_Theta).*cos(THE_Psi_pend).*cos(THE_Theta_pend).*sin(THE_Phi_pend).*sin(THE_Psi_pend).*(2.0./3.0)-Lz_pend.^2.*THE_Theta_pend_D.*m_pend.*cos(THE_Psi).*cos(THE_Phi_pend).^2.*cos(THE_Psi_pend).*cos(THE_Theta_pend).*sin(THE_Theta).*sin(THE_Psi_pend).*(2.0./3.0)-Lz_pend.^2.*THE_Theta_pend_D.*m_pend.*cos(THE_Psi).^2.*cos(THE_Theta).*cos(THE_Phi_pend).*cos(THE_Psi_pend).*sin(THE_Psi_pend).*sin(THE_Theta_pend).*(2.0./3.0)-(Ly_pend.^2.*THE_Phi_pend_D.*m_pend.*cos(THE_Psi_pend).^2.*cos(THE_Theta_pend).*sin(THE_Psi).*sin(THE_Theta).*sin(THE_Phi_pend).*sin(THE_Theta_pend))./6.0+Lz_pend.^2.*THE_Phi_pend_D.*m_pend.*cos(THE_Psi_pend).^2.*cos(THE_Theta_pend).*sin(THE_Psi).*sin(THE_Theta).*sin(THE_Phi_pend).*sin(THE_Theta_pend).*(2.0./3.0)-Lz_pend.*THE_Phi_pend_D.*Tv_Z_pend.*m_pend.*cos(THE_Psi).^2.*cos(THE_Theta).*cos(THE_Phi_pend).*cos(THE_Psi_pend).*sin(THE_Theta_pend)-Lz_pend.*THE_Theta_pend_D.*Tv_Z_pend.*m_pend.*cos(THE_Psi).^2.*cos(THE_Theta).*cos(THE_Psi_pend).*cos(THE_Theta_pend).*sin(THE_Phi_pend)+Lz_pend.*THE_Theta_D.*Tv_Z_pend.*m_pend.*cos(THE_Psi).^2.*cos(THE_Psi_pend).*sin(THE_Theta).*sin(THE_Phi_pend).*sin(THE_Theta_pend)+Lz_pend.*THE_Psi_pend_D.*Tv_Z_pend.*m_pend.*cos(THE_Psi).^2.*cos(THE_Theta).*sin(THE_Phi_pend).*sin(THE_Psi_pend).*sin(THE_Theta_pend)+(Ly_pend.^2.*THE_Theta_D.*m_pend.*cos(THE_Psi).*cos(THE_Theta).*cos(THE_Phi_pend).*cos(THE_Psi_pend).^2.*cos(THE_Theta_pend).^2.*sin(THE_Phi_pend))./1.2e+1+(Ly_pend.^2.*THE_Phi_pend_D.*m_pend.*cos(THE_Psi).^2.*cos(THE_Theta).*cos(THE_Phi_pend).*cos(THE_Psi_pend).^2.*cos(THE_Theta_pend).*sin(THE_Theta_pend))./6.0-(Lz_pend.^2.*THE_Theta_D.*m_pend.*cos(THE_Psi).*cos(THE_Theta).*cos(THE_Phi_pend).*cos(THE_Psi_pend).^2.*cos(THE_Theta_pend).^2.*sin(THE_Phi_pend))./3.0-Lz_pend.^2.*THE_Phi_pend_D.*m_pend.*cos(THE_Psi).^2.*cos(THE_Theta).*cos(THE_Phi_pend).*cos(THE_Psi_pend).^2.*cos(THE_Theta_pend).*sin(THE_Theta_pend).*(2.0./3.0)-(Ly_pend.^2.*THE_Phi_pend_D.*m_pend.*cos(THE_Psi).*cos(THE_Phi_pend).*cos(THE_Psi_pend).*sin(THE_Theta).*sin(THE_Phi_pend).*sin(THE_Psi_pend).*sin(THE_Theta_pend))./3.0-(Ly_pend.^2.*THE_Psi_pend_D.*m_pend.*cos(THE_Phi_pend).*cos(THE_Psi_pend).*cos(THE_Theta_pend).*sin(THE_Psi).*sin(THE_Theta).*sin(THE_Psi_pend).*sin(THE_Theta_pend))./6.0+Lz_pend.^2.*THE_Phi_pend_D.*m_pend.*cos(THE_Psi).*cos(THE_Phi_pend).*cos(THE_Psi_pend).*sin(THE_Theta).*sin(THE_Phi_pend).*sin(THE_Psi_pend).*sin(THE_Theta_pend).*(4.0./3.0)+Lz_pend.^2.*THE_Psi_pend_D.*m_pend.*cos(THE_Phi_pend).*cos(THE_Psi_pend).*cos(THE_Theta_pend).*sin(THE_Psi).*sin(THE_Theta).*sin(THE_Psi_pend).*sin(THE_Theta_pend).*(2.0./3.0)+Lz_pend.*THE_Psi_D.*Tv_Z_pend.*m_pend.*cos(THE_Psi).*cos(THE_Theta).*cos(THE_Psi_pend).*sin(THE_Psi).*sin(THE_Phi_pend).*sin(THE_Theta_pend).*2.0-(Ly_pend.^2.*THE_Psi_D.*m_pend.*cos(THE_Psi).*cos(THE_Theta).*cos(THE_Psi_pend).^2.*cos(THE_Theta_pend).*sin(THE_Psi).*sin(THE_Phi_pend).*sin(THE_Theta_pend))./3.0-(Ly_pend.^2.*THE_Psi_D.*m_pend.*cos(THE_Psi).^2.*cos(THE_Theta).*cos(THE_Phi_pend).*cos(THE_Psi_pend).*sin(THE_Phi_pend).*sin(THE_Psi_pend).*sin(THE_Theta_pend))./3.0-(Ly_pend.^2.*THE_Phi_pend_D.*m_pend.*cos(THE_Psi).*cos(THE_Theta).*cos(THE_Phi_pend).^2.*cos(THE_Psi_pend).*sin(THE_Psi).*sin(THE_Psi_pend).*sin(THE_Theta_pend))./3.0-(Ly_pend.^2.*THE_Psi_pend_D.*m_pend.*cos(THE_Psi).*cos(THE_Theta).*cos(THE_Phi_pend).*cos(THE_Psi_pend).^2.*sin(THE_Psi).*sin(THE_Phi_pend).*sin(THE_Theta_pend))./3.0-(Ly_pend.^2.*THE_Psi_pend_D.*m_pend.*cos(THE_Psi).*cos(THE_Phi_pend).*cos(THE_Psi_pend).*cos(THE_Theta_pend).^2.*sin(THE_Theta).*sin(THE_Phi_pend).*sin(THE_Psi_pend))./6.0-(Ly_pend.^2.*THE_Psi_pend_D.*m_pend.*cos(THE_Psi).^2.*cos(THE_Theta).*cos(THE_Psi_pend).*cos(THE_Theta_pend).*sin(THE_Phi_pend).*sin(THE_Psi_pend).*sin(THE_Theta_pend))./3.0-(Ly_pend.^2.*THE_Theta_pend_D.*m_pend.*cos(THE_Psi).*cos(THE_Phi_pend).*cos(THE_Psi_pend).^2.*cos(THE_Theta_pend).*sin(THE_Theta).*sin(THE_Phi_pend).*sin(THE_Theta_pend))./6.0+Lz_pend.^2.*THE_Psi_D.*m_pend.*cos(THE_Psi).*cos(THE_Theta).*cos(THE_Psi_pend).^2.*cos(THE_Theta_pend).*sin(THE_Psi).*sin(THE_Phi_pend).*sin(THE_Theta_pend).*(4.0./3.0)+Lz_pend.^2.*THE_Psi_D.*m_pend.*cos(THE_Psi).^2.*cos(THE_Theta).*cos(THE_Phi_pend).*cos(THE_Psi_pend).*sin(THE_Phi_pend).*sin(THE_Psi_pend).*sin(THE_Theta_pend).*(4.0./3.0)+Lz_pend.^2.*THE_Phi_pend_D.*m_pend.*cos(THE_Psi).*cos(THE_Theta).*cos(THE_Phi_pend).^2.*cos(THE_Psi_pend).*sin(THE_Psi).*sin(THE_Psi_pend).*sin(THE_Theta_pend).*(4.0./3.0)+Lz_pend.^2.*THE_Psi_pend_D.*m_pend.*cos(THE_Psi).*cos(THE_Theta).*cos(THE_Phi_pend).*cos(THE_Psi_pend).^2.*sin(THE_Psi).*sin(THE_Phi_pend).*sin(THE_Theta_pend).*(4.0./3.0)+Lz_pend.^2.*THE_Psi_pend_D.*m_pend.*cos(THE_Psi).*cos(THE_Phi_pend).*cos(THE_Psi_pend).*cos(THE_Theta_pend).^2.*sin(THE_Theta).*sin(THE_Phi_pend).*sin(THE_Psi_pend).*(2.0./3.0)+Lz_pend.^2.*THE_Psi_pend_D.*m_pend.*cos(THE_Psi).^2.*cos(THE_Theta).*cos(THE_Psi_pend).*cos(THE_Theta_pend).*sin(THE_Phi_pend).*sin(THE_Psi_pend).*sin(THE_Theta_pend).*(4.0./3.0)+Lz_pend.^2.*THE_Theta_pend_D.*m_pend.*cos(THE_Psi).*cos(THE_Phi_pend).*cos(THE_Psi_pend).^2.*cos(THE_Theta_pend).*sin(THE_Theta).*sin(THE_Phi_pend).*sin(THE_Theta_pend).*(2.0./3.0)-(Ly_pend.^2.*THE_Phi_pend_D.*m_pend.*cos(THE_Psi).*cos(THE_Theta).*cos(THE_Phi_pend).*cos(THE_Psi_pend).^2.*cos(THE_Theta_pend).^2.*sin(THE_Psi).*sin(THE_Phi_pend))./6.0-(Ly_pend.^2.*THE_Psi_pend_D.*m_pend.*cos(THE_Psi).*cos(THE_Theta).*cos(THE_Phi_pend).^2.*cos(THE_Psi_pend).*cos(THE_Theta_pend).^2.*sin(THE_Psi).*sin(THE_Psi_pend))./6.0-(Ly_pend.^2.*THE_Theta_pend_D.*m_pend.*cos(THE_Psi).*cos(THE_Theta).*cos(THE_Phi_pend).^2.*cos(THE_Psi_pend).^2.*cos(THE_Theta_pend).*sin(THE_Psi).*sin(THE_Theta_pend))./6.0+Lz_pend.^2.*THE_Phi_pend_D.*m_pend.*cos(THE_Psi).*cos(THE_Theta).*cos(THE_Phi_pend).*cos(THE_Psi_pend).^2.*cos(THE_Theta_pend).^2.*sin(THE_Psi).*sin(THE_Phi_pend).*(2.0./3.0)+Lz_pend.^2.*THE_Psi_pend_D.*m_pend.*cos(THE_Psi).*cos(THE_Theta).*cos(THE_Phi_pend).^2.*cos(THE_Psi_pend).*cos(THE_Theta_pend).^2.*sin(THE_Psi).*sin(THE_Psi_pend).*(2.0./3.0)+Lz_pend.^2.*THE_Theta_pend_D.*m_pend.*cos(THE_Psi).*cos(THE_Theta).*cos(THE_Phi_pend).^2.*cos(THE_Psi_pend).^2.*cos(THE_Theta_pend).*sin(THE_Psi).*sin(THE_Theta_pend).*(2.0./3.0)+(Ly_pend.^2.*THE_Psi_D.*m_pend.*cos(THE_Psi).*cos(THE_Theta).*cos(THE_Phi_pend).*cos(THE_Psi_pend).*cos(THE_Theta_pend).*sin(THE_Psi).*sin(THE_Psi_pend))./3.0-Lz_pend.^2.*THE_Psi_D.*m_pend.*cos(THE_Psi).*cos(THE_Theta).*cos(THE_Phi_pend).*cos(THE_Psi_pend).*cos(THE_Theta_pend).*sin(THE_Psi).*sin(THE_Psi_pend).*(4.0./3.0)-(Ly_pend.^2.*THE_Theta_pend_D.*m_pend.*cos(THE_Psi).*cos(THE_Theta).*cos(THE_Phi_pend).*cos(THE_Psi_pend).*cos(THE_Theta_pend).*sin(THE_Psi).*sin(THE_Phi_pend).*sin(THE_Psi_pend))./6.0+Lz_pend.^2.*THE_Theta_pend_D.*m_pend.*cos(THE_Psi).*cos(THE_Theta).*cos(THE_Phi_pend).*cos(THE_Psi_pend).*cos(THE_Theta_pend).*sin(THE_Psi).*sin(THE_Phi_pend).*sin(THE_Psi_pend).*(2.0./3.0)+(Ly_pend.^2.*THE_Theta_D.*m_pend.*cos(THE_Psi).*cos(THE_Phi_pend).*cos(THE_Psi_pend).*sin(THE_Psi).*sin(THE_Theta).*sin(THE_Phi_pend).*sin(THE_Psi_pend).*sin(THE_Theta_pend))./6.0-Lz_pend.^2.*THE_Theta_D.*m_pend.*cos(THE_Psi).*cos(THE_Phi_pend).*cos(THE_Psi_pend).*sin(THE_Psi).*sin(THE_Theta).*sin(THE_Phi_pend).*sin(THE_Psi_pend).*sin(THE_Theta_pend).*(2.0./3.0),I_yz.*THE_Psi_D.*2.0+Iprop_yz.*THE_Psi_D.*8.0-I_yz.*THE_Psi_D.*cos(THE_Psi).^2.*4.0-Iprop_yz.*THE_Psi_D.*cos(THE_Psi).^2.*1.6e+1-I_yy.*THE_Psi_D.*sin(THE_Psi.*2.0)+I_zz.*THE_Psi_D.*sin(THE_Psi.*2.0)-Iprop_yy.*THE_Psi_D.*sin(THE_Psi.*2.0).*4.0+Iprop_zz.*THE_Psi_D.*sin(THE_Psi.*2.0).*4.0-THE_Psi_D.*cg_to_mot_H.^2.*mprop.*sin(THE_Psi.*2.0).*4.0+THE_Psi_D.*cg_to_mot_L.^2.*mprop.*sin(THE_Psi.*2.0).*2.0-(Lx_pend.^2.*THE_Psi_D.*m_pend.*sin(THE_Psi.*2.0))./1.2e+1-(Lx_pend.^2.*THE_Theta_pend_D.*m_pend.*sin(THE_Theta_pend.*2.0))./1.2e+1+(Ly_pend.^2.*THE_Psi_D.*m_pend.*sin(THE_Psi.*2.0))./1.2e+1+(Ly_pend.^2.*THE_Theta_pend_D.*m_pend.*sin(THE_Theta_pend.*2.0))./1.2e+1-THE_Psi_D.*Tv_Z_pend.^2.*m_pend.*sin(THE_Psi.*2.0)+(Lx_pend.^2.*THE_Theta_pend_D.*m_pend.*cos(THE_Psi).*sin(THE_Psi).*sin(THE_Phi_pend))./6.0+(Lx_pend.^2.*THE_Psi_D.*m_pend.*cos(THE_Theta_pend).*sin(THE_Phi_pend).*sin(THE_Theta_pend))./6.0-(Ly_pend.^2.*THE_Theta_pend_D.*m_pend.*cos(THE_Psi).*sin(THE_Psi).*sin(THE_Phi_pend))./6.0-(Ly_pend.^2.*THE_Psi_D.*m_pend.*cos(THE_Theta_pend).*sin(THE_Phi_pend).*sin(THE_Theta_pend))./6.0+Lz_pend.*THE_Psi_D.*Tv_Z_pend.*m_pend.*cos(THE_Phi_pend).*sin(THE_Psi_pend)+(Lx_pend.^2.*THE_Psi_D.*m_pend.*cos(THE_Psi).*cos(THE_Theta_pend).^2.*sin(THE_Psi))./3.0+(Lx_pend.^2.*THE_Theta_pend_D.*m_pend.*cos(THE_Psi).^2.*cos(THE_Theta_pend).*sin(THE_Theta_pend))./3.0-(Ly_pend.^2.*THE_Psi_D.*m_pend.*cos(THE_Psi).*cos(THE_Phi_pend).^2.*sin(THE_Psi))./6.0-(Ly_pend.^2.*THE_Psi_D.*m_pend.*cos(THE_Psi).*cos(THE_Psi_pend).^2.*sin(THE_Psi))./6.0-(Ly_pend.^2.*THE_Psi_D.*m_pend.*cos(THE_Psi).*cos(THE_Theta_pend).^2.*sin(THE_Psi))./3.0-(Ly_pend.^2.*THE_Phi_pend_D.*m_pend.*cos(THE_Psi).^2.*cos(THE_Phi_pend).*sin(THE_Phi_pend))./6.0-(Ly_pend.^2.*THE_Psi_pend_D.*m_pend.*cos(THE_Psi).^2.*cos(THE_Psi_pend).*sin(THE_Psi_pend))./6.0-(Ly_pend.^2.*THE_Theta_pend_D.*m_pend.*cos(THE_Psi).^2.*cos(THE_Theta_pend).*sin(THE_Theta_pend))./3.0-(Ly_pend.^2.*THE_Psi_pend_D.*m_pend.*cos(THE_Psi_pend).*cos(THE_Theta_pend).^2.*sin(THE_Psi_pend))./6.0-(Ly_pend.^2.*THE_Theta_pend_D.*m_pend.*cos(THE_Psi_pend).^2.*cos(THE_Theta_pend).*sin(THE_Theta_pend))./6.0+Lz_pend.^2.*THE_Psi_D.*m_pend.*cos(THE_Psi).*cos(THE_Phi_pend).^2.*sin(THE_Psi).*(2.0./3.0)+Lz_pend.^2.*THE_Psi_D.*m_pend.*cos(THE_Psi).*cos(THE_Psi_pend).^2.*sin(THE_Psi).*(2.0./3.0)+Lz_pend.^2.*THE_Phi_pend_D.*m_pend.*cos(THE_Psi).^2.*cos(THE_Phi_pend).*sin(THE_Phi_pend).*(2.0./3.0)+Lz_pend.^2.*THE_Psi_pend_D.*m_pend.*cos(THE_Psi).^2.*cos(THE_Psi_pend).*sin(THE_Psi_pend).*(2.0./3.0)+Lz_pend.^2.*THE_Psi_pend_D.*m_pend.*cos(THE_Psi_pend).*cos(THE_Theta_pend).^2.*sin(THE_Psi_pend).*(2.0./3.0)+Lz_pend.^2.*THE_Theta_pend_D.*m_pend.*cos(THE_Psi_pend).^2.*cos(THE_Theta_pend).*sin(THE_Theta_pend).*(2.0./3.0)-Lz_pend.*THE_Psi_D.*Tv_Z_pend.*m_pend.*cos(THE_Psi_pend).*sin(THE_Phi_pend).*sin(THE_Theta_pend)-(Lx_pend.^2.*THE_Psi_D.*m_pend.*cos(THE_Psi).^2.*cos(THE_Theta_pend).*sin(THE_Phi_pend).*sin(THE_Theta_pend))./3.0-(Lx_pend.^2.*THE_Theta_pend_D.*m_pend.*cos(THE_Psi).*cos(THE_Theta_pend).^2.*sin(THE_Psi).*sin(THE_Phi_pend))./3.0+(Ly_pend.^2.*THE_Theta_pend_D.*m_pend.*cos(THE_Psi).*cos(THE_Psi_pend).^2.*sin(THE_Psi).*sin(THE_Phi_pend))./6.0+(Ly_pend.^2.*THE_Psi_D.*m_pend.*cos(THE_Psi).^2.*cos(THE_Theta_pend).*sin(THE_Phi_pend).*sin(THE_Theta_pend))./3.0+(Ly_pend.^2.*THE_Theta_pend_D.*m_pend.*cos(THE_Psi).*cos(THE_Theta_pend).^2.*sin(THE_Psi).*sin(THE_Phi_pend))./3.0+(Ly_pend.^2.*THE_Psi_pend_D.*m_pend.*cos(THE_Psi).^2.*cos(THE_Phi_pend).*sin(THE_Phi_pend).*sin(THE_Theta_pend))./6.0+(Ly_pend.^2.*THE_Phi_pend_D.*m_pend.*cos(THE_Psi).^2.*cos(THE_Psi_pend).*sin(THE_Psi_pend).*sin(THE_Theta_pend))./6.0+(Ly_pend.^2.*THE_Psi_D.*m_pend.*cos(THE_Psi_pend).^2.*cos(THE_Theta_pend).*sin(THE_Phi_pend).*sin(THE_Theta_pend))./6.0-Lz_pend.^2.*THE_Theta_pend_D.*m_pend.*cos(THE_Psi).*cos(THE_Psi_pend).^2.*sin(THE_Psi).*sin(THE_Phi_pend).*(2.0./3.0)-Lz_pend.^2.*THE_Psi_pend_D.*m_pend.*cos(THE_Psi).^2.*cos(THE_Phi_pend).*sin(THE_Phi_pend).*sin(THE_Theta_pend).*(2.0./3.0)-Lz_pend.^2.*THE_Phi_pend_D.*m_pend.*cos(THE_Psi).^2.*cos(THE_Psi_pend).*sin(THE_Psi_pend).*sin(THE_Theta_pend).*(2.0./3.0)-Lz_pend.^2.*THE_Psi_D.*m_pend.*cos(THE_Psi_pend).^2.*cos(THE_Theta_pend).*sin(THE_Phi_pend).*sin(THE_Theta_pend).*(2.0./3.0)-Lz_pend.*THE_Psi_D.*Tv_Z_pend.*m_pend.*cos(THE_Psi).^2.*cos(THE_Phi_pend).*sin(THE_Psi_pend).*2.0-Lz_pend.*THE_Psi_pend_D.*Tv_Z_pend.*m_pend.*cos(THE_Psi).^2.*cos(THE_Theta_pend).*sin(THE_Psi_pend)-Lz_pend.*THE_Theta_pend_D.*Tv_Z_pend.*m_pend.*cos(THE_Psi).^2.*cos(THE_Psi_pend).*sin(THE_Theta_pend)-(Lx_pend.^2.*THE_Psi_D.*m_pend.*cos(THE_Psi).*cos(THE_Phi_pend).^2.*cos(THE_Theta_pend).^2.*sin(THE_Psi))./6.0-(Lx_pend.^2.*THE_Phi_pend_D.*m_pend.*cos(THE_Psi).^2.*cos(THE_Phi_pend).*cos(THE_Theta_pend).^2.*sin(THE_Phi_pend))./6.0-(Lx_pend.^2.*THE_Theta_pend_D.*m_pend.*cos(THE_Psi).^2.*cos(THE_Phi_pend).^2.*cos(THE_Theta_pend).*sin(THE_Theta_pend))./6.0+(Ly_pend.^2.*THE_Psi_D.*m_pend.*cos(THE_Psi).*cos(THE_Phi_pend).^2.*cos(THE_Psi_pend).^2.*sin(THE_Psi))./3.0+(Ly_pend.^2.*THE_Psi_D.*m_pend.*cos(THE_Psi).*cos(THE_Phi_pend).^2.*cos(THE_Theta_pend).^2.*sin(THE_Psi))./6.0+(Ly_pend.^2.*THE_Psi_D.*m_pend.*cos(THE_Psi).*cos(THE_Psi_pend).^2.*cos(THE_Theta_pend).^2.*sin(THE_Psi))./3.0+(Ly_pend.^2.*THE_Phi_pend_D.*m_pend.*cos(THE_Psi).^2.*cos(THE_Phi_pend).*cos(THE_Psi_pend).^2.*sin(THE_Phi_pend))./3.0+(Ly_pend.^2.*THE_Psi_pend_D.*m_pend.*cos(THE_Psi).^2.*cos(THE_Phi_pend).^2.*cos(THE_Psi_pend).*sin(THE_Psi_pend))./3.0+(Ly_pend.^2.*THE_Phi_pend_D.*m_pend.*cos(THE_Psi).^2.*cos(THE_Phi_pend).*cos(THE_Theta_pend).^2.*sin(THE_Phi_pend))./6.0+(Ly_pend.^2.*THE_Psi_pend_D.*m_pend.*cos(THE_Psi).^2.*cos(THE_Psi_pend).*cos(THE_Theta_pend).^2.*sin(THE_Psi_pend))./3.0+(Ly_pend.^2.*THE_Theta_pend_D.*m_pend.*cos(THE_Psi).^2.*cos(THE_Phi_pend).^2.*cos(THE_Theta_pend).*sin(THE_Theta_pend))./6.0+(Ly_pend.^2.*THE_Theta_pend_D.*m_pend.*cos(THE_Psi).^2.*cos(THE_Psi_pend).^2.*cos(THE_Theta_pend).*sin(THE_Theta_pend))./3.0-Lz_pend.^2.*THE_Psi_D.*m_pend.*cos(THE_Psi).*cos(THE_Phi_pend).^2.*cos(THE_Psi_pend).^2.*sin(THE_Psi).*(4.0./3.0)-Lz_pend.^2.*THE_Psi_D.*m_pend.*cos(THE_Psi).*cos(THE_Psi_pend).^2.*cos(THE_Theta_pend).^2.*sin(THE_Psi).*(4.0./3.0)-Lz_pend.^2.*THE_Phi_pend_D.*m_pend.*cos(THE_Psi).^2.*cos(THE_Phi_pend).*cos(THE_Psi_pend).^2.*sin(THE_Phi_pend).*(4.0./3.0)-Lz_pend.^2.*THE_Psi_pend_D.*m_pend.*cos(THE_Psi).^2.*cos(THE_Phi_pend).^2.*cos(THE_Psi_pend).*sin(THE_Psi_pend).*(4.0./3.0)-Lz_pend.^2.*THE_Psi_pend_D.*m_pend.*cos(THE_Psi).^2.*cos(THE_Psi_pend).*cos(THE_Theta_pend).^2.*sin(THE_Psi_pend).*(4.0./3.0)-Lz_pend.^2.*THE_Theta_pend_D.*m_pend.*cos(THE_Psi).^2.*cos(THE_Psi_pend).^2.*cos(THE_Theta_pend).*sin(THE_Theta_pend).*(4.0./3.0)-(Ly_pend.^2.*THE_Psi_pend_D.*m_pend.*cos(THE_Psi).*cos(THE_Phi_pend).*cos(THE_Theta_pend).*sin(THE_Psi))./6.0-(Ly_pend.^2.*THE_Psi_D.*m_pend.*cos(THE_Phi_pend).*cos(THE_Psi_pend).*cos(THE_Theta_pend).*sin(THE_Psi_pend))./6.0+Lz_pend.^2.*THE_Psi_pend_D.*m_pend.*cos(THE_Psi).*cos(THE_Phi_pend).*cos(THE_Theta_pend).*sin(THE_Psi).*(2.0./3.0)+Lz_pend.^2.*THE_Psi_D.*m_pend.*cos(THE_Phi_pend).*cos(THE_Psi_pend).*cos(THE_Theta_pend).*sin(THE_Psi_pend).*(2.0./3.0)+Lz_pend.*THE_Psi_D.*Tv_Z_pend.*m_pend.*cos(THE_Psi).^2.*cos(THE_Psi_pend).*sin(THE_Phi_pend).*sin(THE_Theta_pend).*2.0-(Ly_pend.^2.*THE_Psi_D.*m_pend.*cos(THE_Psi).^2.*cos(THE_Psi_pend).^2.*cos(THE_Theta_pend).*sin(THE_Phi_pend).*sin(THE_Theta_pend))./3.0-(Ly_pend.^2.*THE_Theta_pend_D.*m_pend.*cos(THE_Psi).*cos(THE_Psi_pend).^2.*cos(THE_Theta_pend).^2.*sin(THE_Psi).*sin(THE_Phi_pend))./3.0-(Ly_pend.^2.*THE_Phi_pend_D.*m_pend.*cos(THE_Psi).^2.*cos(THE_Phi_pend).^2.*cos(THE_Psi_pend).*sin(THE_Psi_pend).*sin(THE_Theta_pend))./3.0-(Ly_pend.^2.*THE_Psi_pend_D.*m_pend.*cos(THE_Psi).^2.*cos(THE_Phi_pend).*cos(THE_Psi_pend).^2.*sin(THE_Phi_pend).*sin(THE_Theta_pend))./3.0+Lz_pend.^2.*THE_Psi_D.*m_pend.*cos(THE_Psi).^2.*cos(THE_Psi_pend).^2.*cos(THE_Theta_pend).*sin(THE_Phi_pend).*sin(THE_Theta_pend).*(4.0./3.0)+Lz_pend.^2.*THE_Theta_pend_D.*m_pend.*cos(THE_Psi).*cos(THE_Psi_pend).^2.*cos(THE_Theta_pend).^2.*sin(THE_Psi).*sin(THE_Phi_pend).*(4.0./3.0)+Lz_pend.^2.*THE_Phi_pend_D.*m_pend.*cos(THE_Psi).^2.*cos(THE_Phi_pend).^2.*cos(THE_Psi_pend).*sin(THE_Psi_pend).*sin(THE_Theta_pend).*(4.0./3.0)+Lz_pend.^2.*THE_Psi_pend_D.*m_pend.*cos(THE_Psi).^2.*cos(THE_Phi_pend).*cos(THE_Psi_pend).^2.*sin(THE_Phi_pend).*sin(THE_Theta_pend).*(4.0./3.0)-(Lx_pend.^2.*THE_Phi_pend_D.*m_pend.*cos(THE_Psi).*cos(THE_Phi_pend).*cos(THE_Theta_pend).*sin(THE_Psi).*sin(THE_Theta_pend))./6.0+(Ly_pend.^2.*THE_Phi_pend_D.*m_pend.*cos(THE_Psi).*cos(THE_Phi_pend).*cos(THE_Theta_pend).*sin(THE_Psi).*sin(THE_Theta_pend))./6.0-(Ly_pend.^2.*THE_Psi_D.*m_pend.*cos(THE_Psi).*cos(THE_Phi_pend).^2.*cos(THE_Psi_pend).^2.*cos(THE_Theta_pend).^2.*sin(THE_Psi))./6.0-(Ly_pend.^2.*THE_Phi_pend_D.*m_pend.*cos(THE_Psi).^2.*cos(THE_Phi_pend).*cos(THE_Psi_pend).^2.*cos(THE_Theta_pend).^2.*sin(THE_Phi_pend))./6.0-(Ly_pend.^2.*THE_Psi_pend_D.*m_pend.*cos(THE_Psi).^2.*cos(THE_Phi_pend).^2.*cos(THE_Psi_pend).*cos(THE_Theta_pend).^2.*sin(THE_Psi_pend))./6.0-(Ly_pend.^2.*THE_Theta_pend_D.*m_pend.*cos(THE_Psi).^2.*cos(THE_Phi_pend).^2.*cos(THE_Psi_pend).^2.*cos(THE_Theta_pend).*sin(THE_Theta_pend))./6.0+Lz_pend.^2.*THE_Psi_D.*m_pend.*cos(THE_Psi).*cos(THE_Phi_pend).^2.*cos(THE_Psi_pend).^2.*cos(THE_Theta_pend).^2.*sin(THE_Psi).*(2.0./3.0)+Lz_pend.^2.*THE_Phi_pend_D.*m_pend.*cos(THE_Psi).^2.*cos(THE_Phi_pend).*cos(THE_Psi_pend).^2.*cos(THE_Theta_pend).^2.*sin(THE_Phi_pend).*(2.0./3.0)+Lz_pend.^2.*THE_Psi_pend_D.*m_pend.*cos(THE_Psi).^2.*cos(THE_Phi_pend).^2.*cos(THE_Psi_pend).*cos(THE_Theta_pend).^2.*sin(THE_Psi_pend).*(2.0./3.0)+Lz_pend.^2.*THE_Theta_pend_D.*m_pend.*cos(THE_Psi).^2.*cos(THE_Phi_pend).^2.*cos(THE_Psi_pend).^2.*cos(THE_Theta_pend).*sin(THE_Theta_pend).*(2.0./3.0)-Lz_pend.*THE_Psi_D.*Tv_Z_pend.*m_pend.*cos(THE_Psi).*cos(THE_Psi_pend).*cos(THE_Theta_pend).*sin(THE_Psi).*2.0-Lz_pend.*THE_Psi_pend_D.*Tv_Z_pend.*m_pend.*cos(THE_Psi).*cos(THE_Phi_pend).*cos(THE_Psi_pend).*sin(THE_Psi)+Lz_pend.*THE_Phi_pend_D.*Tv_Z_pend.*m_pend.*cos(THE_Psi).*sin(THE_Psi).*sin(THE_Phi_pend).*sin(THE_Psi_pend)+(Ly_pend.^2.*THE_Psi_D.*m_pend.*cos(THE_Psi).^2.*cos(THE_Phi_pend).*cos(THE_Psi_pend).*cos(THE_Theta_pend).*sin(THE_Psi_pend))./3.0+(Ly_pend.^2.*THE_Psi_pend_D.*m_pend.*cos(THE_Psi).*cos(THE_Phi_pend).*cos(THE_Psi_pend).^2.*cos(THE_Theta_pend).*sin(THE_Psi))./3.0-Lz_pend.^2.*THE_Psi_D.*m_pend.*cos(THE_Psi).^2.*cos(THE_Phi_pend).*cos(THE_Psi_pend).*cos(THE_Theta_pend).*sin(THE_Psi_pend).*(4.0./3.0)-Lz_pend.^2.*THE_Psi_pend_D.*m_pend.*cos(THE_Psi).*cos(THE_Phi_pend).*cos(THE_Psi_pend).^2.*cos(THE_Theta_pend).*sin(THE_Psi).*(4.0./3.0)-(Ly_pend.^2.*THE_Phi_pend_D.*m_pend.*cos(THE_Psi).*cos(THE_Psi_pend).*cos(THE_Theta_pend).*sin(THE_Psi).*sin(THE_Phi_pend).*sin(THE_Psi_pend))./6.0-(Ly_pend.^2.*THE_Theta_pend_D.*m_pend.*cos(THE_Psi).*cos(THE_Phi_pend).*cos(THE_Psi_pend).*sin(THE_Psi).*sin(THE_Psi_pend).*sin(THE_Theta_pend))./6.0+Lz_pend.^2.*THE_Phi_pend_D.*m_pend.*cos(THE_Psi).*cos(THE_Psi_pend).*cos(THE_Theta_pend).*sin(THE_Psi).*sin(THE_Phi_pend).*sin(THE_Psi_pend).*(2.0./3.0)+Lz_pend.^2.*THE_Theta_pend_D.*m_pend.*cos(THE_Psi).*cos(THE_Phi_pend).*cos(THE_Psi_pend).*sin(THE_Psi).*sin(THE_Psi_pend).*sin(THE_Theta_pend).*(2.0./3.0)+Lz_pend.*THE_Phi_pend_D.*Tv_Z_pend.*m_pend.*cos(THE_Psi).*cos(THE_Phi_pend).*cos(THE_Psi_pend).*sin(THE_Psi).*sin(THE_Theta_pend)+Lz_pend.*THE_Theta_pend_D.*Tv_Z_pend.*m_pend.*cos(THE_Psi).*cos(THE_Psi_pend).*cos(THE_Theta_pend).*sin(THE_Psi).*sin(THE_Phi_pend)-Lz_pend.*THE_Psi_pend_D.*Tv_Z_pend.*m_pend.*cos(THE_Psi).*sin(THE_Psi).*sin(THE_Phi_pend).*sin(THE_Psi_pend).*sin(THE_Theta_pend)-(Ly_pend.^2.*THE_Phi_pend_D.*m_pend.*cos(THE_Psi).*cos(THE_Phi_pend).*cos(THE_Psi_pend).^2.*cos(THE_Theta_pend).*sin(THE_Psi).*sin(THE_Theta_pend))./6.0-(Ly_pend.^2.*THE_Theta_pend_D.*m_pend.*cos(THE_Psi).^2.*cos(THE_Phi_pend).*cos(THE_Psi_pend).*cos(THE_Theta_pend).*sin(THE_Phi_pend).*sin(THE_Psi_pend))./6.0+Lz_pend.^2.*THE_Phi_pend_D.*m_pend.*cos(THE_Psi).*cos(THE_Phi_pend).*cos(THE_Psi_pend).^2.*cos(THE_Theta_pend).*sin(THE_Psi).*sin(THE_Theta_pend).*(2.0./3.0)+Lz_pend.^2.*THE_Theta_pend_D.*m_pend.*cos(THE_Psi).^2.*cos(THE_Phi_pend).*cos(THE_Psi_pend).*cos(THE_Theta_pend).*sin(THE_Phi_pend).*sin(THE_Psi_pend).*(2.0./3.0)+(Ly_pend.^2.*THE_Psi_D.*m_pend.*cos(THE_Psi).*cos(THE_Phi_pend).*cos(THE_Psi_pend).*sin(THE_Psi).*sin(THE_Phi_pend).*sin(THE_Psi_pend).*sin(THE_Theta_pend))./3.0+(Ly_pend.^2.*THE_Psi_pend_D.*m_pend.*cos(THE_Psi).*cos(THE_Psi_pend).*cos(THE_Theta_pend).*sin(THE_Psi).*sin(THE_Phi_pend).*sin(THE_Psi_pend).*sin(THE_Theta_pend))./3.0-Lz_pend.^2.*THE_Psi_D.*m_pend.*cos(THE_Psi).*cos(THE_Phi_pend).*cos(THE_Psi_pend).*sin(THE_Psi).*sin(THE_Phi_pend).*sin(THE_Psi_pend).*sin(THE_Theta_pend).*(4.0./3.0)-Lz_pend.^2.*THE_Psi_pend_D.*m_pend.*cos(THE_Psi).*cos(THE_Psi_pend).*cos(THE_Theta_pend).*sin(THE_Psi).*sin(THE_Phi_pend).*sin(THE_Psi_pend).*sin(THE_Theta_pend).*(4.0./3.0),-I_yz.*THE_Theta_D-Iprop_yz.*THE_Theta_D.*4.0+I_yz.*THE_Theta_D.*cos(THE_Psi).^2.*2.0+Iprop_yz.*THE_Theta_D.*cos(THE_Psi).^2.*8.0+(I_yy.*THE_Theta_D.*sin(THE_Psi.*2.0))./2.0-(I_zz.*THE_Theta_D.*sin(THE_Psi.*2.0))./2.0+Iprop_yy.*THE_Theta_D.*sin(THE_Psi.*2.0).*2.0-Iprop_zz.*THE_Theta_D.*sin(THE_Psi.*2.0).*2.0+Iprop_zz.*wMOT_1.*cos(THE_Psi)+Iprop_zz.*wMOT_2.*cos(THE_Psi)+Iprop_zz.*wMOT_3.*cos(THE_Psi)+Iprop_zz.*wMOT_4.*cos(THE_Psi)+Iprop_yz.*wMOT_1.*sin(THE_Psi)+Iprop_yz.*wMOT_2.*sin(THE_Psi)+Iprop_yz.*wMOT_3.*sin(THE_Psi)+Iprop_yz.*wMOT_4.*sin(THE_Psi)+THE_Theta_D.*cg_to_mot_H.^2.*mprop.*sin(THE_Psi.*2.0).*2.0-THE_Theta_D.*cg_to_mot_L.^2.*mprop.*sin(THE_Psi.*2.0)+(Ly_pend.^2.*THE_Phi_pend_D.*m_pend.*cos(THE_Psi))./6.0+(Lx_pend.^2.*THE_Theta_D.*m_pend.*sin(THE_Psi.*2.0))./2.4e+1-(Ly_pend.^2.*THE_Theta_D.*m_pend.*sin(THE_Psi.*2.0))./2.4e+1+(THE_Theta_D.*Tv_Z_pend.^2.*m_pend.*sin(THE_Psi.*2.0))./2.0+(Lx_pend.^2.*THE_Theta_pend_D.*m_pend.*cos(THE_Phi_pend).*sin(THE_Psi))./6.0-(Ly_pend.^2.*THE_Psi_pend_D.*m_pend.*cos(THE_Psi).*sin(THE_Theta_pend))./6.0+(Lx_pend.^2.*THE_Phi_pend_D.*m_pend.*cos(THE_Psi).*cos(THE_Theta_pend).^2)./6.0-(Ly_pend.^2.*THE_Phi_pend_D.*m_pend.*cos(THE_Psi).*cos(THE_Phi_pend).^2)./6.0-(Ly_pend.^2.*THE_Phi_pend_D.*m_pend.*cos(THE_Psi).*cos(THE_Psi_pend).^2)./6.0-(Ly_pend.^2.*THE_Phi_pend_D.*m_pend.*cos(THE_Psi).*cos(THE_Theta_pend).^2)./6.0+Lz_pend.^2.*THE_Phi_pend_D.*m_pend.*cos(THE_Psi).*cos(THE_Phi_pend).^2.*(2.0./3.0)+Lz_pend.^2.*THE_Phi_pend_D.*m_pend.*cos(THE_Psi).*cos(THE_Psi_pend).^2.*(2.0./3.0)-(Lx_pend.^2.*THE_Theta_D.*m_pend.*cos(THE_Theta_pend).*sin(THE_Phi_pend).*sin(THE_Theta_pend))./1.2e+1+(Ly_pend.^2.*THE_Psi_pend_D.*m_pend.*cos(THE_Theta_pend).*sin(THE_Psi).*sin(THE_Phi_pend))./6.0+(Ly_pend.^2.*THE_Theta_D.*m_pend.*cos(THE_Theta_pend).*sin(THE_Phi_pend).*sin(THE_Theta_pend))./1.2e+1-(Lz_pend.*THE_Theta_D.*Tv_Z_pend.*m_pend.*cos(THE_Phi_pend).*sin(THE_Psi_pend))./2.0-(Lx_pend.^2.*THE_Theta_D.*m_pend.*cos(THE_Psi).*cos(THE_Theta_pend).^2.*sin(THE_Psi))./6.0-(Lx_pend.^2.*THE_Theta_pend_D.*m_pend.*cos(THE_Phi_pend).*cos(THE_Theta_pend).^2.*sin(THE_Psi))./6.0+(Ly_pend.^2.*THE_Theta_D.*m_pend.*cos(THE_Psi).*cos(THE_Phi_pend).^2.*sin(THE_Psi))./1.2e+1+(Ly_pend.^2.*THE_Theta_D.*m_pend.*cos(THE_Psi).*cos(THE_Psi_pend).^2.*sin(THE_Psi))./1.2e+1+(Ly_pend.^2.*THE_Theta_D.*m_pend.*cos(THE_Psi).*cos(THE_Theta_pend).^2.*sin(THE_Psi))./6.0+(Ly_pend.^2.*THE_Psi_pend_D.*m_pend.*cos(THE_Psi).*cos(THE_Phi_pend).^2.*sin(THE_Theta_pend))./6.0+(Ly_pend.^2.*THE_Psi_pend_D.*m_pend.*cos(THE_Psi).*cos(THE_Psi_pend).^2.*sin(THE_Theta_pend))./6.0+(Ly_pend.^2.*THE_Theta_pend_D.*m_pend.*cos(THE_Phi_pend).*cos(THE_Theta_pend).^2.*sin(THE_Psi))./6.0-(Lz_pend.^2.*THE_Theta_D.*m_pend.*cos(THE_Psi).*cos(THE_Phi_pend).^2.*sin(THE_Psi))./3.0-(Lz_pend.^2.*THE_Theta_D.*m_pend.*cos(THE_Psi).*cos(THE_Psi_pend).^2.*sin(THE_Psi))./3.0-Lz_pend.^2.*THE_Psi_pend_D.*m_pend.*cos(THE_Psi).*cos(THE_Phi_pend).^2.*sin(THE_Theta_pend).*(2.0./3.0)-Lz_pend.^2.*THE_Psi_pend_D.*m_pend.*cos(THE_Psi).*cos(THE_Psi_pend).^2.*sin(THE_Theta_pend).*(2.0./3.0)-(Lx_pend.^2.*THE_Phi_pend_D.*m_pend.*cos(THE_Psi).*cos(THE_Phi_pend).^2.*cos(THE_Theta_pend).^2)./6.0+(Ly_pend.^2.*THE_Phi_pend_D.*m_pend.*cos(THE_Psi).*cos(THE_Phi_pend).^2.*cos(THE_Psi_pend).^2)./3.0+(Ly_pend.^2.*THE_Phi_pend_D.*m_pend.*cos(THE_Psi).*cos(THE_Phi_pend).^2.*cos(THE_Theta_pend).^2)./6.0+(Ly_pend.^2.*THE_Phi_pend_D.*m_pend.*cos(THE_Psi).*cos(THE_Psi_pend).^2.*cos(THE_Theta_pend).^2)./6.0-Lz_pend.^2.*THE_Phi_pend_D.*m_pend.*cos(THE_Psi).*cos(THE_Phi_pend).^2.*cos(THE_Psi_pend).^2.*(4.0./3.0)-Lz_pend.^2.*THE_Phi_pend_D.*m_pend.*cos(THE_Psi).*cos(THE_Psi_pend).^2.*cos(THE_Theta_pend).^2.*(2.0./3.0)+Lz_pend.*THE_Phi_pend_D.*Tv_Z_pend.*m_pend.*cos(THE_Phi_pend).*sin(THE_Psi).*sin(THE_Psi_pend)+Lz_pend.*THE_Psi_pend_D.*Tv_Z_pend.*m_pend.*cos(THE_Psi_pend).*sin(THE_Psi).*sin(THE_Phi_pend)+(Lz_pend.*THE_Theta_D.*Tv_Z_pend.*m_pend.*cos(THE_Psi_pend).*sin(THE_Phi_pend).*sin(THE_Theta_pend))./2.0+(Lx_pend.^2.*THE_Theta_D.*m_pend.*cos(THE_Psi).^2.*cos(THE_Theta_pend).*sin(THE_Phi_pend).*sin(THE_Theta_pend))./6.0-(Ly_pend.^2.*THE_Theta_D.*m_pend.*cos(THE_Psi).^2.*cos(THE_Theta_pend).*sin(THE_Phi_pend).*sin(THE_Theta_pend))./6.0-(Ly_pend.^2.*THE_Psi_pend_D.*m_pend.*cos(THE_Psi_pend).^2.*cos(THE_Theta_pend).*sin(THE_Psi).*sin(THE_Phi_pend))./6.0-(Ly_pend.^2.*THE_Theta_D.*m_pend.*cos(THE_Psi_pend).^2.*cos(THE_Theta_pend).*sin(THE_Phi_pend).*sin(THE_Theta_pend))./1.2e+1+Lz_pend.^2.*THE_Psi_pend_D.*m_pend.*cos(THE_Psi_pend).^2.*cos(THE_Theta_pend).*sin(THE_Psi).*sin(THE_Phi_pend).*(2.0./3.0)+(Lz_pend.^2.*THE_Theta_D.*m_pend.*cos(THE_Psi_pend).^2.*cos(THE_Theta_pend).*sin(THE_Phi_pend).*sin(THE_Theta_pend))./3.0+Lz_pend.*THE_Theta_D.*Tv_Z_pend.*m_pend.*cos(THE_Psi).^2.*cos(THE_Phi_pend).*sin(THE_Psi_pend)+(Lx_pend.^2.*THE_Theta_D.*m_pend.*cos(THE_Psi).*cos(THE_Phi_pend).^2.*cos(THE_Theta_pend).^2.*sin(THE_Psi))./1.2e+1-(Ly_pend.^2.*THE_Theta_D.*m_pend.*cos(THE_Psi).*cos(THE_Phi_pend).^2.*cos(THE_Psi_pend).^2.*sin(THE_Psi))./6.0-(Ly_pend.^2.*THE_Theta_D.*m_pend.*cos(THE_Psi).*cos(THE_Phi_pend).^2.*cos(THE_Theta_pend).^2.*sin(THE_Psi))./1.2e+1-(Ly_pend.^2.*THE_Theta_D.*m_pend.*cos(THE_Psi).*cos(THE_Psi_pend).^2.*cos(THE_Theta_pend).^2.*sin(THE_Psi))./6.0-(Ly_pend.^2.*THE_Psi_pend_D.*m_pend.*cos(THE_Psi).*cos(THE_Phi_pend).^2.*cos(THE_Psi_pend).^2.*sin(THE_Theta_pend))./3.0-(Ly_pend.^2.*THE_Theta_pend_D.*m_pend.*cos(THE_Phi_pend).*cos(THE_Psi_pend).^2.*cos(THE_Theta_pend).^2.*sin(THE_Psi))./6.0+Lz_pend.^2.*THE_Theta_D.*m_pend.*cos(THE_Psi).*cos(THE_Phi_pend).^2.*cos(THE_Psi_pend).^2.*sin(THE_Psi).*(2.0./3.0)+Lz_pend.^2.*THE_Theta_D.*m_pend.*cos(THE_Psi).*cos(THE_Psi_pend).^2.*cos(THE_Theta_pend).^2.*sin(THE_Psi).*(2.0./3.0)+Lz_pend.^2.*THE_Psi_pend_D.*m_pend.*cos(THE_Psi).*cos(THE_Phi_pend).^2.*cos(THE_Psi_pend).^2.*sin(THE_Theta_pend).*(4.0./3.0)+Lz_pend.^2.*THE_Theta_pend_D.*m_pend.*cos(THE_Phi_pend).*cos(THE_Psi_pend).^2.*cos(THE_Theta_pend).^2.*sin(THE_Psi).*(2.0./3.0)+(Ly_pend.^2.*THE_Theta_D.*m_pend.*cos(THE_Phi_pend).*cos(THE_Psi_pend).*cos(THE_Theta_pend).*sin(THE_Psi_pend))./1.2e+1-(Lz_pend.^2.*THE_Theta_D.*m_pend.*cos(THE_Phi_pend).*cos(THE_Psi_pend).*cos(THE_Theta_pend).*sin(THE_Psi_pend))./3.0-(Ly_pend.^2.*THE_Phi_pend_D.*m_pend.*cos(THE_Psi).*cos(THE_Phi_pend).^2.*cos(THE_Psi_pend).^2.*cos(THE_Theta_pend).^2)./6.0+Lz_pend.^2.*THE_Phi_pend_D.*m_pend.*cos(THE_Psi).*cos(THE_Phi_pend).^2.*cos(THE_Psi_pend).^2.*cos(THE_Theta_pend).^2.*(2.0./3.0)+(Lx_pend.^2.*THE_Phi_pend_D.*m_pend.*cos(THE_Theta_pend).*sin(THE_Psi).*sin(THE_Phi_pend).*sin(THE_Theta_pend))./6.0-(Ly_pend.^2.*THE_Phi_pend_D.*m_pend.*cos(THE_Theta_pend).*sin(THE_Psi).*sin(THE_Phi_pend).*sin(THE_Theta_pend))./6.0-Lz_pend.*THE_Theta_D.*Tv_Z_pend.*m_pend.*cos(THE_Psi).^2.*cos(THE_Psi_pend).*sin(THE_Phi_pend).*sin(THE_Theta_pend)+(Ly_pend.^2.*THE_Theta_D.*m_pend.*cos(THE_Psi).^2.*cos(THE_Psi_pend).^2.*cos(THE_Theta_pend).*sin(THE_Phi_pend).*sin(THE_Theta_pend))./6.0-Lz_pend.^2.*THE_Theta_D.*m_pend.*cos(THE_Psi).^2.*cos(THE_Psi_pend).^2.*cos(THE_Theta_pend).*sin(THE_Phi_pend).*sin(THE_Theta_pend).*(2.0./3.0)+(Lx_pend.^2.*THE_Theta_pend_D.*m_pend.*cos(THE_Psi).*cos(THE_Phi_pend).*cos(THE_Theta_pend).*sin(THE_Phi_pend).*sin(THE_Theta_pend))./6.0-(Ly_pend.^2.*THE_Psi_pend_D.*m_pend.*cos(THE_Psi).*cos(THE_Phi_pend).*cos(THE_Psi_pend).*sin(THE_Phi_pend).*sin(THE_Psi_pend))./3.0-(Ly_pend.^2.*THE_Phi_pend_D.*m_pend.*cos(THE_Phi_pend).*cos(THE_Psi_pend).*cos(THE_Theta_pend).*sin(THE_Psi).*sin(THE_Psi_pend))./6.0-(Ly_pend.^2.*THE_Theta_pend_D.*m_pend.*cos(THE_Psi).*cos(THE_Phi_pend).*cos(THE_Theta_pend).*sin(THE_Phi_pend).*sin(THE_Theta_pend))./6.0+Lz_pend.^2.*THE_Psi_pend_D.*m_pend.*cos(THE_Psi).*cos(THE_Phi_pend).*cos(THE_Psi_pend).*sin(THE_Phi_pend).*sin(THE_Psi_pend).*(4.0./3.0)+Lz_pend.^2.*THE_Phi_pend_D.*m_pend.*cos(THE_Phi_pend).*cos(THE_Psi_pend).*cos(THE_Theta_pend).*sin(THE_Psi).*sin(THE_Psi_pend).*(2.0./3.0)+(Ly_pend.^2.*THE_Theta_D.*m_pend.*cos(THE_Psi).*cos(THE_Phi_pend).^2.*cos(THE_Psi_pend).^2.*cos(THE_Theta_pend).^2.*sin(THE_Psi))./1.2e+1-(Lz_pend.^2.*THE_Theta_D.*m_pend.*cos(THE_Psi).*cos(THE_Phi_pend).^2.*cos(THE_Psi_pend).^2.*cos(THE_Theta_pend).^2.*sin(THE_Psi))./3.0+Lz_pend.*THE_Theta_D.*Tv_Z_pend.*m_pend.*cos(THE_Psi).*cos(THE_Psi_pend).*cos(THE_Theta_pend).*sin(THE_Psi)+Lz_pend.*THE_Theta_pend_D.*Tv_Z_pend.*m_pend.*cos(THE_Phi_pend).*cos(THE_Psi_pend).*cos(THE_Theta_pend).*sin(THE_Psi)-Lz_pend.*THE_Phi_pend_D.*Tv_Z_pend.*m_pend.*cos(THE_Psi_pend).*sin(THE_Psi).*sin(THE_Phi_pend).*sin(THE_Theta_pend)-Lz_pend.*THE_Psi_pend_D.*Tv_Z_pend.*m_pend.*cos(THE_Phi_pend).*sin(THE_Psi).*sin(THE_Psi_pend).*sin(THE_Theta_pend)-(Ly_pend.^2.*THE_Theta_D.*m_pend.*cos(THE_Psi).^2.*cos(THE_Phi_pend).*cos(THE_Psi_pend).*cos(THE_Theta_pend).*sin(THE_Psi_pend))./6.0-(Ly_pend.^2.*THE_Theta_pend_D.*m_pend.*cos(THE_Psi).*cos(THE_Phi_pend).^2.*cos(THE_Psi_pend).*cos(THE_Theta_pend).*sin(THE_Psi_pend))./6.0+Lz_pend.^2.*THE_Theta_D.*m_pend.*cos(THE_Psi).^2.*cos(THE_Phi_pend).*cos(THE_Psi_pend).*cos(THE_Theta_pend).*sin(THE_Psi_pend).*(2.0./3.0)+Lz_pend.^2.*THE_Theta_pend_D.*m_pend.*cos(THE_Psi).*cos(THE_Phi_pend).^2.*cos(THE_Psi_pend).*cos(THE_Theta_pend).*sin(THE_Psi_pend).*(2.0./3.0)+(Ly_pend.^2.*THE_Phi_pend_D.*m_pend.*cos(THE_Psi_pend).^2.*cos(THE_Theta_pend).*sin(THE_Psi).*sin(THE_Phi_pend).*sin(THE_Theta_pend))./6.0-Lz_pend.^2.*THE_Phi_pend_D.*m_pend.*cos(THE_Psi_pend).^2.*cos(THE_Theta_pend).*sin(THE_Psi).*sin(THE_Phi_pend).*sin(THE_Theta_pend).*(2.0./3.0)+(Ly_pend.^2.*THE_Phi_pend_D.*m_pend.*cos(THE_Psi).*cos(THE_Phi_pend).*cos(THE_Psi_pend).*sin(THE_Phi_pend).*sin(THE_Psi_pend).*sin(THE_Theta_pend))./3.0+(Ly_pend.^2.*THE_Psi_pend_D.*m_pend.*cos(THE_Phi_pend).*cos(THE_Psi_pend).*cos(THE_Theta_pend).*sin(THE_Psi).*sin(THE_Psi_pend).*sin(THE_Theta_pend))./6.0-Lz_pend.^2.*THE_Phi_pend_D.*m_pend.*cos(THE_Psi).*cos(THE_Phi_pend).*cos(THE_Psi_pend).*sin(THE_Phi_pend).*sin(THE_Psi_pend).*sin(THE_Theta_pend).*(4.0./3.0)-Lz_pend.^2.*THE_Psi_pend_D.*m_pend.*cos(THE_Phi_pend).*cos(THE_Psi_pend).*cos(THE_Theta_pend).*sin(THE_Psi).*sin(THE_Psi_pend).*sin(THE_Theta_pend).*(2.0./3.0)+(Ly_pend.^2.*THE_Psi_pend_D.*m_pend.*cos(THE_Psi).*cos(THE_Phi_pend).*cos(THE_Psi_pend).*cos(THE_Theta_pend).^2.*sin(THE_Phi_pend).*sin(THE_Psi_pend))./6.0+(Ly_pend.^2.*THE_Theta_pend_D.*m_pend.*cos(THE_Psi).*cos(THE_Phi_pend).*cos(THE_Psi_pend).^2.*cos(THE_Theta_pend).*sin(THE_Phi_pend).*sin(THE_Theta_pend))./6.0-Lz_pend.^2.*THE_Psi_pend_D.*m_pend.*cos(THE_Psi).*cos(THE_Phi_pend).*cos(THE_Psi_pend).*cos(THE_Theta_pend).^2.*sin(THE_Phi_pend).*sin(THE_Psi_pend).*(2.0./3.0)-Lz_pend.^2.*THE_Theta_pend_D.*m_pend.*cos(THE_Psi).*cos(THE_Phi_pend).*cos(THE_Psi_pend).^2.*cos(THE_Theta_pend).*sin(THE_Phi_pend).*sin(THE_Theta_pend).*(2.0./3.0)-(Ly_pend.^2.*THE_Theta_D.*m_pend.*cos(THE_Psi).*cos(THE_Phi_pend).*cos(THE_Psi_pend).*sin(THE_Psi).*sin(THE_Phi_pend).*sin(THE_Psi_pend).*sin(THE_Theta_pend))./6.0+Lz_pend.^2.*THE_Theta_D.*m_pend.*cos(THE_Psi).*cos(THE_Phi_pend).*cos(THE_Psi_pend).*sin(THE_Psi).*sin(THE_Phi_pend).*sin(THE_Psi_pend).*sin(THE_Theta_pend).*(2.0./3.0),cos(THE_Phi).*(THE_Psi_D.*cg_to_mot_H.*mprop.*cos(THE_Theta).*sin(THE_Psi).*1.6e+1+THE_Theta_D.*cg_to_mot_H.*mprop.*cos(THE_Psi).*sin(THE_Theta).*8.0+THE_Psi_D.*Tv_Z_pend.*m_pend.*cos(THE_Theta).*sin(THE_Psi).*4.0+THE_Theta_D.*Tv_Z_pend.*m_pend.*cos(THE_Psi).*sin(THE_Theta).*2.0+Lz_pend.*THE_Theta_D.*m_pend.*cos(THE_Theta).*sin(THE_Phi_pend).*sin(THE_Psi_pend)+Lz_pend.*THE_Phi_pend_D.*m_pend.*cos(THE_Phi_pend).*sin(THE_Theta).*sin(THE_Psi_pend).*2.0+Lz_pend.*THE_Psi_pend_D.*m_pend.*cos(THE_Psi_pend).*sin(THE_Theta).*sin(THE_Phi_pend).*2.0+Lz_pend.*THE_Psi_D.*m_pend.*cos(THE_Psi).*cos(THE_Theta).*cos(THE_Phi_pend).*sin(THE_Psi_pend).*2.0+Lz_pend.*THE_Psi_D.*m_pend.*cos(THE_Theta).*cos(THE_Psi_pend).*cos(THE_Theta_pend).*sin(THE_Psi).*2.0+Lz_pend.*THE_Theta_D.*m_pend.*cos(THE_Psi).*cos(THE_Psi_pend).*cos(THE_Theta_pend).*sin(THE_Theta)+Lz_pend.*THE_Psi_pend_D.*m_pend.*cos(THE_Theta).*cos(THE_Phi_pend).*cos(THE_Psi_pend).*sin(THE_Psi).*2.0+Lz_pend.*THE_Psi_pend_D.*m_pend.*cos(THE_Psi).*cos(THE_Theta).*cos(THE_Theta_pend).*sin(THE_Psi_pend).*2.0+Lz_pend.*THE_Theta_D.*m_pend.*cos(THE_Theta).*cos(THE_Phi_pend).*cos(THE_Psi_pend).*sin(THE_Theta_pend)+Lz_pend.*THE_Theta_pend_D.*m_pend.*cos(THE_Psi).*cos(THE_Theta).*cos(THE_Psi_pend).*sin(THE_Theta_pend).*2.0+Lz_pend.*THE_Theta_pend_D.*m_pend.*cos(THE_Phi_pend).*cos(THE_Psi_pend).*cos(THE_Theta_pend).*sin(THE_Theta).*2.0-Lz_pend.*THE_Theta_D.*m_pend.*cos(THE_Phi_pend).*sin(THE_Psi).*sin(THE_Theta).*sin(THE_Psi_pend)-Lz_pend.*THE_Phi_pend_D.*m_pend.*cos(THE_Theta).*sin(THE_Psi).*sin(THE_Phi_pend).*sin(THE_Psi_pend).*2.0-Lz_pend.*THE_Phi_pend_D.*m_pend.*cos(THE_Psi_pend).*sin(THE_Theta).*sin(THE_Phi_pend).*sin(THE_Theta_pend).*2.0-Lz_pend.*THE_Psi_pend_D.*m_pend.*cos(THE_Phi_pend).*sin(THE_Theta).*sin(THE_Psi_pend).*sin(THE_Theta_pend).*2.0-Lz_pend.*THE_Psi_D.*m_pend.*cos(THE_Psi).*cos(THE_Theta).*cos(THE_Psi_pend).*sin(THE_Phi_pend).*sin(THE_Theta_pend).*2.0-Lz_pend.*THE_Phi_pend_D.*m_pend.*cos(THE_Theta).*cos(THE_Phi_pend).*cos(THE_Psi_pend).*sin(THE_Psi).*sin(THE_Theta_pend).*2.0-Lz_pend.*THE_Theta_pend_D.*m_pend.*cos(THE_Theta).*cos(THE_Psi_pend).*cos(THE_Theta_pend).*sin(THE_Psi).*sin(THE_Phi_pend).*2.0+Lz_pend.*THE_Theta_D.*m_pend.*cos(THE_Psi_pend).*sin(THE_Psi).*sin(THE_Theta).*sin(THE_Phi_pend).*sin(THE_Theta_pend)+Lz_pend.*THE_Psi_pend_D.*m_pend.*cos(THE_Theta).*sin(THE_Psi).*sin(THE_Phi_pend).*sin(THE_Psi_pend).*sin(THE_Theta_pend).*2.0).*(-1.0./2.0),sin(THE_Phi).*(THE_Psi_D.*cg_to_mot_H.*mprop.*cos(THE_Theta).*sin(THE_Psi).*1.6e+1+THE_Theta_D.*cg_to_mot_H.*mprop.*cos(THE_Psi).*sin(THE_Theta).*8.0+THE_Psi_D.*Tv_Z_pend.*m_pend.*cos(THE_Theta).*sin(THE_Psi).*4.0+THE_Theta_D.*Tv_Z_pend.*m_pend.*cos(THE_Psi).*sin(THE_Theta).*2.0+Lz_pend.*THE_Theta_D.*m_pend.*cos(THE_Theta).*sin(THE_Phi_pend).*sin(THE_Psi_pend)+Lz_pend.*THE_Phi_pend_D.*m_pend.*cos(THE_Phi_pend).*sin(THE_Theta).*sin(THE_Psi_pend).*2.0+Lz_pend.*THE_Psi_pend_D.*m_pend.*cos(THE_Psi_pend).*sin(THE_Theta).*sin(THE_Phi_pend).*2.0+Lz_pend.*THE_Psi_D.*m_pend.*cos(THE_Psi).*cos(THE_Theta).*cos(THE_Phi_pend).*sin(THE_Psi_pend).*2.0+Lz_pend.*THE_Psi_D.*m_pend.*cos(THE_Theta).*cos(THE_Psi_pend).*cos(THE_Theta_pend).*sin(THE_Psi).*2.0+Lz_pend.*THE_Theta_D.*m_pend.*cos(THE_Psi).*cos(THE_Psi_pend).*cos(THE_Theta_pend).*sin(THE_Theta)+Lz_pend.*THE_Psi_pend_D.*m_pend.*cos(THE_Theta).*cos(THE_Phi_pend).*cos(THE_Psi_pend).*sin(THE_Psi).*2.0+Lz_pend.*THE_Psi_pend_D.*m_pend.*cos(THE_Psi).*cos(THE_Theta).*cos(THE_Theta_pend).*sin(THE_Psi_pend).*2.0+Lz_pend.*THE_Theta_D.*m_pend.*cos(THE_Theta).*cos(THE_Phi_pend).*cos(THE_Psi_pend).*sin(THE_Theta_pend)+Lz_pend.*THE_Theta_pend_D.*m_pend.*cos(THE_Psi).*cos(THE_Theta).*cos(THE_Psi_pend).*sin(THE_Theta_pend).*2.0+Lz_pend.*THE_Theta_pend_D.*m_pend.*cos(THE_Phi_pend).*cos(THE_Psi_pend).*cos(THE_Theta_pend).*sin(THE_Theta).*2.0-Lz_pend.*THE_Theta_D.*m_pend.*cos(THE_Phi_pend).*sin(THE_Psi).*sin(THE_Theta).*sin(THE_Psi_pend)-Lz_pend.*THE_Phi_pend_D.*m_pend.*cos(THE_Theta).*sin(THE_Psi).*sin(THE_Phi_pend).*sin(THE_Psi_pend).*2.0-Lz_pend.*THE_Phi_pend_D.*m_pend.*cos(THE_Psi_pend).*sin(THE_Theta).*sin(THE_Phi_pend).*sin(THE_Theta_pend).*2.0-Lz_pend.*THE_Psi_pend_D.*m_pend.*cos(THE_Phi_pend).*sin(THE_Theta).*sin(THE_Psi_pend).*sin(THE_Theta_pend).*2.0-Lz_pend.*THE_Psi_D.*m_pend.*cos(THE_Psi).*cos(THE_Theta).*cos(THE_Psi_pend).*sin(THE_Phi_pend).*sin(THE_Theta_pend).*2.0-Lz_pend.*THE_Phi_pend_D.*m_pend.*cos(THE_Theta).*cos(THE_Phi_pend).*cos(THE_Psi_pend).*sin(THE_Psi).*sin(THE_Theta_pend).*2.0-Lz_pend.*THE_Theta_pend_D.*m_pend.*cos(THE_Theta).*cos(THE_Psi_pend).*cos(THE_Theta_pend).*sin(THE_Psi).*sin(THE_Phi_pend).*2.0+Lz_pend.*THE_Theta_D.*m_pend.*cos(THE_Psi_pend).*sin(THE_Psi).*sin(THE_Theta).*sin(THE_Phi_pend).*sin(THE_Theta_pend)+Lz_pend.*THE_Psi_pend_D.*m_pend.*cos(THE_Theta).*sin(THE_Psi).*sin(THE_Phi_pend).*sin(THE_Psi_pend).*sin(THE_Theta_pend).*2.0).*(-1.0./2.0),THE_Psi_D.*Tv_Z_pend.*m_pend.*sin(THE_Psi).*sin(THE_Theta).*2.0+THE_Psi_D.*cg_to_mot_H.*mprop.*sin(THE_Psi).*sin(THE_Theta).*8.0-THE_Theta_D.*Tv_Z_pend.*m_pend.*cos(THE_Psi).*cos(THE_Theta)-THE_Theta_D.*cg_to_mot_H.*mprop.*cos(THE_Psi).*cos(THE_Theta).*4.0-Lz_pend.*THE_Phi_pend_D.*m_pend.*cos(THE_Theta).*cos(THE_Phi_pend).*sin(THE_Psi_pend)-Lz_pend.*THE_Psi_pend_D.*m_pend.*cos(THE_Theta).*cos(THE_Psi_pend).*sin(THE_Phi_pend)+(Lz_pend.*THE_Theta_D.*m_pend.*sin(THE_Theta).*sin(THE_Phi_pend).*sin(THE_Psi_pend))./2.0-(Lz_pend.*THE_Theta_D.*m_pend.*cos(THE_Psi).*cos(THE_Theta).*cos(THE_Psi_pend).*cos(THE_Theta_pend))./2.0-Lz_pend.*THE_Theta_pend_D.*m_pend.*cos(THE_Theta).*cos(THE_Phi_pend).*cos(THE_Psi_pend).*cos(THE_Theta_pend)+Lz_pend.*THE_Psi_D.*m_pend.*cos(THE_Psi).*cos(THE_Phi_pend).*sin(THE_Theta).*sin(THE_Psi_pend)+(Lz_pend.*THE_Theta_D.*m_pend.*cos(THE_Theta).*cos(THE_Phi_pend).*sin(THE_Psi).*sin(THE_Psi_pend))./2.0+Lz_pend.*THE_Psi_D.*m_pend.*cos(THE_Psi_pend).*cos(THE_Theta_pend).*sin(THE_Psi).*sin(THE_Theta)+Lz_pend.*THE_Psi_pend_D.*m_pend.*cos(THE_Phi_pend).*cos(THE_Psi_pend).*sin(THE_Psi).*sin(THE_Theta)+Lz_pend.*THE_Psi_pend_D.*m_pend.*cos(THE_Psi).*cos(THE_Theta_pend).*sin(THE_Theta).*sin(THE_Psi_pend)+(Lz_pend.*THE_Theta_D.*m_pend.*cos(THE_Phi_pend).*cos(THE_Psi_pend).*sin(THE_Theta).*sin(THE_Theta_pend))./2.0+Lz_pend.*THE_Theta_pend_D.*m_pend.*cos(THE_Psi).*cos(THE_Psi_pend).*sin(THE_Theta).*sin(THE_Theta_pend)+Lz_pend.*THE_Phi_pend_D.*m_pend.*cos(THE_Theta).*cos(THE_Psi_pend).*sin(THE_Phi_pend).*sin(THE_Theta_pend)+Lz_pend.*THE_Psi_pend_D.*m_pend.*cos(THE_Theta).*cos(THE_Phi_pend).*sin(THE_Psi_pend).*sin(THE_Theta_pend)-Lz_pend.*THE_Phi_pend_D.*m_pend.*sin(THE_Psi).*sin(THE_Theta).*sin(THE_Phi_pend).*sin(THE_Psi_pend)-Lz_pend.*THE_Psi_D.*m_pend.*cos(THE_Psi).*cos(THE_Psi_pend).*sin(THE_Theta).*sin(THE_Phi_pend).*sin(THE_Theta_pend)-(Lz_pend.*THE_Theta_D.*m_pend.*cos(THE_Theta).*cos(THE_Psi_pend).*sin(THE_Psi).*sin(THE_Phi_pend).*sin(THE_Theta_pend))./2.0-Lz_pend.*THE_Phi_pend_D.*m_pend.*cos(THE_Phi_pend).*cos(THE_Psi_pend).*sin(THE_Psi).*sin(THE_Theta).*sin(THE_Theta_pend)-Lz_pend.*THE_Theta_pend_D.*m_pend.*cos(THE_Psi_pend).*cos(THE_Theta_pend).*sin(THE_Psi).*sin(THE_Theta).*sin(THE_Phi_pend)+Lz_pend.*THE_Psi_pend_D.*m_pend.*sin(THE_Psi).*sin(THE_Theta).*sin(THE_Phi_pend).*sin(THE_Psi_pend).*sin(THE_Theta_pend),Ly_pend.^2.*THE_Psi_D.*m_pend.*cos(THE_Psi).*(-1.0./6.0)+(Ly_pend.^2.*THE_Theta_pend_D.*m_pend.*cos(THE_Psi).*sin(THE_Phi_pend))./6.0-(Lx_pend.^2.*THE_Psi_D.*m_pend.*cos(THE_Psi).*cos(THE_Theta_pend).^2)./6.0+(Ly_pend.^2.*THE_Psi_D.*m_pend.*cos(THE_Psi).*cos(THE_Phi_pend).^2)./6.0+(Ly_pend.^2.*THE_Psi_D.*m_pend.*cos(THE_Psi).*cos(THE_Psi_pend).^2)./6.0+(Ly_pend.^2.*THE_Psi_D.*m_pend.*cos(THE_Psi).*cos(THE_Theta_pend).^2)./6.0-Lz_pend.^2.*THE_Psi_D.*m_pend.*cos(THE_Psi).*cos(THE_Phi_pend).^2.*(2.0./3.0)-Lz_pend.^2.*THE_Psi_D.*m_pend.*cos(THE_Psi).*cos(THE_Psi_pend).^2.*(2.0./3.0)+(Lx_pend.^2.*THE_Theta_pend_D.*m_pend.*cos(THE_Theta_pend).*sin(THE_Psi).*sin(THE_Theta_pend))./6.0-(Ly_pend.^2.*THE_Theta_pend_D.*m_pend.*cos(THE_Theta_pend).*sin(THE_Psi).*sin(THE_Theta_pend))./6.0+(Lx_pend.^2.*THE_Theta_pend_D.*m_pend.*cos(THE_Psi).*cos(THE_Theta_pend).^2.*sin(THE_Phi_pend))./6.0+(Ly_pend.^2.*THE_Theta_D.*m_pend.*cos(THE_Psi).^2.*cos(THE_Phi_pend).*sin(THE_Phi_pend))./1.2e+1-(Ly_pend.^2.*THE_Theta_pend_D.*m_pend.*cos(THE_Psi).*cos(THE_Psi_pend).^2.*sin(THE_Phi_pend))./6.0-(Ly_pend.^2.*THE_Theta_pend_D.*m_pend.*cos(THE_Psi).*cos(THE_Theta_pend).^2.*sin(THE_Phi_pend))./6.0-(Lz_pend.^2.*THE_Theta_D.*m_pend.*cos(THE_Psi).^2.*cos(THE_Phi_pend).*sin(THE_Phi_pend))./3.0+Lz_pend.^2.*THE_Theta_pend_D.*m_pend.*cos(THE_Psi).*cos(THE_Psi_pend).^2.*sin(THE_Phi_pend).*(2.0./3.0)+(Lx_pend.^2.*THE_Psi_D.*m_pend.*cos(THE_Psi).*cos(THE_Phi_pend).^2.*cos(THE_Theta_pend).^2)./6.0-(Ly_pend.^2.*THE_Psi_D.*m_pend.*cos(THE_Psi).*cos(THE_Phi_pend).^2.*cos(THE_Psi_pend).^2)./3.0-(Ly_pend.^2.*THE_Psi_D.*m_pend.*cos(THE_Psi).*cos(THE_Phi_pend).^2.*cos(THE_Theta_pend).^2)./6.0-(Ly_pend.^2.*THE_Psi_D.*m_pend.*cos(THE_Psi).*cos(THE_Psi_pend).^2.*cos(THE_Theta_pend).^2)./6.0+Lz_pend.^2.*THE_Psi_D.*m_pend.*cos(THE_Psi).*cos(THE_Phi_pend).^2.*cos(THE_Psi_pend).^2.*(4.0./3.0)+Lz_pend.^2.*THE_Psi_D.*m_pend.*cos(THE_Psi).*cos(THE_Psi_pend).^2.*cos(THE_Theta_pend).^2.*(2.0./3.0)-Lz_pend.^2.*THE_Psi_pend_D.*m_pend.*cos(THE_Psi).*cos(THE_Phi_pend).*cos(THE_Theta_pend).*(2.0./3.0)-Lz_pend.*THE_Psi_D.*Tv_Z_pend.*m_pend.*cos(THE_Phi_pend).*sin(THE_Psi).*sin(THE_Psi_pend)-(Ly_pend.^2.*THE_Psi_pend_D.*m_pend.*cos(THE_Psi).*cos(THE_Phi_pend).*cos(THE_Psi_pend).^2.*cos(THE_Theta_pend))./6.0+Lz_pend.^2.*THE_Psi_pend_D.*m_pend.*cos(THE_Psi).*cos(THE_Phi_pend).*cos(THE_Psi_pend).^2.*cos(THE_Theta_pend).*(2.0./3.0)-(Ly_pend.^2.*THE_Theta_D.*m_pend.*cos(THE_Psi).^2.*cos(THE_Psi_pend).*sin(THE_Psi_pend).*sin(THE_Theta_pend))./1.2e+1+(Ly_pend.^2.*THE_Psi_pend_D.*m_pend.*cos(THE_Psi_pend).*cos(THE_Theta_pend).^2.*sin(THE_Psi).*sin(THE_Psi_pend))./6.0+(Ly_pend.^2.*THE_Theta_pend_D.*m_pend.*cos(THE_Psi_pend).^2.*cos(THE_Theta_pend).*sin(THE_Psi).*sin(THE_Theta_pend))./6.0+(Lz_pend.^2.*THE_Theta_D.*m_pend.*cos(THE_Psi).^2.*cos(THE_Psi_pend).*sin(THE_Psi_pend).*sin(THE_Theta_pend))./3.0-Lz_pend.^2.*THE_Psi_pend_D.*m_pend.*cos(THE_Psi_pend).*cos(THE_Theta_pend).^2.*sin(THE_Psi).*sin(THE_Psi_pend).*(2.0./3.0)-Lz_pend.^2.*THE_Theta_pend_D.*m_pend.*cos(THE_Psi_pend).^2.*cos(THE_Theta_pend).*sin(THE_Psi).*sin(THE_Theta_pend).*(2.0./3.0)+(Lx_pend.^2.*THE_Theta_D.*m_pend.*cos(THE_Psi).^2.*cos(THE_Phi_pend).*cos(THE_Theta_pend).^2.*sin(THE_Phi_pend))./1.2e+1-(Ly_pend.^2.*THE_Theta_D.*m_pend.*cos(THE_Psi).^2.*cos(THE_Phi_pend).*cos(THE_Psi_pend).^2.*sin(THE_Phi_pend))./6.0-(Ly_pend.^2.*THE_Theta_D.*m_pend.*cos(THE_Psi).^2.*cos(THE_Phi_pend).*cos(THE_Theta_pend).^2.*sin(THE_Phi_pend))./1.2e+1+(Ly_pend.^2.*THE_Theta_pend_D.*m_pend.*cos(THE_Psi).*cos(THE_Psi_pend).^2.*cos(THE_Theta_pend).^2.*sin(THE_Phi_pend))./6.0+Lz_pend.^2.*THE_Theta_D.*m_pend.*cos(THE_Psi).^2.*cos(THE_Phi_pend).*cos(THE_Psi_pend).^2.*sin(THE_Phi_pend).*(2.0./3.0)-Lz_pend.^2.*THE_Theta_pend_D.*m_pend.*cos(THE_Psi).*cos(THE_Psi_pend).^2.*cos(THE_Theta_pend).^2.*sin(THE_Phi_pend).*(2.0./3.0)+(Ly_pend.^2.*THE_Psi_D.*m_pend.*cos(THE_Psi).*cos(THE_Phi_pend).^2.*cos(THE_Psi_pend).^2.*cos(THE_Theta_pend).^2)./6.0-Lz_pend.^2.*THE_Psi_D.*m_pend.*cos(THE_Psi).*cos(THE_Phi_pend).^2.*cos(THE_Psi_pend).^2.*cos(THE_Theta_pend).^2.*(2.0./3.0)-(Lx_pend.^2.*THE_Psi_D.*m_pend.*cos(THE_Theta_pend).*sin(THE_Psi).*sin(THE_Phi_pend).*sin(THE_Theta_pend))./6.0+(Ly_pend.^2.*THE_Psi_D.*m_pend.*cos(THE_Theta_pend).*sin(THE_Psi).*sin(THE_Phi_pend).*sin(THE_Theta_pend))./6.0+(Ly_pend.^2.*THE_Theta_D.*m_pend.*cos(THE_Psi).^2.*cos(THE_Phi_pend).^2.*cos(THE_Psi_pend).*sin(THE_Psi_pend).*sin(THE_Theta_pend))./6.0-Lz_pend.^2.*THE_Theta_D.*m_pend.*cos(THE_Psi).^2.*cos(THE_Phi_pend).^2.*cos(THE_Psi_pend).*sin(THE_Psi_pend).*sin(THE_Theta_pend).*(2.0./3.0)+(Lx_pend.^2.*THE_Theta_D.*m_pend.*cos(THE_Psi).*cos(THE_Phi_pend).*cos(THE_Theta_pend).*sin(THE_Psi).*sin(THE_Theta_pend))./1.2e+1-(Ly_pend.^2.*THE_Theta_D.*m_pend.*cos(THE_Psi).*cos(THE_Phi_pend).*cos(THE_Theta_pend).*sin(THE_Psi).*sin(THE_Theta_pend))./1.2e+1+(Ly_pend.^2.*THE_Psi_D.*m_pend.*cos(THE_Phi_pend).*cos(THE_Psi_pend).*cos(THE_Theta_pend).*sin(THE_Psi).*sin(THE_Psi_pend))./6.0+(Ly_pend.^2.*THE_Theta_pend_D.*m_pend.*cos(THE_Psi).*cos(THE_Phi_pend).*cos(THE_Psi_pend).*sin(THE_Psi_pend).*sin(THE_Theta_pend))./6.0-Lz_pend.^2.*THE_Psi_D.*m_pend.*cos(THE_Phi_pend).*cos(THE_Psi_pend).*cos(THE_Theta_pend).*sin(THE_Psi).*sin(THE_Psi_pend).*(2.0./3.0)-Lz_pend.^2.*THE_Theta_pend_D.*m_pend.*cos(THE_Psi).*cos(THE_Phi_pend).*cos(THE_Psi_pend).*sin(THE_Psi_pend).*sin(THE_Theta_pend).*(2.0./3.0)+(Ly_pend.^2.*THE_Theta_D.*m_pend.*cos(THE_Psi).^2.*cos(THE_Phi_pend).*cos(THE_Psi_pend).^2.*cos(THE_Theta_pend).^2.*sin(THE_Phi_pend))./1.2e+1-(Lz_pend.^2.*THE_Theta_D.*m_pend.*cos(THE_Psi).^2.*cos(THE_Phi_pend).*cos(THE_Psi_pend).^2.*cos(THE_Theta_pend).^2.*sin(THE_Phi_pend))./3.0-(Lz_pend.*THE_Theta_D.*Tv_Z_pend.*m_pend.*cos(THE_Psi).*sin(THE_Psi).*sin(THE_Phi_pend).*sin(THE_Psi_pend))./2.0+Lz_pend.*THE_Psi_D.*Tv_Z_pend.*m_pend.*cos(THE_Psi_pend).*sin(THE_Psi).*sin(THE_Phi_pend).*sin(THE_Theta_pend)-(Ly_pend.^2.*THE_Psi_D.*m_pend.*cos(THE_Psi_pend).^2.*cos(THE_Theta_pend).*sin(THE_Psi).*sin(THE_Phi_pend).*sin(THE_Theta_pend))./6.0+Lz_pend.^2.*THE_Psi_D.*m_pend.*cos(THE_Psi_pend).^2.*cos(THE_Theta_pend).*sin(THE_Psi).*sin(THE_Phi_pend).*sin(THE_Theta_pend).*(2.0./3.0)+(Ly_pend.^2.*THE_Theta_D.*m_pend.*cos(THE_Psi).*cos(THE_Psi_pend).*cos(THE_Theta_pend).*sin(THE_Psi).*sin(THE_Phi_pend).*sin(THE_Psi_pend))./1.2e+1-(Ly_pend.^2.*THE_Psi_D.*m_pend.*cos(THE_Psi).*cos(THE_Phi_pend).*cos(THE_Psi_pend).*sin(THE_Phi_pend).*sin(THE_Psi_pend).*sin(THE_Theta_pend))./3.0-(Ly_pend.^2.*THE_Psi_pend_D.*m_pend.*cos(THE_Psi).*cos(THE_Psi_pend).*cos(THE_Theta_pend).*sin(THE_Phi_pend).*sin(THE_Psi_pend).*sin(THE_Theta_pend))./6.0-(Lz_pend.^2.*THE_Theta_D.*m_pend.*cos(THE_Psi).*cos(THE_Psi_pend).*cos(THE_Theta_pend).*sin(THE_Psi).*sin(THE_Phi_pend).*sin(THE_Psi_pend))./3.0+Lz_pend.^2.*THE_Psi_D.*m_pend.*cos(THE_Psi).*cos(THE_Phi_pend).*cos(THE_Psi_pend).*sin(THE_Phi_pend).*sin(THE_Psi_pend).*sin(THE_Theta_pend).*(4.0./3.0)+Lz_pend.^2.*THE_Psi_pend_D.*m_pend.*cos(THE_Psi).*cos(THE_Psi_pend).*cos(THE_Theta_pend).*sin(THE_Phi_pend).*sin(THE_Psi_pend).*sin(THE_Theta_pend).*(2.0./3.0)-(Lz_pend.*THE_Theta_D.*Tv_Z_pend.*m_pend.*cos(THE_Psi).*cos(THE_Phi_pend).*cos(THE_Psi_pend).*sin(THE_Psi).*sin(THE_Theta_pend))./2.0+(Ly_pend.^2.*THE_Theta_D.*m_pend.*cos(THE_Psi).*cos(THE_Phi_pend).*cos(THE_Psi_pend).^2.*cos(THE_Theta_pend).*sin(THE_Psi).*sin(THE_Theta_pend))./1.2e+1-(Lz_pend.^2.*THE_Theta_D.*m_pend.*cos(THE_Psi).*cos(THE_Phi_pend).*cos(THE_Psi_pend).^2.*cos(THE_Theta_pend).*sin(THE_Psi).*sin(THE_Theta_pend))./3.0,